simulink model "new_model"  (R2023a)
(part 3 of 4)

  Bus Selector:RadarSensor:1_OBJ_S_Range_BS/39 -> RadarSensor:1.OBJ_S_Range_39/1  "<OBJ_S_Range_39>"
  Bus Selector:RadarSensor:1_OBJ_S_Range_BS/40 -> RadarSensor:1.OBJ_S_Range_40/1  "<OBJ_S_Range_40>"
  Bus Selector:RadarSensor:1_OBJ_S_Range_BS/41 -> RadarSensor:1.OBJ_S_Range_41/1  "<OBJ_S_Range_41>"
  Bus Selector:RadarSensor:1_OBJ_S_Range_BS/42 -> RadarSensor:1.OBJ_S_Range_42/1  "<OBJ_S_Range_42>"
  Bus Selector:RadarSensor:1_OBJ_S_Range_BS/43 -> RadarSensor:1.OBJ_S_Range_43/1  "<OBJ_S_Range_43>"
  Bus Selector:RadarSensor:1_OBJ_S_Range_BS/44 -> RadarSensor:1.OBJ_S_Range_44/1  "<OBJ_S_Range_44>"
  Bus Selector:RadarSensor:1_OBJ_S_Range_BS/45 -> RadarSensor:1.OBJ_S_Range_45/1  "<OBJ_S_Range_45>"
  Bus Selector:RadarSensor:1_OBJ_S_Range_BS/46 -> RadarSensor:1.OBJ_S_Range_46/1  "<OBJ_S_Range_46>"
  Bus Selector:RadarSensor:1_OBJ_S_Range_BS/47 -> RadarSensor:1.OBJ_S_Range_47/1  "<OBJ_S_Range_47>"
  Bus Selector:RadarSensor:1_OBJ_S_Range_BS/48 -> RadarSensor:1.OBJ_S_Range_48/1  "<OBJ_S_Range_48>"
  Bus Selector:RadarSensor:1_OBJ_S_Range_BS/49 -> RadarSensor:1.OBJ_S_Range_49/1  "<OBJ_S_Range_49>"
  Bus Selector:RadarSensor:1_OBJ_S_Range_BS/50 -> RadarSensor:1.OBJ_S_Range_50/1  "<OBJ_S_Range_50>"
  Bus Selector:RadarSensor:1_OBJ_S_Range_BS/51 -> RadarSensor:1.OBJ_S_Range_51/1  "<OBJ_S_Range_51>"
  Bus Selector:RadarSensor:1_OBJ_S_Range_BS/52 -> RadarSensor:1.OBJ_S_Range_52/1  "<OBJ_S_Range_52>"
  Bus Selector:RadarSensor:1_OBJ_S_Range_BS/53 -> RadarSensor:1.OBJ_S_Range_53/1  "<OBJ_S_Range_53>"
  Bus Selector:RadarSensor:1_OBJ_S_Range_BS/54 -> RadarSensor:1.OBJ_S_Range_54/1  "<OBJ_S_Range_54>"
  Bus Selector:RadarSensor:1_OBJ_S_Range_BS/55 -> RadarSensor:1.OBJ_S_Range_55/1  "<OBJ_S_Range_55>"
  Bus Selector:RadarSensor:1_OBJ_S_Range_BS/56 -> RadarSensor:1.OBJ_S_Range_56/1  "<OBJ_S_Range_56>"
  Bus Selector:RadarSensor:1_OBJ_S_Range_BS/57 -> RadarSensor:1.OBJ_S_Range_57/1  "<OBJ_S_Range_57>"
  Bus Selector:RadarSensor:1_OBJ_S_Range_BS/58 -> RadarSensor:1.OBJ_S_Range_58/1  "<OBJ_S_Range_58>"
  Bus Selector:RadarSensor:1_OBJ_S_Range_BS/59 -> RadarSensor:1.OBJ_S_Range_59/1  "<OBJ_S_Range_59>"
  Bus Selector:RadarSensor:1_OBJ_S_Range_BS/60 -> RadarSensor:1.OBJ_S_Range_60/1  "<OBJ_S_Range_60>"
  Bus Selector:RadarSensor:1_OBJ_S_Range_BS/61 -> RadarSensor:1.OBJ_S_Range_61/1  "<OBJ_S_Range_61>"
  Bus Selector:RadarSensor:1_OBJ_S_Range_BS/62 -> RadarSensor:1.OBJ_S_Range_62/1  "<OBJ_S_Range_62>"
  Bus Selector:RadarSensor:1_OBJ_S_Range_BS/63 -> RadarSensor:1.OBJ_S_Range_63/1  "<OBJ_S_Range_63>"
  Bus Selector:RadarSensor:1_OBJ_S_Range_BS/64 -> RadarSensor:1.OBJ_S_Range_64/1  "<OBJ_S_Range_64>"
  Bus Selector:RadarSensor:1_OBJ_RCS_BS/1 -> RadarSensor:1.OBJ_RCS_1/1  "<OBJ_RCS_1>"
  Bus Selector:RadarSensor:1_OBJ_RCS_BS/2 -> RadarSensor:1.OBJ_RCS_2/1  "<OBJ_RCS_2>"
  Bus Selector:RadarSensor:1_OBJ_RCS_BS/3 -> RadarSensor:1.OBJ_RCS_3/1  "<OBJ_RCS_3>"
  Bus Selector:RadarSensor:1_OBJ_RCS_BS/4 -> RadarSensor:1.OBJ_RCS_4/1  "<OBJ_RCS_4>"
  Bus Selector:RadarSensor:1_OBJ_RCS_BS/5 -> RadarSensor:1.OBJ_RCS_5/1  "<OBJ_RCS_5>"
  Bus Selector:RadarSensor:1_OBJ_RCS_BS/6 -> RadarSensor:1.OBJ_RCS_6/1  "<OBJ_RCS_6>"
  Bus Selector:RadarSensor:1_OBJ_RCS_BS/7 -> RadarSensor:1.OBJ_RCS_7/1  "<OBJ_RCS_7>"
  Bus Selector:RadarSensor:1_OBJ_RCS_BS/8 -> RadarSensor:1.OBJ_RCS_8/1  "<OBJ_RCS_8>"
  Bus Selector:RadarSensor:1_OBJ_RCS_BS/9 -> RadarSensor:1.OBJ_RCS_9/1  "<OBJ_RCS_9>"
  Bus Selector:RadarSensor:1_OBJ_RCS_BS/10 -> RadarSensor:1.OBJ_RCS_10/1  "<OBJ_RCS_10>"
  Bus Selector:RadarSensor:1_OBJ_RCS_BS/11 -> RadarSensor:1.OBJ_RCS_11/1  "<OBJ_RCS_11>"
  Bus Selector:RadarSensor:1_OBJ_RCS_BS/12 -> RadarSensor:1.OBJ_RCS_12/1  "<OBJ_RCS_12>"
  Bus Selector:RadarSensor:1_OBJ_RCS_BS/13 -> RadarSensor:1.OBJ_RCS_13/1  "<OBJ_RCS_13>"
  Bus Selector:RadarSensor:1_OBJ_RCS_BS/14 -> RadarSensor:1.OBJ_RCS_14/1  "<OBJ_RCS_14>"
  Bus Selector:RadarSensor:1_OBJ_RCS_BS/15 -> RadarSensor:1.OBJ_RCS_15/1  "<OBJ_RCS_15>"
  Bus Selector:RadarSensor:1_OBJ_RCS_BS/16 -> RadarSensor:1.OBJ_RCS_16/1  "<OBJ_RCS_16>"
  Bus Selector:RadarSensor:1_OBJ_RCS_BS/17 -> RadarSensor:1.OBJ_RCS_17/1  "<OBJ_RCS_17>"
  Bus Selector:RadarSensor:1_OBJ_RCS_BS/18 -> RadarSensor:1.OBJ_RCS_18/1  "<OBJ_RCS_18>"
  Bus Selector:RadarSensor:1_OBJ_RCS_BS/19 -> RadarSensor:1.OBJ_RCS_19/1  "<OBJ_RCS_19>"
  Bus Selector:RadarSensor:1_OBJ_RCS_BS/20 -> RadarSensor:1.OBJ_RCS_20/1  "<OBJ_RCS_20>"
  Bus Selector:RadarSensor:1_OBJ_RCS_BS/21 -> RadarSensor:1.OBJ_RCS_21/1  "<OBJ_RCS_21>"
  Bus Selector:RadarSensor:1_OBJ_RCS_BS/22 -> RadarSensor:1.OBJ_RCS_22/1  "<OBJ_RCS_22>"
  Bus Selector:RadarSensor:1_OBJ_RCS_BS/23 -> RadarSensor:1.OBJ_RCS_23/1  "<OBJ_RCS_23>"
  Bus Selector:RadarSensor:1_OBJ_RCS_BS/24 -> RadarSensor:1.OBJ_RCS_24/1  "<OBJ_RCS_24>"
  Bus Selector:RadarSensor:1_OBJ_RCS_BS/25 -> RadarSensor:1.OBJ_RCS_25/1  "<OBJ_RCS_25>"
  Bus Selector:RadarSensor:1_OBJ_RCS_BS/26 -> RadarSensor:1.OBJ_RCS_26/1  "<OBJ_RCS_26>"
  Bus Selector:RadarSensor:1_OBJ_RCS_BS/27 -> RadarSensor:1.OBJ_RCS_27/1  "<OBJ_RCS_27>"
  Bus Selector:RadarSensor:1_OBJ_RCS_BS/28 -> RadarSensor:1.OBJ_RCS_28/1  "<OBJ_RCS_28>"
  Bus Selector:RadarSensor:1_OBJ_RCS_BS/29 -> RadarSensor:1.OBJ_RCS_29/1  "<OBJ_RCS_29>"
  Bus Selector:RadarSensor:1_OBJ_RCS_BS/30 -> RadarSensor:1.OBJ_RCS_30/1  "<OBJ_RCS_30>"
  Bus Selector:RadarSensor:1_OBJ_RCS_BS/31 -> RadarSensor:1.OBJ_RCS_31/1  "<OBJ_RCS_31>"
  Bus Selector:RadarSensor:1_OBJ_RCS_BS/32 -> RadarSensor:1.OBJ_RCS_32/1  "<OBJ_RCS_32>"
  Bus Selector:RadarSensor:1_OBJ_RCS_BS/33 -> RadarSensor:1.OBJ_RCS_33/1  "<OBJ_RCS_33>"
  Bus Selector:RadarSensor:1_OBJ_RCS_BS/34 -> RadarSensor:1.OBJ_RCS_34/1  "<OBJ_RCS_34>"
  Bus Selector:RadarSensor:1_OBJ_RCS_BS/35 -> RadarSensor:1.OBJ_RCS_35/1  "<OBJ_RCS_35>"
  Bus Selector:RadarSensor:1_OBJ_RCS_BS/36 -> RadarSensor:1.OBJ_RCS_36/1  "<OBJ_RCS_36>"
  Bus Selector:RadarSensor:1_OBJ_RCS_BS/37 -> RadarSensor:1.OBJ_RCS_37/1  "<OBJ_RCS_37>"
  Bus Selector:RadarSensor:1_OBJ_RCS_BS/38 -> RadarSensor:1.OBJ_RCS_38/1  "<OBJ_RCS_38>"
  Bus Selector:RadarSensor:1_OBJ_RCS_BS/39 -> RadarSensor:1.OBJ_RCS_39/1  "<OBJ_RCS_39>"
  Bus Selector:RadarSensor:1_OBJ_RCS_BS/40 -> RadarSensor:1.OBJ_RCS_40/1  "<OBJ_RCS_40>"
  Bus Selector:RadarSensor:1_OBJ_RCS_BS/41 -> RadarSensor:1.OBJ_RCS_41/1  "<OBJ_RCS_41>"
  Bus Selector:RadarSensor:1_OBJ_RCS_BS/42 -> RadarSensor:1.OBJ_RCS_42/1  "<OBJ_RCS_42>"
  Bus Selector:RadarSensor:1_OBJ_RCS_BS/43 -> RadarSensor:1.OBJ_RCS_43/1  "<OBJ_RCS_43>"
  Bus Selector:RadarSensor:1_OBJ_RCS_BS/44 -> RadarSensor:1.OBJ_RCS_44/1  "<OBJ_RCS_44>"
  Bus Selector:RadarSensor:1_OBJ_RCS_BS/45 -> RadarSensor:1.OBJ_RCS_45/1  "<OBJ_RCS_45>"
  Bus Selector:RadarSensor:1_OBJ_RCS_BS/46 -> RadarSensor:1.OBJ_RCS_46/1  "<OBJ_RCS_46>"
  Bus Selector:RadarSensor:1_OBJ_RCS_BS/47 -> RadarSensor:1.OBJ_RCS_47/1  "<OBJ_RCS_47>"
  Bus Selector:RadarSensor:1_OBJ_RCS_BS/48 -> RadarSensor:1.OBJ_RCS_48/1  "<OBJ_RCS_48>"
  Bus Selector:RadarSensor:1_OBJ_RCS_BS/49 -> RadarSensor:1.OBJ_RCS_49/1  "<OBJ_RCS_49>"
  Bus Selector:RadarSensor:1_OBJ_RCS_BS/50 -> RadarSensor:1.OBJ_RCS_50/1  "<OBJ_RCS_50>"
  Bus Selector:RadarSensor:1_OBJ_RCS_BS/51 -> RadarSensor:1.OBJ_RCS_51/1  "<OBJ_RCS_51>"
  Bus Selector:RadarSensor:1_OBJ_RCS_BS/52 -> RadarSensor:1.OBJ_RCS_52/1  "<OBJ_RCS_52>"
  Bus Selector:RadarSensor:1_OBJ_RCS_BS/53 -> RadarSensor:1.OBJ_RCS_53/1  "<OBJ_RCS_53>"
  Bus Selector:RadarSensor:1_OBJ_RCS_BS/54 -> RadarSensor:1.OBJ_RCS_54/1  "<OBJ_RCS_54>"
  Bus Selector:RadarSensor:1_OBJ_RCS_BS/55 -> RadarSensor:1.OBJ_RCS_55/1  "<OBJ_RCS_55>"
  Bus Selector:RadarSensor:1_OBJ_RCS_BS/56 -> RadarSensor:1.OBJ_RCS_56/1  "<OBJ_RCS_56>"
  Bus Selector:RadarSensor:1_OBJ_RCS_BS/57 -> RadarSensor:1.OBJ_RCS_57/1  "<OBJ_RCS_57>"
  Bus Selector:RadarSensor:1_OBJ_RCS_BS/58 -> RadarSensor:1.OBJ_RCS_58/1  "<OBJ_RCS_58>"
  Bus Selector:RadarSensor:1_OBJ_RCS_BS/59 -> RadarSensor:1.OBJ_RCS_59/1  "<OBJ_RCS_59>"
  Bus Selector:RadarSensor:1_OBJ_RCS_BS/60 -> RadarSensor:1.OBJ_RCS_60/1  "<OBJ_RCS_60>"
  Bus Selector:RadarSensor:1_OBJ_RCS_BS/61 -> RadarSensor:1.OBJ_RCS_61/1  "<OBJ_RCS_61>"
  Bus Selector:RadarSensor:1_OBJ_RCS_BS/62 -> RadarSensor:1.OBJ_RCS_62/1  "<OBJ_RCS_62>"
  Bus Selector:RadarSensor:1_OBJ_RCS_BS/63 -> RadarSensor:1.OBJ_RCS_63/1  "<OBJ_RCS_63>"
  Bus Selector:RadarSensor:1_OBJ_RCS_BS/64 -> RadarSensor:1.OBJ_RCS_64/1  "<OBJ_RCS_64>"
  Bus Selector:RadarSensor:1/1 -> RadarSensor:1.time/1  "<time>"
  Bus Selector:RadarSensor:1/2 -> RadarSensor:1.width/1  "<width>"
  Bus Selector:RadarSensor:1/3 -> RadarSensor:1.OBJ_ID/1, Bus Selector:RadarSensor:1_OBJ_ID_BS/1  "<OBJ_ID>"
  Bus Selector:RadarSensor:1/4 -> RadarSensor:1.OBJ_Class/1, Bus Selector:RadarSensor:1_OBJ_Class_BS/1  "<OBJ_Class>"
  Bus Selector:RadarSensor:1/5 -> RadarSensor:1.OBJ_S_Azimuth/1, Bus Selector:RadarSensor:1_OBJ_S_Azimuth_BS/1  "<OBJ_S_Azimuth>"
  Bus Selector:RadarSensor:1/6 -> RadarSensor:1.OBJ_S_Elevation/1, Bus Selector:RadarSensor:1_OBJ_S_Elevation_BS/1  "<OBJ_S_Elevation>"
  Bus Selector:RadarSensor:1/7 -> RadarSensor:1.OBJ_S_Velocity/1, Bus Selector:RadarSensor:1_OBJ_S_Velocity_BS/1  "<OBJ_S_Velocity>"
  Bus Selector:RadarSensor:1/8 -> RadarSensor:1.OBJ_S_Range/1, Bus Selector:RadarSensor:1_OBJ_S_Range_BS/1  "<OBJ_S_Range>"
  Bus Selector:RadarSensor:1/9 -> RadarSensor:1.OBJ_RCS/1, Bus Selector:RadarSensor:1_OBJ_RCS_BS/1  "<OBJ_RCS>"
  Bus Selector:RadarSensor:2_OBJ_ID_BS/1 -> RadarSensor:2.OBJ_ID_1/1  "<OBJ_ID_1>"
  Bus Selector:RadarSensor:2_OBJ_ID_BS/2 -> RadarSensor:2.OBJ_ID_2/1  "<OBJ_ID_2>"
  Bus Selector:RadarSensor:2_OBJ_ID_BS/3 -> RadarSensor:2.OBJ_ID_3/1  "<OBJ_ID_3>"
  Bus Selector:RadarSensor:2_OBJ_ID_BS/4 -> RadarSensor:2.OBJ_ID_4/1  "<OBJ_ID_4>"
  Bus Selector:RadarSensor:2_OBJ_ID_BS/5 -> RadarSensor:2.OBJ_ID_5/1  "<OBJ_ID_5>"
  Bus Selector:RadarSensor:2_OBJ_ID_BS/6 -> RadarSensor:2.OBJ_ID_6/1  "<OBJ_ID_6>"
  Bus Selector:RadarSensor:2_OBJ_ID_BS/7 -> RadarSensor:2.OBJ_ID_7/1  "<OBJ_ID_7>"
  Bus Selector:RadarSensor:2_OBJ_ID_BS/8 -> RadarSensor:2.OBJ_ID_8/1  "<OBJ_ID_8>"
  Bus Selector:RadarSensor:2_OBJ_ID_BS/9 -> RadarSensor:2.OBJ_ID_9/1  "<OBJ_ID_9>"
  Bus Selector:RadarSensor:2_OBJ_ID_BS/10 -> RadarSensor:2.OBJ_ID_10/1  "<OBJ_ID_10>"
  Bus Selector:RadarSensor:2_OBJ_ID_BS/11 -> RadarSensor:2.OBJ_ID_11/1  "<OBJ_ID_11>"
  Bus Selector:RadarSensor:2_OBJ_ID_BS/12 -> RadarSensor:2.OBJ_ID_12/1  "<OBJ_ID_12>"
  Bus Selector:RadarSensor:2_OBJ_ID_BS/13 -> RadarSensor:2.OBJ_ID_13/1  "<OBJ_ID_13>"
  Bus Selector:RadarSensor:2_OBJ_ID_BS/14 -> RadarSensor:2.OBJ_ID_14/1  "<OBJ_ID_14>"
  Bus Selector:RadarSensor:2_OBJ_ID_BS/15 -> RadarSensor:2.OBJ_ID_15/1  "<OBJ_ID_15>"
  Bus Selector:RadarSensor:2_OBJ_ID_BS/16 -> RadarSensor:2.OBJ_ID_16/1  "<OBJ_ID_16>"
  Bus Selector:RadarSensor:2_OBJ_ID_BS/17 -> RadarSensor:2.OBJ_ID_17/1  "<OBJ_ID_17>"
  Bus Selector:RadarSensor:2_OBJ_ID_BS/18 -> RadarSensor:2.OBJ_ID_18/1  "<OBJ_ID_18>"
  Bus Selector:RadarSensor:2_OBJ_ID_BS/19 -> RadarSensor:2.OBJ_ID_19/1  "<OBJ_ID_19>"
  Bus Selector:RadarSensor:2_OBJ_ID_BS/20 -> RadarSensor:2.OBJ_ID_20/1  "<OBJ_ID_20>"
  Bus Selector:RadarSensor:2_OBJ_ID_BS/21 -> RadarSensor:2.OBJ_ID_21/1  "<OBJ_ID_21>"
  Bus Selector:RadarSensor:2_OBJ_ID_BS/22 -> RadarSensor:2.OBJ_ID_22/1  "<OBJ_ID_22>"
  Bus Selector:RadarSensor:2_OBJ_ID_BS/23 -> RadarSensor:2.OBJ_ID_23/1  "<OBJ_ID_23>"
  Bus Selector:RadarSensor:2_OBJ_ID_BS/24 -> RadarSensor:2.OBJ_ID_24/1  "<OBJ_ID_24>"
  Bus Selector:RadarSensor:2_OBJ_ID_BS/25 -> RadarSensor:2.OBJ_ID_25/1  "<OBJ_ID_25>"
  Bus Selector:RadarSensor:2_OBJ_ID_BS/26 -> RadarSensor:2.OBJ_ID_26/1  "<OBJ_ID_26>"
  Bus Selector:RadarSensor:2_OBJ_ID_BS/27 -> RadarSensor:2.OBJ_ID_27/1  "<OBJ_ID_27>"
  Bus Selector:RadarSensor:2_OBJ_ID_BS/28 -> RadarSensor:2.OBJ_ID_28/1  "<OBJ_ID_28>"
  Bus Selector:RadarSensor:2_OBJ_ID_BS/29 -> RadarSensor:2.OBJ_ID_29/1  "<OBJ_ID_29>"
  Bus Selector:RadarSensor:2_OBJ_ID_BS/30 -> RadarSensor:2.OBJ_ID_30/1  "<OBJ_ID_30>"
  Bus Selector:RadarSensor:2_OBJ_ID_BS/31 -> RadarSensor:2.OBJ_ID_31/1  "<OBJ_ID_31>"
  Bus Selector:RadarSensor:2_OBJ_ID_BS/32 -> RadarSensor:2.OBJ_ID_32/1  "<OBJ_ID_32>"
  Bus Selector:RadarSensor:2_OBJ_ID_BS/33 -> RadarSensor:2.OBJ_ID_33/1  "<OBJ_ID_33>"
  Bus Selector:RadarSensor:2_OBJ_ID_BS/34 -> RadarSensor:2.OBJ_ID_34/1  "<OBJ_ID_34>"
  Bus Selector:RadarSensor:2_OBJ_ID_BS/35 -> RadarSensor:2.OBJ_ID_35/1  "<OBJ_ID_35>"
  Bus Selector:RadarSensor:2_OBJ_ID_BS/36 -> RadarSensor:2.OBJ_ID_36/1  "<OBJ_ID_36>"
  Bus Selector:RadarSensor:2_OBJ_ID_BS/37 -> RadarSensor:2.OBJ_ID_37/1  "<OBJ_ID_37>"
  Bus Selector:RadarSensor:2_OBJ_ID_BS/38 -> RadarSensor:2.OBJ_ID_38/1  "<OBJ_ID_38>"
  Bus Selector:RadarSensor:2_OBJ_ID_BS/39 -> RadarSensor:2.OBJ_ID_39/1  "<OBJ_ID_39>"
  Bus Selector:RadarSensor:2_OBJ_ID_BS/40 -> RadarSensor:2.OBJ_ID_40/1  "<OBJ_ID_40>"
  Bus Selector:RadarSensor:2_OBJ_ID_BS/41 -> RadarSensor:2.OBJ_ID_41/1  "<OBJ_ID_41>"
  Bus Selector:RadarSensor:2_OBJ_ID_BS/42 -> RadarSensor:2.OBJ_ID_42/1  "<OBJ_ID_42>"
  Bus Selector:RadarSensor:2_OBJ_ID_BS/43 -> RadarSensor:2.OBJ_ID_43/1  "<OBJ_ID_43>"
  Bus Selector:RadarSensor:2_OBJ_ID_BS/44 -> RadarSensor:2.OBJ_ID_44/1  "<OBJ_ID_44>"
  Bus Selector:RadarSensor:2_OBJ_ID_BS/45 -> RadarSensor:2.OBJ_ID_45/1  "<OBJ_ID_45>"
  Bus Selector:RadarSensor:2_OBJ_ID_BS/46 -> RadarSensor:2.OBJ_ID_46/1  "<OBJ_ID_46>"
  Bus Selector:RadarSensor:2_OBJ_ID_BS/47 -> RadarSensor:2.OBJ_ID_47/1  "<OBJ_ID_47>"
  Bus Selector:RadarSensor:2_OBJ_ID_BS/48 -> RadarSensor:2.OBJ_ID_48/1  "<OBJ_ID_48>"
  Bus Selector:RadarSensor:2_OBJ_ID_BS/49 -> RadarSensor:2.OBJ_ID_49/1  "<OBJ_ID_49>"
  Bus Selector:RadarSensor:2_OBJ_ID_BS/50 -> RadarSensor:2.OBJ_ID_50/1  "<OBJ_ID_50>"
  Bus Selector:RadarSensor:2_OBJ_ID_BS/51 -> RadarSensor:2.OBJ_ID_51/1  "<OBJ_ID_51>"
  Bus Selector:RadarSensor:2_OBJ_ID_BS/52 -> RadarSensor:2.OBJ_ID_52/1  "<OBJ_ID_52>"
  Bus Selector:RadarSensor:2_OBJ_ID_BS/53 -> RadarSensor:2.OBJ_ID_53/1  "<OBJ_ID_53>"
  Bus Selector:RadarSensor:2_OBJ_ID_BS/54 -> RadarSensor:2.OBJ_ID_54/1  "<OBJ_ID_54>"
  Bus Selector:RadarSensor:2_OBJ_ID_BS/55 -> RadarSensor:2.OBJ_ID_55/1  "<OBJ_ID_55>"
  Bus Selector:RadarSensor:2_OBJ_ID_BS/56 -> RadarSensor:2.OBJ_ID_56/1  "<OBJ_ID_56>"
  Bus Selector:RadarSensor:2_OBJ_ID_BS/57 -> RadarSensor:2.OBJ_ID_57/1  "<OBJ_ID_57>"
  Bus Selector:RadarSensor:2_OBJ_ID_BS/58 -> RadarSensor:2.OBJ_ID_58/1  "<OBJ_ID_58>"
  Bus Selector:RadarSensor:2_OBJ_ID_BS/59 -> RadarSensor:2.OBJ_ID_59/1  "<OBJ_ID_59>"
  Bus Selector:RadarSensor:2_OBJ_ID_BS/60 -> RadarSensor:2.OBJ_ID_60/1  "<OBJ_ID_60>"
  Bus Selector:RadarSensor:2_OBJ_ID_BS/61 -> RadarSensor:2.OBJ_ID_61/1  "<OBJ_ID_61>"
  Bus Selector:RadarSensor:2_OBJ_ID_BS/62 -> RadarSensor:2.OBJ_ID_62/1  "<OBJ_ID_62>"
  Bus Selector:RadarSensor:2_OBJ_ID_BS/63 -> RadarSensor:2.OBJ_ID_63/1  "<OBJ_ID_63>"
  Bus Selector:RadarSensor:2_OBJ_ID_BS/64 -> RadarSensor:2.OBJ_ID_64/1  "<OBJ_ID_64>"
  Bus Selector:RadarSensor:2_OBJ_Class_BS/1 -> RadarSensor:2.OBJ_Class_1/1  "<OBJ_Class_1>"
  Bus Selector:RadarSensor:2_OBJ_Class_BS/2 -> RadarSensor:2.OBJ_Class_2/1  "<OBJ_Class_2>"
  Bus Selector:RadarSensor:2_OBJ_Class_BS/3 -> RadarSensor:2.OBJ_Class_3/1  "<OBJ_Class_3>"
  Bus Selector:RadarSensor:2_OBJ_Class_BS/4 -> RadarSensor:2.OBJ_Class_4/1  "<OBJ_Class_4>"
  Bus Selector:RadarSensor:2_OBJ_Class_BS/5 -> RadarSensor:2.OBJ_Class_5/1  "<OBJ_Class_5>"
  Bus Selector:RadarSensor:2_OBJ_Class_BS/6 -> RadarSensor:2.OBJ_Class_6/1  "<OBJ_Class_6>"
  Bus Selector:RadarSensor:2_OBJ_Class_BS/7 -> RadarSensor:2.OBJ_Class_7/1  "<OBJ_Class_7>"
  Bus Selector:RadarSensor:2_OBJ_Class_BS/8 -> RadarSensor:2.OBJ_Class_8/1  "<OBJ_Class_8>"
  Bus Selector:RadarSensor:2_OBJ_Class_BS/9 -> RadarSensor:2.OBJ_Class_9/1  "<OBJ_Class_9>"
  Bus Selector:RadarSensor:2_OBJ_Class_BS/10 -> RadarSensor:2.OBJ_Class_10/1  "<OBJ_Class_10>"
  Bus Selector:RadarSensor:2_OBJ_Class_BS/11 -> RadarSensor:2.OBJ_Class_11/1  "<OBJ_Class_11>"
  Bus Selector:RadarSensor:2_OBJ_Class_BS/12 -> RadarSensor:2.OBJ_Class_12/1  "<OBJ_Class_12>"
  Bus Selector:RadarSensor:2_OBJ_Class_BS/13 -> RadarSensor:2.OBJ_Class_13/1  "<OBJ_Class_13>"
  Bus Selector:RadarSensor:2_OBJ_Class_BS/14 -> RadarSensor:2.OBJ_Class_14/1  "<OBJ_Class_14>"
  Bus Selector:RadarSensor:2_OBJ_Class_BS/15 -> RadarSensor:2.OBJ_Class_15/1  "<OBJ_Class_15>"
  Bus Selector:RadarSensor:2_OBJ_Class_BS/16 -> RadarSensor:2.OBJ_Class_16/1  "<OBJ_Class_16>"
  Bus Selector:RadarSensor:2_OBJ_Class_BS/17 -> RadarSensor:2.OBJ_Class_17/1  "<OBJ_Class_17>"
  Bus Selector:RadarSensor:2_OBJ_Class_BS/18 -> RadarSensor:2.OBJ_Class_18/1  "<OBJ_Class_18>"
  Bus Selector:RadarSensor:2_OBJ_Class_BS/19 -> RadarSensor:2.OBJ_Class_19/1  "<OBJ_Class_19>"
  Bus Selector:RadarSensor:2_OBJ_Class_BS/20 -> RadarSensor:2.OBJ_Class_20/1  "<OBJ_Class_20>"
  Bus Selector:RadarSensor:2_OBJ_Class_BS/21 -> RadarSensor:2.OBJ_Class_21/1  "<OBJ_Class_21>"
  Bus Selector:RadarSensor:2_OBJ_Class_BS/22 -> RadarSensor:2.OBJ_Class_22/1  "<OBJ_Class_22>"
  Bus Selector:RadarSensor:2_OBJ_Class_BS/23 -> RadarSensor:2.OBJ_Class_23/1  "<OBJ_Class_23>"
  Bus Selector:RadarSensor:2_OBJ_Class_BS/24 -> RadarSensor:2.OBJ_Class_24/1  "<OBJ_Class_24>"
  Bus Selector:RadarSensor:2_OBJ_Class_BS/25 -> RadarSensor:2.OBJ_Class_25/1  "<OBJ_Class_25>"
  Bus Selector:RadarSensor:2_OBJ_Class_BS/26 -> RadarSensor:2.OBJ_Class_26/1  "<OBJ_Class_26>"
  Bus Selector:RadarSensor:2_OBJ_Class_BS/27 -> RadarSensor:2.OBJ_Class_27/1  "<OBJ_Class_27>"
  Bus Selector:RadarSensor:2_OBJ_Class_BS/28 -> RadarSensor:2.OBJ_Class_28/1  "<OBJ_Class_28>"
  Bus Selector:RadarSensor:2_OBJ_Class_BS/29 -> RadarSensor:2.OBJ_Class_29/1  "<OBJ_Class_29>"
  Bus Selector:RadarSensor:2_OBJ_Class_BS/30 -> RadarSensor:2.OBJ_Class_30/1  "<OBJ_Class_30>"
  Bus Selector:RadarSensor:2_OBJ_Class_BS/31 -> RadarSensor:2.OBJ_Class_31/1  "<OBJ_Class_31>"
  Bus Selector:RadarSensor:2_OBJ_Class_BS/32 -> RadarSensor:2.OBJ_Class_32/1  "<OBJ_Class_32>"
  Bus Selector:RadarSensor:2_OBJ_Class_BS/33 -> RadarSensor:2.OBJ_Class_33/1  "<OBJ_Class_33>"
  Bus Selector:RadarSensor:2_OBJ_Class_BS/34 -> RadarSensor:2.OBJ_Class_34/1  "<OBJ_Class_34>"
  Bus Selector:RadarSensor:2_OBJ_Class_BS/35 -> RadarSensor:2.OBJ_Class_35/1  "<OBJ_Class_35>"
  Bus Selector:RadarSensor:2_OBJ_Class_BS/36 -> RadarSensor:2.OBJ_Class_36/1  "<OBJ_Class_36>"
  Bus Selector:RadarSensor:2_OBJ_Class_BS/37 -> RadarSensor:2.OBJ_Class_37/1  "<OBJ_Class_37>"
  Bus Selector:RadarSensor:2_OBJ_Class_BS/38 -> RadarSensor:2.OBJ_Class_38/1  "<OBJ_Class_38>"
  Bus Selector:RadarSensor:2_OBJ_Class_BS/39 -> RadarSensor:2.OBJ_Class_39/1  "<OBJ_Class_39>"
  Bus Selector:RadarSensor:2_OBJ_Class_BS/40 -> RadarSensor:2.OBJ_Class_40/1  "<OBJ_Class_40>"
  Bus Selector:RadarSensor:2_OBJ_Class_BS/41 -> RadarSensor:2.OBJ_Class_41/1  "<OBJ_Class_41>"
  Bus Selector:RadarSensor:2_OBJ_Class_BS/42 -> RadarSensor:2.OBJ_Class_42/1  "<OBJ_Class_42>"
  Bus Selector:RadarSensor:2_OBJ_Class_BS/43 -> RadarSensor:2.OBJ_Class_43/1  "<OBJ_Class_43>"
  Bus Selector:RadarSensor:2_OBJ_Class_BS/44 -> RadarSensor:2.OBJ_Class_44/1  "<OBJ_Class_44>"
  Bus Selector:RadarSensor:2_OBJ_Class_BS/45 -> RadarSensor:2.OBJ_Class_45/1  "<OBJ_Class_45>"
  Bus Selector:RadarSensor:2_OBJ_Class_BS/46 -> RadarSensor:2.OBJ_Class_46/1  "<OBJ_Class_46>"
  Bus Selector:RadarSensor:2_OBJ_Class_BS/47 -> RadarSensor:2.OBJ_Class_47/1  "<OBJ_Class_47>"
  Bus Selector:RadarSensor:2_OBJ_Class_BS/48 -> RadarSensor:2.OBJ_Class_48/1  "<OBJ_Class_48>"
  Bus Selector:RadarSensor:2_OBJ_Class_BS/49 -> RadarSensor:2.OBJ_Class_49/1  "<OBJ_Class_49>"
  Bus Selector:RadarSensor:2_OBJ_Class_BS/50 -> RadarSensor:2.OBJ_Class_50/1  "<OBJ_Class_50>"
  Bus Selector:RadarSensor:2_OBJ_Class_BS/51 -> RadarSensor:2.OBJ_Class_51/1  "<OBJ_Class_51>"
  Bus Selector:RadarSensor:2_OBJ_Class_BS/52 -> RadarSensor:2.OBJ_Class_52/1  "<OBJ_Class_52>"
  Bus Selector:RadarSensor:2_OBJ_Class_BS/53 -> RadarSensor:2.OBJ_Class_53/1  "<OBJ_Class_53>"
  Bus Selector:RadarSensor:2_OBJ_Class_BS/54 -> RadarSensor:2.OBJ_Class_54/1  "<OBJ_Class_54>"
  Bus Selector:RadarSensor:2_OBJ_Class_BS/55 -> RadarSensor:2.OBJ_Class_55/1  "<OBJ_Class_55>"
  Bus Selector:RadarSensor:2_OBJ_Class_BS/56 -> RadarSensor:2.OBJ_Class_56/1  "<OBJ_Class_56>"
  Bus Selector:RadarSensor:2_OBJ_Class_BS/57 -> RadarSensor:2.OBJ_Class_57/1  "<OBJ_Class_57>"
  Bus Selector:RadarSensor:2_OBJ_Class_BS/58 -> RadarSensor:2.OBJ_Class_58/1  "<OBJ_Class_58>"
  Bus Selector:RadarSensor:2_OBJ_Class_BS/59 -> RadarSensor:2.OBJ_Class_59/1  "<OBJ_Class_59>"
  Bus Selector:RadarSensor:2_OBJ_Class_BS/60 -> RadarSensor:2.OBJ_Class_60/1  "<OBJ_Class_60>"
  Bus Selector:RadarSensor:2_OBJ_Class_BS/61 -> RadarSensor:2.OBJ_Class_61/1  "<OBJ_Class_61>"
  Bus Selector:RadarSensor:2_OBJ_Class_BS/62 -> RadarSensor:2.OBJ_Class_62/1  "<OBJ_Class_62>"
  Bus Selector:RadarSensor:2_OBJ_Class_BS/63 -> RadarSensor:2.OBJ_Class_63/1  "<OBJ_Class_63>"
  Bus Selector:RadarSensor:2_OBJ_Class_BS/64 -> RadarSensor:2.OBJ_Class_64/1  "<OBJ_Class_64>"
  Bus Selector:RadarSensor:2_OBJ_S_Azimuth_BS/1 -> RadarSensor:2.OBJ_S_Azimuth_1/1  "<OBJ_S_Azimuth_1>"
  Bus Selector:RadarSensor:2_OBJ_S_Azimuth_BS/2 -> RadarSensor:2.OBJ_S_Azimuth_2/1  "<OBJ_S_Azimuth_2>"
  Bus Selector:RadarSensor:2_OBJ_S_Azimuth_BS/3 -> RadarSensor:2.OBJ_S_Azimuth_3/1  "<OBJ_S_Azimuth_3>"
  Bus Selector:RadarSensor:2_OBJ_S_Azimuth_BS/4 -> RadarSensor:2.OBJ_S_Azimuth_4/1  "<OBJ_S_Azimuth_4>"
  Bus Selector:RadarSensor:2_OBJ_S_Azimuth_BS/5 -> RadarSensor:2.OBJ_S_Azimuth_5/1  "<OBJ_S_Azimuth_5>"
  Bus Selector:RadarSensor:2_OBJ_S_Azimuth_BS/6 -> RadarSensor:2.OBJ_S_Azimuth_6/1  "<OBJ_S_Azimuth_6>"
  Bus Selector:RadarSensor:2_OBJ_S_Azimuth_BS/7 -> RadarSensor:2.OBJ_S_Azimuth_7/1  "<OBJ_S_Azimuth_7>"
  Bus Selector:RadarSensor:2_OBJ_S_Azimuth_BS/8 -> RadarSensor:2.OBJ_S_Azimuth_8/1  "<OBJ_S_Azimuth_8>"
  Bus Selector:RadarSensor:2_OBJ_S_Azimuth_BS/9 -> RadarSensor:2.OBJ_S_Azimuth_9/1  "<OBJ_S_Azimuth_9>"
  Bus Selector:RadarSensor:2_OBJ_S_Azimuth_BS/10 -> RadarSensor:2.OBJ_S_Azimuth_10/1  "<OBJ_S_Azimuth_10>"
  Bus Selector:RadarSensor:2_OBJ_S_Azimuth_BS/11 -> RadarSensor:2.OBJ_S_Azimuth_11/1  "<OBJ_S_Azimuth_11>"
  Bus Selector:RadarSensor:2_OBJ_S_Azimuth_BS/12 -> RadarSensor:2.OBJ_S_Azimuth_12/1  "<OBJ_S_Azimuth_12>"
  Bus Selector:RadarSensor:2_OBJ_S_Azimuth_BS/13 -> RadarSensor:2.OBJ_S_Azimuth_13/1  "<OBJ_S_Azimuth_13>"
  Bus Selector:RadarSensor:2_OBJ_S_Azimuth_BS/14 -> RadarSensor:2.OBJ_S_Azimuth_14/1  "<OBJ_S_Azimuth_14>"
  Bus Selector:RadarSensor:2_OBJ_S_Azimuth_BS/15 -> RadarSensor:2.OBJ_S_Azimuth_15/1  "<OBJ_S_Azimuth_15>"
  Bus Selector:RadarSensor:2_OBJ_S_Azimuth_BS/16 -> RadarSensor:2.OBJ_S_Azimuth_16/1  "<OBJ_S_Azimuth_16>"
  Bus Selector:RadarSensor:2_OBJ_S_Azimuth_BS/17 -> RadarSensor:2.OBJ_S_Azimuth_17/1  "<OBJ_S_Azimuth_17>"
  Bus Selector:RadarSensor:2_OBJ_S_Azimuth_BS/18 -> RadarSensor:2.OBJ_S_Azimuth_18/1  "<OBJ_S_Azimuth_18>"
  Bus Selector:RadarSensor:2_OBJ_S_Azimuth_BS/19 -> RadarSensor:2.OBJ_S_Azimuth_19/1  "<OBJ_S_Azimuth_19>"
  Bus Selector:RadarSensor:2_OBJ_S_Azimuth_BS/20 -> RadarSensor:2.OBJ_S_Azimuth_20/1  "<OBJ_S_Azimuth_20>"
  Bus Selector:RadarSensor:2_OBJ_S_Azimuth_BS/21 -> RadarSensor:2.OBJ_S_Azimuth_21/1  "<OBJ_S_Azimuth_21>"
  Bus Selector:RadarSensor:2_OBJ_S_Azimuth_BS/22 -> RadarSensor:2.OBJ_S_Azimuth_22/1  "<OBJ_S_Azimuth_22>"
  Bus Selector:RadarSensor:2_OBJ_S_Azimuth_BS/23 -> RadarSensor:2.OBJ_S_Azimuth_23/1  "<OBJ_S_Azimuth_23>"
  Bus Selector:RadarSensor:2_OBJ_S_Azimuth_BS/24 -> RadarSensor:2.OBJ_S_Azimuth_24/1  "<OBJ_S_Azimuth_24>"
  Bus Selector:RadarSensor:2_OBJ_S_Azimuth_BS/25 -> RadarSensor:2.OBJ_S_Azimuth_25/1  "<OBJ_S_Azimuth_25>"
  Bus Selector:RadarSensor:2_OBJ_S_Azimuth_BS/26 -> RadarSensor:2.OBJ_S_Azimuth_26/1  "<OBJ_S_Azimuth_26>"
  Bus Selector:RadarSensor:2_OBJ_S_Azimuth_BS/27 -> RadarSensor:2.OBJ_S_Azimuth_27/1  "<OBJ_S_Azimuth_27>"
  Bus Selector:RadarSensor:2_OBJ_S_Azimuth_BS/28 -> RadarSensor:2.OBJ_S_Azimuth_28/1  "<OBJ_S_Azimuth_28>"
  Bus Selector:RadarSensor:2_OBJ_S_Azimuth_BS/29 -> RadarSensor:2.OBJ_S_Azimuth_29/1  "<OBJ_S_Azimuth_29>"
  Bus Selector:RadarSensor:2_OBJ_S_Azimuth_BS/30 -> RadarSensor:2.OBJ_S_Azimuth_30/1  "<OBJ_S_Azimuth_30>"
  Bus Selector:RadarSensor:2_OBJ_S_Azimuth_BS/31 -> RadarSensor:2.OBJ_S_Azimuth_31/1  "<OBJ_S_Azimuth_31>"
  Bus Selector:RadarSensor:2_OBJ_S_Azimuth_BS/32 -> RadarSensor:2.OBJ_S_Azimuth_32/1  "<OBJ_S_Azimuth_32>"
  Bus Selector:RadarSensor:2_OBJ_S_Azimuth_BS/33 -> RadarSensor:2.OBJ_S_Azimuth_33/1  "<OBJ_S_Azimuth_33>"
  Bus Selector:RadarSensor:2_OBJ_S_Azimuth_BS/34 -> RadarSensor:2.OBJ_S_Azimuth_34/1  "<OBJ_S_Azimuth_34>"
  Bus Selector:RadarSensor:2_OBJ_S_Azimuth_BS/35 -> RadarSensor:2.OBJ_S_Azimuth_35/1  "<OBJ_S_Azimuth_35>"
  Bus Selector:RadarSensor:2_OBJ_S_Azimuth_BS/36 -> RadarSensor:2.OBJ_S_Azimuth_36/1  "<OBJ_S_Azimuth_36>"
  Bus Selector:RadarSensor:2_OBJ_S_Azimuth_BS/37 -> RadarSensor:2.OBJ_S_Azimuth_37/1  "<OBJ_S_Azimuth_37>"
  Bus Selector:RadarSensor:2_OBJ_S_Azimuth_BS/38 -> RadarSensor:2.OBJ_S_Azimuth_38/1  "<OBJ_S_Azimuth_38>"
  Bus Selector:RadarSensor:2_OBJ_S_Azimuth_BS/39 -> RadarSensor:2.OBJ_S_Azimuth_39/1  "<OBJ_S_Azimuth_39>"
  Bus Selector:RadarSensor:2_OBJ_S_Azimuth_BS/40 -> RadarSensor:2.OBJ_S_Azimuth_40/1  "<OBJ_S_Azimuth_40>"
  Bus Selector:RadarSensor:2_OBJ_S_Azimuth_BS/41 -> RadarSensor:2.OBJ_S_Azimuth_41/1  "<OBJ_S_Azimuth_41>"
  Bus Selector:RadarSensor:2_OBJ_S_Azimuth_BS/42 -> RadarSensor:2.OBJ_S_Azimuth_42/1  "<OBJ_S_Azimuth_42>"
  Bus Selector:RadarSensor:2_OBJ_S_Azimuth_BS/43 -> RadarSensor:2.OBJ_S_Azimuth_43/1  "<OBJ_S_Azimuth_43>"
  Bus Selector:RadarSensor:2_OBJ_S_Azimuth_BS/44 -> RadarSensor:2.OBJ_S_Azimuth_44/1  "<OBJ_S_Azimuth_44>"
  Bus Selector:RadarSensor:2_OBJ_S_Azimuth_BS/45 -> RadarSensor:2.OBJ_S_Azimuth_45/1  "<OBJ_S_Azimuth_45>"
  Bus Selector:RadarSensor:2_OBJ_S_Azimuth_BS/46 -> RadarSensor:2.OBJ_S_Azimuth_46/1  "<OBJ_S_Azimuth_46>"
  Bus Selector:RadarSensor:2_OBJ_S_Azimuth_BS/47 -> RadarSensor:2.OBJ_S_Azimuth_47/1  "<OBJ_S_Azimuth_47>"
  Bus Selector:RadarSensor:2_OBJ_S_Azimuth_BS/48 -> RadarSensor:2.OBJ_S_Azimuth_48/1  "<OBJ_S_Azimuth_48>"
  Bus Selector:RadarSensor:2_OBJ_S_Azimuth_BS/49 -> RadarSensor:2.OBJ_S_Azimuth_49/1  "<OBJ_S_Azimuth_49>"
  Bus Selector:RadarSensor:2_OBJ_S_Azimuth_BS/50 -> RadarSensor:2.OBJ_S_Azimuth_50/1  "<OBJ_S_Azimuth_50>"
  Bus Selector:RadarSensor:2_OBJ_S_Azimuth_BS/51 -> RadarSensor:2.OBJ_S_Azimuth_51/1  "<OBJ_S_Azimuth_51>"
  Bus Selector:RadarSensor:2_OBJ_S_Azimuth_BS/52 -> RadarSensor:2.OBJ_S_Azimuth_52/1  "<OBJ_S_Azimuth_52>"
  Bus Selector:RadarSensor:2_OBJ_S_Azimuth_BS/53 -> RadarSensor:2.OBJ_S_Azimuth_53/1  "<OBJ_S_Azimuth_53>"
  Bus Selector:RadarSensor:2_OBJ_S_Azimuth_BS/54 -> RadarSensor:2.OBJ_S_Azimuth_54/1  "<OBJ_S_Azimuth_54>"
  Bus Selector:RadarSensor:2_OBJ_S_Azimuth_BS/55 -> RadarSensor:2.OBJ_S_Azimuth_55/1  "<OBJ_S_Azimuth_55>"
  Bus Selector:RadarSensor:2_OBJ_S_Azimuth_BS/56 -> RadarSensor:2.OBJ_S_Azimuth_56/1  "<OBJ_S_Azimuth_56>"
  Bus Selector:RadarSensor:2_OBJ_S_Azimuth_BS/57 -> RadarSensor:2.OBJ_S_Azimuth_57/1  "<OBJ_S_Azimuth_57>"
  Bus Selector:RadarSensor:2_OBJ_S_Azimuth_BS/58 -> RadarSensor:2.OBJ_S_Azimuth_58/1  "<OBJ_S_Azimuth_58>"
  Bus Selector:RadarSensor:2_OBJ_S_Azimuth_BS/59 -> RadarSensor:2.OBJ_S_Azimuth_59/1  "<OBJ_S_Azimuth_59>"
  Bus Selector:RadarSensor:2_OBJ_S_Azimuth_BS/60 -> RadarSensor:2.OBJ_S_Azimuth_60/1  "<OBJ_S_Azimuth_60>"
  Bus Selector:RadarSensor:2_OBJ_S_Azimuth_BS/61 -> RadarSensor:2.OBJ_S_Azimuth_61/1  "<OBJ_S_Azimuth_61>"
  Bus Selector:RadarSensor:2_OBJ_S_Azimuth_BS/62 -> RadarSensor:2.OBJ_S_Azimuth_62/1  "<OBJ_S_Azimuth_62>"
  Bus Selector:RadarSensor:2_OBJ_S_Azimuth_BS/63 -> RadarSensor:2.OBJ_S_Azimuth_63/1  "<OBJ_S_Azimuth_63>"
  Bus Selector:RadarSensor:2_OBJ_S_Azimuth_BS/64 -> RadarSensor:2.OBJ_S_Azimuth_64/1  "<OBJ_S_Azimuth_64>"
  Bus Selector:RadarSensor:2_OBJ_S_Elevation_BS/1 -> RadarSensor:2.OBJ_S_Elevation_1/1  "<OBJ_S_Elevation_1>"
  Bus Selector:RadarSensor:2_OBJ_S_Elevation_BS/2 -> RadarSensor:2.OBJ_S_Elevation_2/1  "<OBJ_S_Elevation_2>"
  Bus Selector:RadarSensor:2_OBJ_S_Elevation_BS/3 -> RadarSensor:2.OBJ_S_Elevation_3/1  "<OBJ_S_Elevation_3>"
  Bus Selector:RadarSensor:2_OBJ_S_Elevation_BS/4 -> RadarSensor:2.OBJ_S_Elevation_4/1  "<OBJ_S_Elevation_4>"
  Bus Selector:RadarSensor:2_OBJ_S_Elevation_BS/5 -> RadarSensor:2.OBJ_S_Elevation_5/1  "<OBJ_S_Elevation_5>"
  Bus Selector:RadarSensor:2_OBJ_S_Elevation_BS/6 -> RadarSensor:2.OBJ_S_Elevation_6/1  "<OBJ_S_Elevation_6>"
  Bus Selector:RadarSensor:2_OBJ_S_Elevation_BS/7 -> RadarSensor:2.OBJ_S_Elevation_7/1  "<OBJ_S_Elevation_7>"
  Bus Selector:RadarSensor:2_OBJ_S_Elevation_BS/8 -> RadarSensor:2.OBJ_S_Elevation_8/1  "<OBJ_S_Elevation_8>"
  Bus Selector:RadarSensor:2_OBJ_S_Elevation_BS/9 -> RadarSensor:2.OBJ_S_Elevation_9/1  "<OBJ_S_Elevation_9>"
  Bus Selector:RadarSensor:2_OBJ_S_Elevation_BS/10 -> RadarSensor:2.OBJ_S_Elevation_10/1  "<OBJ_S_Elevation_10>"
  Bus Selector:RadarSensor:2_OBJ_S_Elevation_BS/11 -> RadarSensor:2.OBJ_S_Elevation_11/1  "<OBJ_S_Elevation_11>"
  Bus Selector:RadarSensor:2_OBJ_S_Elevation_BS/12 -> RadarSensor:2.OBJ_S_Elevation_12/1  "<OBJ_S_Elevation_12>"
  Bus Selector:RadarSensor:2_OBJ_S_Elevation_BS/13 -> RadarSensor:2.OBJ_S_Elevation_13/1  "<OBJ_S_Elevation_13>"
  Bus Selector:RadarSensor:2_OBJ_S_Elevation_BS/14 -> RadarSensor:2.OBJ_S_Elevation_14/1  "<OBJ_S_Elevation_14>"
  Bus Selector:RadarSensor:2_OBJ_S_Elevation_BS/15 -> RadarSensor:2.OBJ_S_Elevation_15/1  "<OBJ_S_Elevation_15>"
  Bus Selector:RadarSensor:2_OBJ_S_Elevation_BS/16 -> RadarSensor:2.OBJ_S_Elevation_16/1  "<OBJ_S_Elevation_16>"
  Bus Selector:RadarSensor:2_OBJ_S_Elevation_BS/17 -> RadarSensor:2.OBJ_S_Elevation_17/1  "<OBJ_S_Elevation_17>"
  Bus Selector:RadarSensor:2_OBJ_S_Elevation_BS/18 -> RadarSensor:2.OBJ_S_Elevation_18/1  "<OBJ_S_Elevation_18>"
  Bus Selector:RadarSensor:2_OBJ_S_Elevation_BS/19 -> RadarSensor:2.OBJ_S_Elevation_19/1  "<OBJ_S_Elevation_19>"
  Bus Selector:RadarSensor:2_OBJ_S_Elevation_BS/20 -> RadarSensor:2.OBJ_S_Elevation_20/1  "<OBJ_S_Elevation_20>"
  Bus Selector:RadarSensor:2_OBJ_S_Elevation_BS/21 -> RadarSensor:2.OBJ_S_Elevation_21/1  "<OBJ_S_Elevation_21>"
  Bus Selector:RadarSensor:2_OBJ_S_Elevation_BS/22 -> RadarSensor:2.OBJ_S_Elevation_22/1  "<OBJ_S_Elevation_22>"
  Bus Selector:RadarSensor:2_OBJ_S_Elevation_BS/23 -> RadarSensor:2.OBJ_S_Elevation_23/1  "<OBJ_S_Elevation_23>"
  Bus Selector:RadarSensor:2_OBJ_S_Elevation_BS/24 -> RadarSensor:2.OBJ_S_Elevation_24/1  "<OBJ_S_Elevation_24>"
  Bus Selector:RadarSensor:2_OBJ_S_Elevation_BS/25 -> RadarSensor:2.OBJ_S_Elevation_25/1  "<OBJ_S_Elevation_25>"
  Bus Selector:RadarSensor:2_OBJ_S_Elevation_BS/26 -> RadarSensor:2.OBJ_S_Elevation_26/1  "<OBJ_S_Elevation_26>"
  Bus Selector:RadarSensor:2_OBJ_S_Elevation_BS/27 -> RadarSensor:2.OBJ_S_Elevation_27/1  "<OBJ_S_Elevation_27>"
  Bus Selector:RadarSensor:2_OBJ_S_Elevation_BS/28 -> RadarSensor:2.OBJ_S_Elevation_28/1  "<OBJ_S_Elevation_28>"
  Bus Selector:RadarSensor:2_OBJ_S_Elevation_BS/29 -> RadarSensor:2.OBJ_S_Elevation_29/1  "<OBJ_S_Elevation_29>"
  Bus Selector:RadarSensor:2_OBJ_S_Elevation_BS/30 -> RadarSensor:2.OBJ_S_Elevation_30/1  "<OBJ_S_Elevation_30>"
  Bus Selector:RadarSensor:2_OBJ_S_Elevation_BS/31 -> RadarSensor:2.OBJ_S_Elevation_31/1  "<OBJ_S_Elevation_31>"
  Bus Selector:RadarSensor:2_OBJ_S_Elevation_BS/32 -> RadarSensor:2.OBJ_S_Elevation_32/1  "<OBJ_S_Elevation_32>"
  Bus Selector:RadarSensor:2_OBJ_S_Elevation_BS/33 -> RadarSensor:2.OBJ_S_Elevation_33/1  "<OBJ_S_Elevation_33>"
  Bus Selector:RadarSensor:2_OBJ_S_Elevation_BS/34 -> RadarSensor:2.OBJ_S_Elevation_34/1  "<OBJ_S_Elevation_34>"
  Bus Selector:RadarSensor:2_OBJ_S_Elevation_BS/35 -> RadarSensor:2.OBJ_S_Elevation_35/1  "<OBJ_S_Elevation_35>"
  Bus Selector:RadarSensor:2_OBJ_S_Elevation_BS/36 -> RadarSensor:2.OBJ_S_Elevation_36/1  "<OBJ_S_Elevation_36>"
  Bus Selector:RadarSensor:2_OBJ_S_Elevation_BS/37 -> RadarSensor:2.OBJ_S_Elevation_37/1  "<OBJ_S_Elevation_37>"
  Bus Selector:RadarSensor:2_OBJ_S_Elevation_BS/38 -> RadarSensor:2.OBJ_S_Elevation_38/1  "<OBJ_S_Elevation_38>"
  Bus Selector:RadarSensor:2_OBJ_S_Elevation_BS/39 -> RadarSensor:2.OBJ_S_Elevation_39/1  "<OBJ_S_Elevation_39>"
  Bus Selector:RadarSensor:2_OBJ_S_Elevation_BS/40 -> RadarSensor:2.OBJ_S_Elevation_40/1  "<OBJ_S_Elevation_40>"
  Bus Selector:RadarSensor:2_OBJ_S_Elevation_BS/41 -> RadarSensor:2.OBJ_S_Elevation_41/1  "<OBJ_S_Elevation_41>"
  Bus Selector:RadarSensor:2_OBJ_S_Elevation_BS/42 -> RadarSensor:2.OBJ_S_Elevation_42/1  "<OBJ_S_Elevation_42>"
  Bus Selector:RadarSensor:2_OBJ_S_Elevation_BS/43 -> RadarSensor:2.OBJ_S_Elevation_43/1  "<OBJ_S_Elevation_43>"
  Bus Selector:RadarSensor:2_OBJ_S_Elevation_BS/44 -> RadarSensor:2.OBJ_S_Elevation_44/1  "<OBJ_S_Elevation_44>"
  Bus Selector:RadarSensor:2_OBJ_S_Elevation_BS/45 -> RadarSensor:2.OBJ_S_Elevation_45/1  "<OBJ_S_Elevation_45>"
  Bus Selector:RadarSensor:2_OBJ_S_Elevation_BS/46 -> RadarSensor:2.OBJ_S_Elevation_46/1  "<OBJ_S_Elevation_46>"
  Bus Selector:RadarSensor:2_OBJ_S_Elevation_BS/47 -> RadarSensor:2.OBJ_S_Elevation_47/1  "<OBJ_S_Elevation_47>"
  Bus Selector:RadarSensor:2_OBJ_S_Elevation_BS/48 -> RadarSensor:2.OBJ_S_Elevation_48/1  "<OBJ_S_Elevation_48>"
  Bus Selector:RadarSensor:2_OBJ_S_Elevation_BS/49 -> RadarSensor:2.OBJ_S_Elevation_49/1  "<OBJ_S_Elevation_49>"
  Bus Selector:RadarSensor:2_OBJ_S_Elevation_BS/50 -> RadarSensor:2.OBJ_S_Elevation_50/1  "<OBJ_S_Elevation_50>"
  Bus Selector:RadarSensor:2_OBJ_S_Elevation_BS/51 -> RadarSensor:2.OBJ_S_Elevation_51/1  "<OBJ_S_Elevation_51>"
  Bus Selector:RadarSensor:2_OBJ_S_Elevation_BS/52 -> RadarSensor:2.OBJ_S_Elevation_52/1  "<OBJ_S_Elevation_52>"
  Bus Selector:RadarSensor:2_OBJ_S_Elevation_BS/53 -> RadarSensor:2.OBJ_S_Elevation_53/1  "<OBJ_S_Elevation_53>"
  Bus Selector:RadarSensor:2_OBJ_S_Elevation_BS/54 -> RadarSensor:2.OBJ_S_Elevation_54/1  "<OBJ_S_Elevation_54>"
  Bus Selector:RadarSensor:2_OBJ_S_Elevation_BS/55 -> RadarSensor:2.OBJ_S_Elevation_55/1  "<OBJ_S_Elevation_55>"
  Bus Selector:RadarSensor:2_OBJ_S_Elevation_BS/56 -> RadarSensor:2.OBJ_S_Elevation_56/1  "<OBJ_S_Elevation_56>"
  Bus Selector:RadarSensor:2_OBJ_S_Elevation_BS/57 -> RadarSensor:2.OBJ_S_Elevation_57/1  "<OBJ_S_Elevation_57>"
  Bus Selector:RadarSensor:2_OBJ_S_Elevation_BS/58 -> RadarSensor:2.OBJ_S_Elevation_58/1  "<OBJ_S_Elevation_58>"
  Bus Selector:RadarSensor:2_OBJ_S_Elevation_BS/59 -> RadarSensor:2.OBJ_S_Elevation_59/1  "<OBJ_S_Elevation_59>"
  Bus Selector:RadarSensor:2_OBJ_S_Elevation_BS/60 -> RadarSensor:2.OBJ_S_Elevation_60/1  "<OBJ_S_Elevation_60>"
  Bus Selector:RadarSensor:2_OBJ_S_Elevation_BS/61 -> RadarSensor:2.OBJ_S_Elevation_61/1  "<OBJ_S_Elevation_61>"
  Bus Selector:RadarSensor:2_OBJ_S_Elevation_BS/62 -> RadarSensor:2.OBJ_S_Elevation_62/1  "<OBJ_S_Elevation_62>"
  Bus Selector:RadarSensor:2_OBJ_S_Elevation_BS/63 -> RadarSensor:2.OBJ_S_Elevation_63/1  "<OBJ_S_Elevation_63>"
  Bus Selector:RadarSensor:2_OBJ_S_Elevation_BS/64 -> RadarSensor:2.OBJ_S_Elevation_64/1  "<OBJ_S_Elevation_64>"
  Bus Selector:RadarSensor:2_OBJ_S_Velocity_BS/1 -> RadarSensor:2.OBJ_S_Velocity_1/1  "<OBJ_S_Velocity_1>"
  Bus Selector:RadarSensor:2_OBJ_S_Velocity_BS/2 -> RadarSensor:2.OBJ_S_Velocity_2/1  "<OBJ_S_Velocity_2>"
  Bus Selector:RadarSensor:2_OBJ_S_Velocity_BS/3 -> RadarSensor:2.OBJ_S_Velocity_3/1  "<OBJ_S_Velocity_3>"
  Bus Selector:RadarSensor:2_OBJ_S_Velocity_BS/4 -> RadarSensor:2.OBJ_S_Velocity_4/1  "<OBJ_S_Velocity_4>"
  Bus Selector:RadarSensor:2_OBJ_S_Velocity_BS/5 -> RadarSensor:2.OBJ_S_Velocity_5/1  "<OBJ_S_Velocity_5>"
  Bus Selector:RadarSensor:2_OBJ_S_Velocity_BS/6 -> RadarSensor:2.OBJ_S_Velocity_6/1  "<OBJ_S_Velocity_6>"
  Bus Selector:RadarSensor:2_OBJ_S_Velocity_BS/7 -> RadarSensor:2.OBJ_S_Velocity_7/1  "<OBJ_S_Velocity_7>"
  Bus Selector:RadarSensor:2_OBJ_S_Velocity_BS/8 -> RadarSensor:2.OBJ_S_Velocity_8/1  "<OBJ_S_Velocity_8>"
  Bus Selector:RadarSensor:2_OBJ_S_Velocity_BS/9 -> RadarSensor:2.OBJ_S_Velocity_9/1  "<OBJ_S_Velocity_9>"
  Bus Selector:RadarSensor:2_OBJ_S_Velocity_BS/10 -> RadarSensor:2.OBJ_S_Velocity_10/1  "<OBJ_S_Velocity_10>"
  Bus Selector:RadarSensor:2_OBJ_S_Velocity_BS/11 -> RadarSensor:2.OBJ_S_Velocity_11/1  "<OBJ_S_Velocity_11>"
  Bus Selector:RadarSensor:2_OBJ_S_Velocity_BS/12 -> RadarSensor:2.OBJ_S_Velocity_12/1  "<OBJ_S_Velocity_12>"
  Bus Selector:RadarSensor:2_OBJ_S_Velocity_BS/13 -> RadarSensor:2.OBJ_S_Velocity_13/1  "<OBJ_S_Velocity_13>"
  Bus Selector:RadarSensor:2_OBJ_S_Velocity_BS/14 -> RadarSensor:2.OBJ_S_Velocity_14/1  "<OBJ_S_Velocity_14>"
  Bus Selector:RadarSensor:2_OBJ_S_Velocity_BS/15 -> RadarSensor:2.OBJ_S_Velocity_15/1  "<OBJ_S_Velocity_15>"
  Bus Selector:RadarSensor:2_OBJ_S_Velocity_BS/16 -> RadarSensor:2.OBJ_S_Velocity_16/1  "<OBJ_S_Velocity_16>"
  Bus Selector:RadarSensor:2_OBJ_S_Velocity_BS/17 -> RadarSensor:2.OBJ_S_Velocity_17/1  "<OBJ_S_Velocity_17>"
  Bus Selector:RadarSensor:2_OBJ_S_Velocity_BS/18 -> RadarSensor:2.OBJ_S_Velocity_18/1  "<OBJ_S_Velocity_18>"
  Bus Selector:RadarSensor:2_OBJ_S_Velocity_BS/19 -> RadarSensor:2.OBJ_S_Velocity_19/1  "<OBJ_S_Velocity_19>"
  Bus Selector:RadarSensor:2_OBJ_S_Velocity_BS/20 -> RadarSensor:2.OBJ_S_Velocity_20/1  "<OBJ_S_Velocity_20>"
  Bus Selector:RadarSensor:2_OBJ_S_Velocity_BS/21 -> RadarSensor:2.OBJ_S_Velocity_21/1  "<OBJ_S_Velocity_21>"
  Bus Selector:RadarSensor:2_OBJ_S_Velocity_BS/22 -> RadarSensor:2.OBJ_S_Velocity_22/1  "<OBJ_S_Velocity_22>"
  Bus Selector:RadarSensor:2_OBJ_S_Velocity_BS/23 -> RadarSensor:2.OBJ_S_Velocity_23/1  "<OBJ_S_Velocity_23>"
  Bus Selector:RadarSensor:2_OBJ_S_Velocity_BS/24 -> RadarSensor:2.OBJ_S_Velocity_24/1  "<OBJ_S_Velocity_24>"
  Bus Selector:RadarSensor:2_OBJ_S_Velocity_BS/25 -> RadarSensor:2.OBJ_S_Velocity_25/1  "<OBJ_S_Velocity_25>"
  Bus Selector:RadarSensor:2_OBJ_S_Velocity_BS/26 -> RadarSensor:2.OBJ_S_Velocity_26/1  "<OBJ_S_Velocity_26>"
  Bus Selector:RadarSensor:2_OBJ_S_Velocity_BS/27 -> RadarSensor:2.OBJ_S_Velocity_27/1  "<OBJ_S_Velocity_27>"
  Bus Selector:RadarSensor:2_OBJ_S_Velocity_BS/28 -> RadarSensor:2.OBJ_S_Velocity_28/1  "<OBJ_S_Velocity_28>"
  Bus Selector:RadarSensor:2_OBJ_S_Velocity_BS/29 -> RadarSensor:2.OBJ_S_Velocity_29/1  "<OBJ_S_Velocity_29>"
  Bus Selector:RadarSensor:2_OBJ_S_Velocity_BS/30 -> RadarSensor:2.OBJ_S_Velocity_30/1  "<OBJ_S_Velocity_30>"
  Bus Selector:RadarSensor:2_OBJ_S_Velocity_BS/31 -> RadarSensor:2.OBJ_S_Velocity_31/1  "<OBJ_S_Velocity_31>"
  Bus Selector:RadarSensor:2_OBJ_S_Velocity_BS/32 -> RadarSensor:2.OBJ_S_Velocity_32/1  "<OBJ_S_Velocity_32>"
  Bus Selector:RadarSensor:2_OBJ_S_Velocity_BS/33 -> RadarSensor:2.OBJ_S_Velocity_33/1  "<OBJ_S_Velocity_33>"
  Bus Selector:RadarSensor:2_OBJ_S_Velocity_BS/34 -> RadarSensor:2.OBJ_S_Velocity_34/1  "<OBJ_S_Velocity_34>"
  Bus Selector:RadarSensor:2_OBJ_S_Velocity_BS/35 -> RadarSensor:2.OBJ_S_Velocity_35/1  "<OBJ_S_Velocity_35>"
  Bus Selector:RadarSensor:2_OBJ_S_Velocity_BS/36 -> RadarSensor:2.OBJ_S_Velocity_36/1  "<OBJ_S_Velocity_36>"
  Bus Selector:RadarSensor:2_OBJ_S_Velocity_BS/37 -> RadarSensor:2.OBJ_S_Velocity_37/1  "<OBJ_S_Velocity_37>"
  Bus Selector:RadarSensor:2_OBJ_S_Velocity_BS/38 -> RadarSensor:2.OBJ_S_Velocity_38/1  "<OBJ_S_Velocity_38>"
  Bus Selector:RadarSensor:2_OBJ_S_Velocity_BS/39 -> RadarSensor:2.OBJ_S_Velocity_39/1  "<OBJ_S_Velocity_39>"
  Bus Selector:RadarSensor:2_OBJ_S_Velocity_BS/40 -> RadarSensor:2.OBJ_S_Velocity_40/1  "<OBJ_S_Velocity_40>"
  Bus Selector:RadarSensor:2_OBJ_S_Velocity_BS/41 -> RadarSensor:2.OBJ_S_Velocity_41/1  "<OBJ_S_Velocity_41>"
  Bus Selector:RadarSensor:2_OBJ_S_Velocity_BS/42 -> RadarSensor:2.OBJ_S_Velocity_42/1  "<OBJ_S_Velocity_42>"
  Bus Selector:RadarSensor:2_OBJ_S_Velocity_BS/43 -> RadarSensor:2.OBJ_S_Velocity_43/1  "<OBJ_S_Velocity_43>"
  Bus Selector:RadarSensor:2_OBJ_S_Velocity_BS/44 -> RadarSensor:2.OBJ_S_Velocity_44/1  "<OBJ_S_Velocity_44>"
  Bus Selector:RadarSensor:2_OBJ_S_Velocity_BS/45 -> RadarSensor:2.OBJ_S_Velocity_45/1  "<OBJ_S_Velocity_45>"
  Bus Selector:RadarSensor:2_OBJ_S_Velocity_BS/46 -> RadarSensor:2.OBJ_S_Velocity_46/1  "<OBJ_S_Velocity_46>"
  Bus Selector:RadarSensor:2_OBJ_S_Velocity_BS/47 -> RadarSensor:2.OBJ_S_Velocity_47/1  "<OBJ_S_Velocity_47>"
  Bus Selector:RadarSensor:2_OBJ_S_Velocity_BS/48 -> RadarSensor:2.OBJ_S_Velocity_48/1  "<OBJ_S_Velocity_48>"
  Bus Selector:RadarSensor:2_OBJ_S_Velocity_BS/49 -> RadarSensor:2.OBJ_S_Velocity_49/1  "<OBJ_S_Velocity_49>"
  Bus Selector:RadarSensor:2_OBJ_S_Velocity_BS/50 -> RadarSensor:2.OBJ_S_Velocity_50/1  "<OBJ_S_Velocity_50>"
  Bus Selector:RadarSensor:2_OBJ_S_Velocity_BS/51 -> RadarSensor:2.OBJ_S_Velocity_51/1  "<OBJ_S_Velocity_51>"
  Bus Selector:RadarSensor:2_OBJ_S_Velocity_BS/52 -> RadarSensor:2.OBJ_S_Velocity_52/1  "<OBJ_S_Velocity_52>"
  Bus Selector:RadarSensor:2_OBJ_S_Velocity_BS/53 -> RadarSensor:2.OBJ_S_Velocity_53/1  "<OBJ_S_Velocity_53>"
  Bus Selector:RadarSensor:2_OBJ_S_Velocity_BS/54 -> RadarSensor:2.OBJ_S_Velocity_54/1  "<OBJ_S_Velocity_54>"
  Bus Selector:RadarSensor:2_OBJ_S_Velocity_BS/55 -> RadarSensor:2.OBJ_S_Velocity_55/1  "<OBJ_S_Velocity_55>"
  Bus Selector:RadarSensor:2_OBJ_S_Velocity_BS/56 -> RadarSensor:2.OBJ_S_Velocity_56/1  "<OBJ_S_Velocity_56>"
  Bus Selector:RadarSensor:2_OBJ_S_Velocity_BS/57 -> RadarSensor:2.OBJ_S_Velocity_57/1  "<OBJ_S_Velocity_57>"
  Bus Selector:RadarSensor:2_OBJ_S_Velocity_BS/58 -> RadarSensor:2.OBJ_S_Velocity_58/1  "<OBJ_S_Velocity_58>"
  Bus Selector:RadarSensor:2_OBJ_S_Velocity_BS/59 -> RadarSensor:2.OBJ_S_Velocity_59/1  "<OBJ_S_Velocity_59>"
  Bus Selector:RadarSensor:2_OBJ_S_Velocity_BS/60 -> RadarSensor:2.OBJ_S_Velocity_60/1  "<OBJ_S_Velocity_60>"
  Bus Selector:RadarSensor:2_OBJ_S_Velocity_BS/61 -> RadarSensor:2.OBJ_S_Velocity_61/1  "<OBJ_S_Velocity_61>"
  Bus Selector:RadarSensor:2_OBJ_S_Velocity_BS/62 -> RadarSensor:2.OBJ_S_Velocity_62/1  "<OBJ_S_Velocity_62>"
  Bus Selector:RadarSensor:2_OBJ_S_Velocity_BS/63 -> RadarSensor:2.OBJ_S_Velocity_63/1  "<OBJ_S_Velocity_63>"
  Bus Selector:RadarSensor:2_OBJ_S_Velocity_BS/64 -> RadarSensor:2.OBJ_S_Velocity_64/1  "<OBJ_S_Velocity_64>"
  Bus Selector:RadarSensor:2_OBJ_S_Range_BS/1 -> RadarSensor:2.OBJ_S_Range_1/1  "<OBJ_S_Range_1>"
  Bus Selector:RadarSensor:2_OBJ_S_Range_BS/2 -> RadarSensor:2.OBJ_S_Range_2/1  "<OBJ_S_Range_2>"
  Bus Selector:RadarSensor:2_OBJ_S_Range_BS/3 -> RadarSensor:2.OBJ_S_Range_3/1  "<OBJ_S_Range_3>"
  Bus Selector:RadarSensor:2_OBJ_S_Range_BS/4 -> RadarSensor:2.OBJ_S_Range_4/1  "<OBJ_S_Range_4>"
  Bus Selector:RadarSensor:2_OBJ_S_Range_BS/5 -> RadarSensor:2.OBJ_S_Range_5/1  "<OBJ_S_Range_5>"
  Bus Selector:RadarSensor:2_OBJ_S_Range_BS/6 -> RadarSensor:2.OBJ_S_Range_6/1  "<OBJ_S_Range_6>"
  Bus Selector:RadarSensor:2_OBJ_S_Range_BS/7 -> RadarSensor:2.OBJ_S_Range_7/1  "<OBJ_S_Range_7>"
  Bus Selector:RadarSensor:2_OBJ_S_Range_BS/8 -> RadarSensor:2.OBJ_S_Range_8/1  "<OBJ_S_Range_8>"
  Bus Selector:RadarSensor:2_OBJ_S_Range_BS/9 -> RadarSensor:2.OBJ_S_Range_9/1  "<OBJ_S_Range_9>"
  Bus Selector:RadarSensor:2_OBJ_S_Range_BS/10 -> RadarSensor:2.OBJ_S_Range_10/1  "<OBJ_S_Range_10>"
  Bus Selector:RadarSensor:2_OBJ_S_Range_BS/11 -> RadarSensor:2.OBJ_S_Range_11/1  "<OBJ_S_Range_11>"
  Bus Selector:RadarSensor:2_OBJ_S_Range_BS/12 -> RadarSensor:2.OBJ_S_Range_12/1  "<OBJ_S_Range_12>"
  Bus Selector:RadarSensor:2_OBJ_S_Range_BS/13 -> RadarSensor:2.OBJ_S_Range_13/1  "<OBJ_S_Range_13>"
  Bus Selector:RadarSensor:2_OBJ_S_Range_BS/14 -> RadarSensor:2.OBJ_S_Range_14/1  "<OBJ_S_Range_14>"
  Bus Selector:RadarSensor:2_OBJ_S_Range_BS/15 -> RadarSensor:2.OBJ_S_Range_15/1  "<OBJ_S_Range_15>"
  Bus Selector:RadarSensor:2_OBJ_S_Range_BS/16 -> RadarSensor:2.OBJ_S_Range_16/1  "<OBJ_S_Range_16>"
  Bus Selector:RadarSensor:2_OBJ_S_Range_BS/17 -> RadarSensor:2.OBJ_S_Range_17/1  "<OBJ_S_Range_17>"
  Bus Selector:RadarSensor:2_OBJ_S_Range_BS/18 -> RadarSensor:2.OBJ_S_Range_18/1  "<OBJ_S_Range_18>"
  Bus Selector:RadarSensor:2_OBJ_S_Range_BS/19 -> RadarSensor:2.OBJ_S_Range_19/1  "<OBJ_S_Range_19>"
  Bus Selector:RadarSensor:2_OBJ_S_Range_BS/20 -> RadarSensor:2.OBJ_S_Range_20/1  "<OBJ_S_Range_20>"
  Bus Selector:RadarSensor:2_OBJ_S_Range_BS/21 -> RadarSensor:2.OBJ_S_Range_21/1  "<OBJ_S_Range_21>"
  Bus Selector:RadarSensor:2_OBJ_S_Range_BS/22 -> RadarSensor:2.OBJ_S_Range_22/1  "<OBJ_S_Range_22>"
  Bus Selector:RadarSensor:2_OBJ_S_Range_BS/23 -> RadarSensor:2.OBJ_S_Range_23/1  "<OBJ_S_Range_23>"
  Bus Selector:RadarSensor:2_OBJ_S_Range_BS/24 -> RadarSensor:2.OBJ_S_Range_24/1  "<OBJ_S_Range_24>"
  Bus Selector:RadarSensor:2_OBJ_S_Range_BS/25 -> RadarSensor:2.OBJ_S_Range_25/1  "<OBJ_S_Range_25>"
  Bus Selector:RadarSensor:2_OBJ_S_Range_BS/26 -> RadarSensor:2.OBJ_S_Range_26/1  "<OBJ_S_Range_26>"
  Bus Selector:RadarSensor:2_OBJ_S_Range_BS/27 -> RadarSensor:2.OBJ_S_Range_27/1  "<OBJ_S_Range_27>"
  Bus Selector:RadarSensor:2_OBJ_S_Range_BS/28 -> RadarSensor:2.OBJ_S_Range_28/1  "<OBJ_S_Range_28>"
  Bus Selector:RadarSensor:2_OBJ_S_Range_BS/29 -> RadarSensor:2.OBJ_S_Range_29/1  "<OBJ_S_Range_29>"
  Bus Selector:RadarSensor:2_OBJ_S_Range_BS/30 -> RadarSensor:2.OBJ_S_Range_30/1  "<OBJ_S_Range_30>"
  Bus Selector:RadarSensor:2_OBJ_S_Range_BS/31 -> RadarSensor:2.OBJ_S_Range_31/1  "<OBJ_S_Range_31>"
  Bus Selector:RadarSensor:2_OBJ_S_Range_BS/32 -> RadarSensor:2.OBJ_S_Range_32/1  "<OBJ_S_Range_32>"
  Bus Selector:RadarSensor:2_OBJ_S_Range_BS/33 -> RadarSensor:2.OBJ_S_Range_33/1  "<OBJ_S_Range_33>"
  Bus Selector:RadarSensor:2_OBJ_S_Range_BS/34 -> RadarSensor:2.OBJ_S_Range_34/1  "<OBJ_S_Range_34>"
  Bus Selector:RadarSensor:2_OBJ_S_Range_BS/35 -> RadarSensor:2.OBJ_S_Range_35/1  "<OBJ_S_Range_35>"
  Bus Selector:RadarSensor:2_OBJ_S_Range_BS/36 -> RadarSensor:2.OBJ_S_Range_36/1  "<OBJ_S_Range_36>"
  Bus Selector:RadarSensor:2_OBJ_S_Range_BS/37 -> RadarSensor:2.OBJ_S_Range_37/1  "<OBJ_S_Range_37>"
  Bus Selector:RadarSensor:2_OBJ_S_Range_BS/38 -> RadarSensor:2.OBJ_S_Range_38/1  "<OBJ_S_Range_38>"
  Bus Selector:RadarSensor:2_OBJ_S_Range_BS/39 -> RadarSensor:2.OBJ_S_Range_39/1  "<OBJ_S_Range_39>"
  Bus Selector:RadarSensor:2_OBJ_S_Range_BS/40 -> RadarSensor:2.OBJ_S_Range_40/1  "<OBJ_S_Range_40>"
  Bus Selector:RadarSensor:2_OBJ_S_Range_BS/41 -> RadarSensor:2.OBJ_S_Range_41/1  "<OBJ_S_Range_41>"
  Bus Selector:RadarSensor:2_OBJ_S_Range_BS/42 -> RadarSensor:2.OBJ_S_Range_42/1  "<OBJ_S_Range_42>"
  Bus Selector:RadarSensor:2_OBJ_S_Range_BS/43 -> RadarSensor:2.OBJ_S_Range_43/1  "<OBJ_S_Range_43>"
  Bus Selector:RadarSensor:2_OBJ_S_Range_BS/44 -> RadarSensor:2.OBJ_S_Range_44/1  "<OBJ_S_Range_44>"
  Bus Selector:RadarSensor:2_OBJ_S_Range_BS/45 -> RadarSensor:2.OBJ_S_Range_45/1  "<OBJ_S_Range_45>"
  Bus Selector:RadarSensor:2_OBJ_S_Range_BS/46 -> RadarSensor:2.OBJ_S_Range_46/1  "<OBJ_S_Range_46>"
  Bus Selector:RadarSensor:2_OBJ_S_Range_BS/47 -> RadarSensor:2.OBJ_S_Range_47/1  "<OBJ_S_Range_47>"
  Bus Selector:RadarSensor:2_OBJ_S_Range_BS/48 -> RadarSensor:2.OBJ_S_Range_48/1  "<OBJ_S_Range_48>"
  Bus Selector:RadarSensor:2_OBJ_S_Range_BS/49 -> RadarSensor:2.OBJ_S_Range_49/1  "<OBJ_S_Range_49>"
  Bus Selector:RadarSensor:2_OBJ_S_Range_BS/50 -> RadarSensor:2.OBJ_S_Range_50/1  "<OBJ_S_Range_50>"
  Bus Selector:RadarSensor:2_OBJ_S_Range_BS/51 -> RadarSensor:2.OBJ_S_Range_51/1  "<OBJ_S_Range_51>"
  Bus Selector:RadarSensor:2_OBJ_S_Range_BS/52 -> RadarSensor:2.OBJ_S_Range_52/1  "<OBJ_S_Range_52>"
  Bus Selector:RadarSensor:2_OBJ_S_Range_BS/53 -> RadarSensor:2.OBJ_S_Range_53/1  "<OBJ_S_Range_53>"
  Bus Selector:RadarSensor:2_OBJ_S_Range_BS/54 -> RadarSensor:2.OBJ_S_Range_54/1  "<OBJ_S_Range_54>"
  Bus Selector:RadarSensor:2_OBJ_S_Range_BS/55 -> RadarSensor:2.OBJ_S_Range_55/1  "<OBJ_S_Range_55>"
  Bus Selector:RadarSensor:2_OBJ_S_Range_BS/56 -> RadarSensor:2.OBJ_S_Range_56/1  "<OBJ_S_Range_56>"
  Bus Selector:RadarSensor:2_OBJ_S_Range_BS/57 -> RadarSensor:2.OBJ_S_Range_57/1  "<OBJ_S_Range_57>"
  Bus Selector:RadarSensor:2_OBJ_S_Range_BS/58 -> RadarSensor:2.OBJ_S_Range_58/1  "<OBJ_S_Range_58>"
  Bus Selector:RadarSensor:2_OBJ_S_Range_BS/59 -> RadarSensor:2.OBJ_S_Range_59/1  "<OBJ_S_Range_59>"
  Bus Selector:RadarSensor:2_OBJ_S_Range_BS/60 -> RadarSensor:2.OBJ_S_Range_60/1  "<OBJ_S_Range_60>"
  Bus Selector:RadarSensor:2_OBJ_S_Range_BS/61 -> RadarSensor:2.OBJ_S_Range_61/1  "<OBJ_S_Range_61>"
  Bus Selector:RadarSensor:2_OBJ_S_Range_BS/62 -> RadarSensor:2.OBJ_S_Range_62/1  "<OBJ_S_Range_62>"
  Bus Selector:RadarSensor:2_OBJ_S_Range_BS/63 -> RadarSensor:2.OBJ_S_Range_63/1  "<OBJ_S_Range_63>"
  Bus Selector:RadarSensor:2_OBJ_S_Range_BS/64 -> RadarSensor:2.OBJ_S_Range_64/1  "<OBJ_S_Range_64>"
  Bus Selector:RadarSensor:2_OBJ_RCS_BS/1 -> RadarSensor:2.OBJ_RCS_1/1  "<OBJ_RCS_1>"
  Bus Selector:RadarSensor:2_OBJ_RCS_BS/2 -> RadarSensor:2.OBJ_RCS_2/1  "<OBJ_RCS_2>"
  Bus Selector:RadarSensor:2_OBJ_RCS_BS/3 -> RadarSensor:2.OBJ_RCS_3/1  "<OBJ_RCS_3>"
  Bus Selector:RadarSensor:2_OBJ_RCS_BS/4 -> RadarSensor:2.OBJ_RCS_4/1  "<OBJ_RCS_4>"
  Bus Selector:RadarSensor:2_OBJ_RCS_BS/5 -> RadarSensor:2.OBJ_RCS_5/1  "<OBJ_RCS_5>"
  Bus Selector:RadarSensor:2_OBJ_RCS_BS/6 -> RadarSensor:2.OBJ_RCS_6/1  "<OBJ_RCS_6>"
  Bus Selector:RadarSensor:2_OBJ_RCS_BS/7 -> RadarSensor:2.OBJ_RCS_7/1  "<OBJ_RCS_7>"
  Bus Selector:RadarSensor:2_OBJ_RCS_BS/8 -> RadarSensor:2.OBJ_RCS_8/1  "<OBJ_RCS_8>"
  Bus Selector:RadarSensor:2_OBJ_RCS_BS/9 -> RadarSensor:2.OBJ_RCS_9/1  "<OBJ_RCS_9>"
  Bus Selector:RadarSensor:2_OBJ_RCS_BS/10 -> RadarSensor:2.OBJ_RCS_10/1  "<OBJ_RCS_10>"
  Bus Selector:RadarSensor:2_OBJ_RCS_BS/11 -> RadarSensor:2.OBJ_RCS_11/1  "<OBJ_RCS_11>"
  Bus Selector:RadarSensor:2_OBJ_RCS_BS/12 -> RadarSensor:2.OBJ_RCS_12/1  "<OBJ_RCS_12>"
  Bus Selector:RadarSensor:2_OBJ_RCS_BS/13 -> RadarSensor:2.OBJ_RCS_13/1  "<OBJ_RCS_13>"
  Bus Selector:RadarSensor:2_OBJ_RCS_BS/14 -> RadarSensor:2.OBJ_RCS_14/1  "<OBJ_RCS_14>"
  Bus Selector:RadarSensor:2_OBJ_RCS_BS/15 -> RadarSensor:2.OBJ_RCS_15/1  "<OBJ_RCS_15>"
  Bus Selector:RadarSensor:2_OBJ_RCS_BS/16 -> RadarSensor:2.OBJ_RCS_16/1  "<OBJ_RCS_16>"
  Bus Selector:RadarSensor:2_OBJ_RCS_BS/17 -> RadarSensor:2.OBJ_RCS_17/1  "<OBJ_RCS_17>"
  Bus Selector:RadarSensor:2_OBJ_RCS_BS/18 -> RadarSensor:2.OBJ_RCS_18/1  "<OBJ_RCS_18>"
  Bus Selector:RadarSensor:2_OBJ_RCS_BS/19 -> RadarSensor:2.OBJ_RCS_19/1  "<OBJ_RCS_19>"
  Bus Selector:RadarSensor:2_OBJ_RCS_BS/20 -> RadarSensor:2.OBJ_RCS_20/1  "<OBJ_RCS_20>"
  Bus Selector:RadarSensor:2_OBJ_RCS_BS/21 -> RadarSensor:2.OBJ_RCS_21/1  "<OBJ_RCS_21>"
  Bus Selector:RadarSensor:2_OBJ_RCS_BS/22 -> RadarSensor:2.OBJ_RCS_22/1  "<OBJ_RCS_22>"
  Bus Selector:RadarSensor:2_OBJ_RCS_BS/23 -> RadarSensor:2.OBJ_RCS_23/1  "<OBJ_RCS_23>"
  Bus Selector:RadarSensor:2_OBJ_RCS_BS/24 -> RadarSensor:2.OBJ_RCS_24/1  "<OBJ_RCS_24>"
  Bus Selector:RadarSensor:2_OBJ_RCS_BS/25 -> RadarSensor:2.OBJ_RCS_25/1  "<OBJ_RCS_25>"
  Bus Selector:RadarSensor:2_OBJ_RCS_BS/26 -> RadarSensor:2.OBJ_RCS_26/1  "<OBJ_RCS_26>"
  Bus Selector:RadarSensor:2_OBJ_RCS_BS/27 -> RadarSensor:2.OBJ_RCS_27/1  "<OBJ_RCS_27>"
  Bus Selector:RadarSensor:2_OBJ_RCS_BS/28 -> RadarSensor:2.OBJ_RCS_28/1  "<OBJ_RCS_28>"
  Bus Selector:RadarSensor:2_OBJ_RCS_BS/29 -> RadarSensor:2.OBJ_RCS_29/1  "<OBJ_RCS_29>"
  Bus Selector:RadarSensor:2_OBJ_RCS_BS/30 -> RadarSensor:2.OBJ_RCS_30/1  "<OBJ_RCS_30>"
  Bus Selector:RadarSensor:2_OBJ_RCS_BS/31 -> RadarSensor:2.OBJ_RCS_31/1  "<OBJ_RCS_31>"
  Bus Selector:RadarSensor:2_OBJ_RCS_BS/32 -> RadarSensor:2.OBJ_RCS_32/1  "<OBJ_RCS_32>"
  Bus Selector:RadarSensor:2_OBJ_RCS_BS/33 -> RadarSensor:2.OBJ_RCS_33/1  "<OBJ_RCS_33>"
  Bus Selector:RadarSensor:2_OBJ_RCS_BS/34 -> RadarSensor:2.OBJ_RCS_34/1  "<OBJ_RCS_34>"
  Bus Selector:RadarSensor:2_OBJ_RCS_BS/35 -> RadarSensor:2.OBJ_RCS_35/1  "<OBJ_RCS_35>"
  Bus Selector:RadarSensor:2_OBJ_RCS_BS/36 -> RadarSensor:2.OBJ_RCS_36/1  "<OBJ_RCS_36>"
  Bus Selector:RadarSensor:2_OBJ_RCS_BS/37 -> RadarSensor:2.OBJ_RCS_37/1  "<OBJ_RCS_37>"
  Bus Selector:RadarSensor:2_OBJ_RCS_BS/38 -> RadarSensor:2.OBJ_RCS_38/1  "<OBJ_RCS_38>"
  Bus Selector:RadarSensor:2_OBJ_RCS_BS/39 -> RadarSensor:2.OBJ_RCS_39/1  "<OBJ_RCS_39>"
  Bus Selector:RadarSensor:2_OBJ_RCS_BS/40 -> RadarSensor:2.OBJ_RCS_40/1  "<OBJ_RCS_40>"
  Bus Selector:RadarSensor:2_OBJ_RCS_BS/41 -> RadarSensor:2.OBJ_RCS_41/1  "<OBJ_RCS_41>"
  Bus Selector:RadarSensor:2_OBJ_RCS_BS/42 -> RadarSensor:2.OBJ_RCS_42/1  "<OBJ_RCS_42>"
  Bus Selector:RadarSensor:2_OBJ_RCS_BS/43 -> RadarSensor:2.OBJ_RCS_43/1  "<OBJ_RCS_43>"
  Bus Selector:RadarSensor:2_OBJ_RCS_BS/44 -> RadarSensor:2.OBJ_RCS_44/1  "<OBJ_RCS_44>"
  Bus Selector:RadarSensor:2_OBJ_RCS_BS/45 -> RadarSensor:2.OBJ_RCS_45/1  "<OBJ_RCS_45>"
  Bus Selector:RadarSensor:2_OBJ_RCS_BS/46 -> RadarSensor:2.OBJ_RCS_46/1  "<OBJ_RCS_46>"
  Bus Selector:RadarSensor:2_OBJ_RCS_BS/47 -> RadarSensor:2.OBJ_RCS_47/1  "<OBJ_RCS_47>"
  Bus Selector:RadarSensor:2_OBJ_RCS_BS/48 -> RadarSensor:2.OBJ_RCS_48/1  "<OBJ_RCS_48>"
  Bus Selector:RadarSensor:2_OBJ_RCS_BS/49 -> RadarSensor:2.OBJ_RCS_49/1  "<OBJ_RCS_49>"
  Bus Selector:RadarSensor:2_OBJ_RCS_BS/50 -> RadarSensor:2.OBJ_RCS_50/1  "<OBJ_RCS_50>"
  Bus Selector:RadarSensor:2_OBJ_RCS_BS/51 -> RadarSensor:2.OBJ_RCS_51/1  "<OBJ_RCS_51>"
  Bus Selector:RadarSensor:2_OBJ_RCS_BS/52 -> RadarSensor:2.OBJ_RCS_52/1  "<OBJ_RCS_52>"
  Bus Selector:RadarSensor:2_OBJ_RCS_BS/53 -> RadarSensor:2.OBJ_RCS_53/1  "<OBJ_RCS_53>"
  Bus Selector:RadarSensor:2_OBJ_RCS_BS/54 -> RadarSensor:2.OBJ_RCS_54/1  "<OBJ_RCS_54>"
  Bus Selector:RadarSensor:2_OBJ_RCS_BS/55 -> RadarSensor:2.OBJ_RCS_55/1  "<OBJ_RCS_55>"
  Bus Selector:RadarSensor:2_OBJ_RCS_BS/56 -> RadarSensor:2.OBJ_RCS_56/1  "<OBJ_RCS_56>"
  Bus Selector:RadarSensor:2_OBJ_RCS_BS/57 -> RadarSensor:2.OBJ_RCS_57/1  "<OBJ_RCS_57>"
  Bus Selector:RadarSensor:2_OBJ_RCS_BS/58 -> RadarSensor:2.OBJ_RCS_58/1  "<OBJ_RCS_58>"
  Bus Selector:RadarSensor:2_OBJ_RCS_BS/59 -> RadarSensor:2.OBJ_RCS_59/1  "<OBJ_RCS_59>"
  Bus Selector:RadarSensor:2_OBJ_RCS_BS/60 -> RadarSensor:2.OBJ_RCS_60/1  "<OBJ_RCS_60>"
  Bus Selector:RadarSensor:2_OBJ_RCS_BS/61 -> RadarSensor:2.OBJ_RCS_61/1  "<OBJ_RCS_61>"
  Bus Selector:RadarSensor:2_OBJ_RCS_BS/62 -> RadarSensor:2.OBJ_RCS_62/1  "<OBJ_RCS_62>"
  Bus Selector:RadarSensor:2_OBJ_RCS_BS/63 -> RadarSensor:2.OBJ_RCS_63/1  "<OBJ_RCS_63>"
  Bus Selector:RadarSensor:2_OBJ_RCS_BS/64 -> RadarSensor:2.OBJ_RCS_64/1  "<OBJ_RCS_64>"
  Bus Selector:RadarSensor:2/1 -> RadarSensor:2.time/1  "<time>"
  Bus Selector:RadarSensor:2/2 -> RadarSensor:2.width/1  "<width>"
  Bus Selector:RadarSensor:2/3 -> RadarSensor:2.OBJ_ID/1, Bus Selector:RadarSensor:2_OBJ_ID_BS/1  "<OBJ_ID>"
  Bus Selector:RadarSensor:2/4 -> RadarSensor:2.OBJ_Class/1, Bus Selector:RadarSensor:2_OBJ_Class_BS/1  "<OBJ_Class>"
  Bus Selector:RadarSensor:2/5 -> RadarSensor:2.OBJ_S_Azimuth/1, Bus Selector:RadarSensor:2_OBJ_S_Azimuth_BS/1  "<OBJ_S_Azimuth>"
  Bus Selector:RadarSensor:2/6 -> RadarSensor:2.OBJ_S_Elevation/1, Bus Selector:RadarSensor:2_OBJ_S_Elevation_BS/1  "<OBJ_S_Elevation>"
  Bus Selector:RadarSensor:2/7 -> RadarSensor:2.OBJ_S_Velocity/1, Bus Selector:RadarSensor:2_OBJ_S_Velocity_BS/1  "<OBJ_S_Velocity>"
  Bus Selector:RadarSensor:2/8 -> RadarSensor:2.OBJ_S_Range/1, Bus Selector:RadarSensor:2_OBJ_S_Range_BS/1  "<OBJ_S_Range>"
  Bus Selector:RadarSensor:2/9 -> RadarSensor:2.OBJ_RCS/1, Bus Selector:RadarSensor:2_OBJ_RCS_BS/1  "<OBJ_RCS>"
  Bus Selector:RadarSensor:3_OBJ_ID_BS/1 -> RadarSensor:3.OBJ_ID_1/1  "<OBJ_ID_1>"
  Bus Selector:RadarSensor:3_OBJ_ID_BS/2 -> RadarSensor:3.OBJ_ID_2/1  "<OBJ_ID_2>"
  Bus Selector:RadarSensor:3_OBJ_ID_BS/3 -> RadarSensor:3.OBJ_ID_3/1  "<OBJ_ID_3>"
  Bus Selector:RadarSensor:3_OBJ_ID_BS/4 -> RadarSensor:3.OBJ_ID_4/1  "<OBJ_ID_4>"
  Bus Selector:RadarSensor:3_OBJ_ID_BS/5 -> RadarSensor:3.OBJ_ID_5/1  "<OBJ_ID_5>"
  Bus Selector:RadarSensor:3_OBJ_ID_BS/6 -> RadarSensor:3.OBJ_ID_6/1  "<OBJ_ID_6>"
  Bus Selector:RadarSensor:3_OBJ_ID_BS/7 -> RadarSensor:3.OBJ_ID_7/1  "<OBJ_ID_7>"
  Bus Selector:RadarSensor:3_OBJ_ID_BS/8 -> RadarSensor:3.OBJ_ID_8/1  "<OBJ_ID_8>"
  Bus Selector:RadarSensor:3_OBJ_ID_BS/9 -> RadarSensor:3.OBJ_ID_9/1  "<OBJ_ID_9>"
  Bus Selector:RadarSensor:3_OBJ_ID_BS/10 -> RadarSensor:3.OBJ_ID_10/1  "<OBJ_ID_10>"
  Bus Selector:RadarSensor:3_OBJ_ID_BS/11 -> RadarSensor:3.OBJ_ID_11/1  "<OBJ_ID_11>"
  Bus Selector:RadarSensor:3_OBJ_ID_BS/12 -> RadarSensor:3.OBJ_ID_12/1  "<OBJ_ID_12>"
  Bus Selector:RadarSensor:3_OBJ_ID_BS/13 -> RadarSensor:3.OBJ_ID_13/1  "<OBJ_ID_13>"
  Bus Selector:RadarSensor:3_OBJ_ID_BS/14 -> RadarSensor:3.OBJ_ID_14/1  "<OBJ_ID_14>"
  Bus Selector:RadarSensor:3_OBJ_ID_BS/15 -> RadarSensor:3.OBJ_ID_15/1  "<OBJ_ID_15>"
  Bus Selector:RadarSensor:3_OBJ_ID_BS/16 -> RadarSensor:3.OBJ_ID_16/1  "<OBJ_ID_16>"
  Bus Selector:RadarSensor:3_OBJ_ID_BS/17 -> RadarSensor:3.OBJ_ID_17/1  "<OBJ_ID_17>"
  Bus Selector:RadarSensor:3_OBJ_ID_BS/18 -> RadarSensor:3.OBJ_ID_18/1  "<OBJ_ID_18>"
  Bus Selector:RadarSensor:3_OBJ_ID_BS/19 -> RadarSensor:3.OBJ_ID_19/1  "<OBJ_ID_19>"
  Bus Selector:RadarSensor:3_OBJ_ID_BS/20 -> RadarSensor:3.OBJ_ID_20/1  "<OBJ_ID_20>"
  Bus Selector:RadarSensor:3_OBJ_ID_BS/21 -> RadarSensor:3.OBJ_ID_21/1  "<OBJ_ID_21>"
  Bus Selector:RadarSensor:3_OBJ_ID_BS/22 -> RadarSensor:3.OBJ_ID_22/1  "<OBJ_ID_22>"
  Bus Selector:RadarSensor:3_OBJ_ID_BS/23 -> RadarSensor:3.OBJ_ID_23/1  "<OBJ_ID_23>"
  Bus Selector:RadarSensor:3_OBJ_ID_BS/24 -> RadarSensor:3.OBJ_ID_24/1  "<OBJ_ID_24>"
  Bus Selector:RadarSensor:3_OBJ_ID_BS/25 -> RadarSensor:3.OBJ_ID_25/1  "<OBJ_ID_25>"
  Bus Selector:RadarSensor:3_OBJ_ID_BS/26 -> RadarSensor:3.OBJ_ID_26/1  "<OBJ_ID_26>"
  Bus Selector:RadarSensor:3_OBJ_ID_BS/27 -> RadarSensor:3.OBJ_ID_27/1  "<OBJ_ID_27>"
  Bus Selector:RadarSensor:3_OBJ_ID_BS/28 -> RadarSensor:3.OBJ_ID_28/1  "<OBJ_ID_28>"
  Bus Selector:RadarSensor:3_OBJ_ID_BS/29 -> RadarSensor:3.OBJ_ID_29/1  "<OBJ_ID_29>"
  Bus Selector:RadarSensor:3_OBJ_ID_BS/30 -> RadarSensor:3.OBJ_ID_30/1  "<OBJ_ID_30>"
  Bus Selector:RadarSensor:3_OBJ_ID_BS/31 -> RadarSensor:3.OBJ_ID_31/1  "<OBJ_ID_31>"
  Bus Selector:RadarSensor:3_OBJ_ID_BS/32 -> RadarSensor:3.OBJ_ID_32/1  "<OBJ_ID_32>"
  Bus Selector:RadarSensor:3_OBJ_ID_BS/33 -> RadarSensor:3.OBJ_ID_33/1  "<OBJ_ID_33>"
  Bus Selector:RadarSensor:3_OBJ_ID_BS/34 -> RadarSensor:3.OBJ_ID_34/1  "<OBJ_ID_34>"
  Bus Selector:RadarSensor:3_OBJ_ID_BS/35 -> RadarSensor:3.OBJ_ID_35/1  "<OBJ_ID_35>"
  Bus Selector:RadarSensor:3_OBJ_ID_BS/36 -> RadarSensor:3.OBJ_ID_36/1  "<OBJ_ID_36>"
  Bus Selector:RadarSensor:3_OBJ_ID_BS/37 -> RadarSensor:3.OBJ_ID_37/1  "<OBJ_ID_37>"
  Bus Selector:RadarSensor:3_OBJ_ID_BS/38 -> RadarSensor:3.OBJ_ID_38/1  "<OBJ_ID_38>"
  Bus Selector:RadarSensor:3_OBJ_ID_BS/39 -> RadarSensor:3.OBJ_ID_39/1  "<OBJ_ID_39>"
  Bus Selector:RadarSensor:3_OBJ_ID_BS/40 -> RadarSensor:3.OBJ_ID_40/1  "<OBJ_ID_40>"
  Bus Selector:RadarSensor:3_OBJ_ID_BS/41 -> RadarSensor:3.OBJ_ID_41/1  "<OBJ_ID_41>"
  Bus Selector:RadarSensor:3_OBJ_ID_BS/42 -> RadarSensor:3.OBJ_ID_42/1  "<OBJ_ID_42>"
  Bus Selector:RadarSensor:3_OBJ_ID_BS/43 -> RadarSensor:3.OBJ_ID_43/1  "<OBJ_ID_43>"
  Bus Selector:RadarSensor:3_OBJ_ID_BS/44 -> RadarSensor:3.OBJ_ID_44/1  "<OBJ_ID_44>"
  Bus Selector:RadarSensor:3_OBJ_ID_BS/45 -> RadarSensor:3.OBJ_ID_45/1  "<OBJ_ID_45>"
  Bus Selector:RadarSensor:3_OBJ_ID_BS/46 -> RadarSensor:3.OBJ_ID_46/1  "<OBJ_ID_46>"
  Bus Selector:RadarSensor:3_OBJ_ID_BS/47 -> RadarSensor:3.OBJ_ID_47/1  "<OBJ_ID_47>"
  Bus Selector:RadarSensor:3_OBJ_ID_BS/48 -> RadarSensor:3.OBJ_ID_48/1  "<OBJ_ID_48>"
  Bus Selector:RadarSensor:3_OBJ_ID_BS/49 -> RadarSensor:3.OBJ_ID_49/1  "<OBJ_ID_49>"
  Bus Selector:RadarSensor:3_OBJ_ID_BS/50 -> RadarSensor:3.OBJ_ID_50/1  "<OBJ_ID_50>"
  Bus Selector:RadarSensor:3_OBJ_ID_BS/51 -> RadarSensor:3.OBJ_ID_51/1  "<OBJ_ID_51>"
  Bus Selector:RadarSensor:3_OBJ_ID_BS/52 -> RadarSensor:3.OBJ_ID_52/1  "<OBJ_ID_52>"
  Bus Selector:RadarSensor:3_OBJ_ID_BS/53 -> RadarSensor:3.OBJ_ID_53/1  "<OBJ_ID_53>"
  Bus Selector:RadarSensor:3_OBJ_ID_BS/54 -> RadarSensor:3.OBJ_ID_54/1  "<OBJ_ID_54>"
  Bus Selector:RadarSensor:3_OBJ_ID_BS/55 -> RadarSensor:3.OBJ_ID_55/1  "<OBJ_ID_55>"
  Bus Selector:RadarSensor:3_OBJ_ID_BS/56 -> RadarSensor:3.OBJ_ID_56/1  "<OBJ_ID_56>"
  Bus Selector:RadarSensor:3_OBJ_ID_BS/57 -> RadarSensor:3.OBJ_ID_57/1  "<OBJ_ID_57>"
  Bus Selector:RadarSensor:3_OBJ_ID_BS/58 -> RadarSensor:3.OBJ_ID_58/1  "<OBJ_ID_58>"
  Bus Selector:RadarSensor:3_OBJ_ID_BS/59 -> RadarSensor:3.OBJ_ID_59/1  "<OBJ_ID_59>"
  Bus Selector:RadarSensor:3_OBJ_ID_BS/60 -> RadarSensor:3.OBJ_ID_60/1  "<OBJ_ID_60>"
  Bus Selector:RadarSensor:3_OBJ_ID_BS/61 -> RadarSensor:3.OBJ_ID_61/1  "<OBJ_ID_61>"
  Bus Selector:RadarSensor:3_OBJ_ID_BS/62 -> RadarSensor:3.OBJ_ID_62/1  "<OBJ_ID_62>"
  Bus Selector:RadarSensor:3_OBJ_ID_BS/63 -> RadarSensor:3.OBJ_ID_63/1  "<OBJ_ID_63>"
  Bus Selector:RadarSensor:3_OBJ_ID_BS/64 -> RadarSensor:3.OBJ_ID_64/1  "<OBJ_ID_64>"
  Bus Selector:RadarSensor:3_OBJ_Class_BS/1 -> RadarSensor:3.OBJ_Class_1/1  "<OBJ_Class_1>"
  Bus Selector:RadarSensor:3_OBJ_Class_BS/2 -> RadarSensor:3.OBJ_Class_2/1  "<OBJ_Class_2>"
  Bus Selector:RadarSensor:3_OBJ_Class_BS/3 -> RadarSensor:3.OBJ_Class_3/1  "<OBJ_Class_3>"
  Bus Selector:RadarSensor:3_OBJ_Class_BS/4 -> RadarSensor:3.OBJ_Class_4/1  "<OBJ_Class_4>"
  Bus Selector:RadarSensor:3_OBJ_Class_BS/5 -> RadarSensor:3.OBJ_Class_5/1  "<OBJ_Class_5>"
  Bus Selector:RadarSensor:3_OBJ_Class_BS/6 -> RadarSensor:3.OBJ_Class_6/1  "<OBJ_Class_6>"
  Bus Selector:RadarSensor:3_OBJ_Class_BS/7 -> RadarSensor:3.OBJ_Class_7/1  "<OBJ_Class_7>"
  Bus Selector:RadarSensor:3_OBJ_Class_BS/8 -> RadarSensor:3.OBJ_Class_8/1  "<OBJ_Class_8>"
  Bus Selector:RadarSensor:3_OBJ_Class_BS/9 -> RadarSensor:3.OBJ_Class_9/1  "<OBJ_Class_9>"
  Bus Selector:RadarSensor:3_OBJ_Class_BS/10 -> RadarSensor:3.OBJ_Class_10/1  "<OBJ_Class_10>"
  Bus Selector:RadarSensor:3_OBJ_Class_BS/11 -> RadarSensor:3.OBJ_Class_11/1  "<OBJ_Class_11>"
  Bus Selector:RadarSensor:3_OBJ_Class_BS/12 -> RadarSensor:3.OBJ_Class_12/1  "<OBJ_Class_12>"
  Bus Selector:RadarSensor:3_OBJ_Class_BS/13 -> RadarSensor:3.OBJ_Class_13/1  "<OBJ_Class_13>"
  Bus Selector:RadarSensor:3_OBJ_Class_BS/14 -> RadarSensor:3.OBJ_Class_14/1  "<OBJ_Class_14>"
  Bus Selector:RadarSensor:3_OBJ_Class_BS/15 -> RadarSensor:3.OBJ_Class_15/1  "<OBJ_Class_15>"
  Bus Selector:RadarSensor:3_OBJ_Class_BS/16 -> RadarSensor:3.OBJ_Class_16/1  "<OBJ_Class_16>"
  Bus Selector:RadarSensor:3_OBJ_Class_BS/17 -> RadarSensor:3.OBJ_Class_17/1  "<OBJ_Class_17>"
  Bus Selector:RadarSensor:3_OBJ_Class_BS/18 -> RadarSensor:3.OBJ_Class_18/1  "<OBJ_Class_18>"
  Bus Selector:RadarSensor:3_OBJ_Class_BS/19 -> RadarSensor:3.OBJ_Class_19/1  "<OBJ_Class_19>"
  Bus Selector:RadarSensor:3_OBJ_Class_BS/20 -> RadarSensor:3.OBJ_Class_20/1  "<OBJ_Class_20>"
  Bus Selector:RadarSensor:3_OBJ_Class_BS/21 -> RadarSensor:3.OBJ_Class_21/1  "<OBJ_Class_21>"
  Bus Selector:RadarSensor:3_OBJ_Class_BS/22 -> RadarSensor:3.OBJ_Class_22/1  "<OBJ_Class_22>"
  Bus Selector:RadarSensor:3_OBJ_Class_BS/23 -> RadarSensor:3.OBJ_Class_23/1  "<OBJ_Class_23>"
  Bus Selector:RadarSensor:3_OBJ_Class_BS/24 -> RadarSensor:3.OBJ_Class_24/1  "<OBJ_Class_24>"
  Bus Selector:RadarSensor:3_OBJ_Class_BS/25 -> RadarSensor:3.OBJ_Class_25/1  "<OBJ_Class_25>"
  Bus Selector:RadarSensor:3_OBJ_Class_BS/26 -> RadarSensor:3.OBJ_Class_26/1  "<OBJ_Class_26>"
  Bus Selector:RadarSensor:3_OBJ_Class_BS/27 -> RadarSensor:3.OBJ_Class_27/1  "<OBJ_Class_27>"
  Bus Selector:RadarSensor:3_OBJ_Class_BS/28 -> RadarSensor:3.OBJ_Class_28/1  "<OBJ_Class_28>"
  Bus Selector:RadarSensor:3_OBJ_Class_BS/29 -> RadarSensor:3.OBJ_Class_29/1  "<OBJ_Class_29>"
  Bus Selector:RadarSensor:3_OBJ_Class_BS/30 -> RadarSensor:3.OBJ_Class_30/1  "<OBJ_Class_30>"
  Bus Selector:RadarSensor:3_OBJ_Class_BS/31 -> RadarSensor:3.OBJ_Class_31/1  "<OBJ_Class_31>"
  Bus Selector:RadarSensor:3_OBJ_Class_BS/32 -> RadarSensor:3.OBJ_Class_32/1  "<OBJ_Class_32>"
  Bus Selector:RadarSensor:3_OBJ_Class_BS/33 -> RadarSensor:3.OBJ_Class_33/1  "<OBJ_Class_33>"
  Bus Selector:RadarSensor:3_OBJ_Class_BS/34 -> RadarSensor:3.OBJ_Class_34/1  "<OBJ_Class_34>"
  Bus Selector:RadarSensor:3_OBJ_Class_BS/35 -> RadarSensor:3.OBJ_Class_35/1  "<OBJ_Class_35>"
  Bus Selector:RadarSensor:3_OBJ_Class_BS/36 -> RadarSensor:3.OBJ_Class_36/1  "<OBJ_Class_36>"
  Bus Selector:RadarSensor:3_OBJ_Class_BS/37 -> RadarSensor:3.OBJ_Class_37/1  "<OBJ_Class_37>"
  Bus Selector:RadarSensor:3_OBJ_Class_BS/38 -> RadarSensor:3.OBJ_Class_38/1  "<OBJ_Class_38>"
  Bus Selector:RadarSensor:3_OBJ_Class_BS/39 -> RadarSensor:3.OBJ_Class_39/1  "<OBJ_Class_39>"
  Bus Selector:RadarSensor:3_OBJ_Class_BS/40 -> RadarSensor:3.OBJ_Class_40/1  "<OBJ_Class_40>"
  Bus Selector:RadarSensor:3_OBJ_Class_BS/41 -> RadarSensor:3.OBJ_Class_41/1  "<OBJ_Class_41>"
  Bus Selector:RadarSensor:3_OBJ_Class_BS/42 -> RadarSensor:3.OBJ_Class_42/1  "<OBJ_Class_42>"
  Bus Selector:RadarSensor:3_OBJ_Class_BS/43 -> RadarSensor:3.OBJ_Class_43/1  "<OBJ_Class_43>"
  Bus Selector:RadarSensor:3_OBJ_Class_BS/44 -> RadarSensor:3.OBJ_Class_44/1  "<OBJ_Class_44>"
  Bus Selector:RadarSensor:3_OBJ_Class_BS/45 -> RadarSensor:3.OBJ_Class_45/1  "<OBJ_Class_45>"
  Bus Selector:RadarSensor:3_OBJ_Class_BS/46 -> RadarSensor:3.OBJ_Class_46/1  "<OBJ_Class_46>"
  Bus Selector:RadarSensor:3_OBJ_Class_BS/47 -> RadarSensor:3.OBJ_Class_47/1  "<OBJ_Class_47>"
  Bus Selector:RadarSensor:3_OBJ_Class_BS/48 -> RadarSensor:3.OBJ_Class_48/1  "<OBJ_Class_48>"
  Bus Selector:RadarSensor:3_OBJ_Class_BS/49 -> RadarSensor:3.OBJ_Class_49/1  "<OBJ_Class_49>"
  Bus Selector:RadarSensor:3_OBJ_Class_BS/50 -> RadarSensor:3.OBJ_Class_50/1  "<OBJ_Class_50>"
  Bus Selector:RadarSensor:3_OBJ_Class_BS/51 -> RadarSensor:3.OBJ_Class_51/1  "<OBJ_Class_51>"
  Bus Selector:RadarSensor:3_OBJ_Class_BS/52 -> RadarSensor:3.OBJ_Class_52/1  "<OBJ_Class_52>"
  Bus Selector:RadarSensor:3_OBJ_Class_BS/53 -> RadarSensor:3.OBJ_Class_53/1  "<OBJ_Class_53>"
  Bus Selector:RadarSensor:3_OBJ_Class_BS/54 -> RadarSensor:3.OBJ_Class_54/1  "<OBJ_Class_54>"
  Bus Selector:RadarSensor:3_OBJ_Class_BS/55 -> RadarSensor:3.OBJ_Class_55/1  "<OBJ_Class_55>"
  Bus Selector:RadarSensor:3_OBJ_Class_BS/56 -> RadarSensor:3.OBJ_Class_56/1  "<OBJ_Class_56>"
  Bus Selector:RadarSensor:3_OBJ_Class_BS/57 -> RadarSensor:3.OBJ_Class_57/1  "<OBJ_Class_57>"
  Bus Selector:RadarSensor:3_OBJ_Class_BS/58 -> RadarSensor:3.OBJ_Class_58/1  "<OBJ_Class_58>"
  Bus Selector:RadarSensor:3_OBJ_Class_BS/59 -> RadarSensor:3.OBJ_Class_59/1  "<OBJ_Class_59>"
  Bus Selector:RadarSensor:3_OBJ_Class_BS/60 -> RadarSensor:3.OBJ_Class_60/1  "<OBJ_Class_60>"
  Bus Selector:RadarSensor:3_OBJ_Class_BS/61 -> RadarSensor:3.OBJ_Class_61/1  "<OBJ_Class_61>"
  Bus Selector:RadarSensor:3_OBJ_Class_BS/62 -> RadarSensor:3.OBJ_Class_62/1  "<OBJ_Class_62>"
  Bus Selector:RadarSensor:3_OBJ_Class_BS/63 -> RadarSensor:3.OBJ_Class_63/1  "<OBJ_Class_63>"
  Bus Selector:RadarSensor:3_OBJ_Class_BS/64 -> RadarSensor:3.OBJ_Class_64/1  "<OBJ_Class_64>"
  Bus Selector:RadarSensor:3_OBJ_S_Azimuth_BS/1 -> RadarSensor:3.OBJ_S_Azimuth_1/1  "<OBJ_S_Azimuth_1>"
  Bus Selector:RadarSensor:3_OBJ_S_Azimuth_BS/2 -> RadarSensor:3.OBJ_S_Azimuth_2/1  "<OBJ_S_Azimuth_2>"
  Bus Selector:RadarSensor:3_OBJ_S_Azimuth_BS/3 -> RadarSensor:3.OBJ_S_Azimuth_3/1  "<OBJ_S_Azimuth_3>"
  Bus Selector:RadarSensor:3_OBJ_S_Azimuth_BS/4 -> RadarSensor:3.OBJ_S_Azimuth_4/1  "<OBJ_S_Azimuth_4>"
  Bus Selector:RadarSensor:3_OBJ_S_Azimuth_BS/5 -> RadarSensor:3.OBJ_S_Azimuth_5/1  "<OBJ_S_Azimuth_5>"
  Bus Selector:RadarSensor:3_OBJ_S_Azimuth_BS/6 -> RadarSensor:3.OBJ_S_Azimuth_6/1  "<OBJ_S_Azimuth_6>"
  Bus Selector:RadarSensor:3_OBJ_S_Azimuth_BS/7 -> RadarSensor:3.OBJ_S_Azimuth_7/1  "<OBJ_S_Azimuth_7>"
  Bus Selector:RadarSensor:3_OBJ_S_Azimuth_BS/8 -> RadarSensor:3.OBJ_S_Azimuth_8/1  "<OBJ_S_Azimuth_8>"
  Bus Selector:RadarSensor:3_OBJ_S_Azimuth_BS/9 -> RadarSensor:3.OBJ_S_Azimuth_9/1  "<OBJ_S_Azimuth_9>"
  Bus Selector:RadarSensor:3_OBJ_S_Azimuth_BS/10 -> RadarSensor:3.OBJ_S_Azimuth_10/1  "<OBJ_S_Azimuth_10>"
  Bus Selector:RadarSensor:3_OBJ_S_Azimuth_BS/11 -> RadarSensor:3.OBJ_S_Azimuth_11/1  "<OBJ_S_Azimuth_11>"
  Bus Selector:RadarSensor:3_OBJ_S_Azimuth_BS/12 -> RadarSensor:3.OBJ_S_Azimuth_12/1  "<OBJ_S_Azimuth_12>"
  Bus Selector:RadarSensor:3_OBJ_S_Azimuth_BS/13 -> RadarSensor:3.OBJ_S_Azimuth_13/1  "<OBJ_S_Azimuth_13>"
  Bus Selector:RadarSensor:3_OBJ_S_Azimuth_BS/14 -> RadarSensor:3.OBJ_S_Azimuth_14/1  "<OBJ_S_Azimuth_14>"
  Bus Selector:RadarSensor:3_OBJ_S_Azimuth_BS/15 -> RadarSensor:3.OBJ_S_Azimuth_15/1  "<OBJ_S_Azimuth_15>"
  Bus Selector:RadarSensor:3_OBJ_S_Azimuth_BS/16 -> RadarSensor:3.OBJ_S_Azimuth_16/1  "<OBJ_S_Azimuth_16>"
  Bus Selector:RadarSensor:3_OBJ_S_Azimuth_BS/17 -> RadarSensor:3.OBJ_S_Azimuth_17/1  "<OBJ_S_Azimuth_17>"
  Bus Selector:RadarSensor:3_OBJ_S_Azimuth_BS/18 -> RadarSensor:3.OBJ_S_Azimuth_18/1  "<OBJ_S_Azimuth_18>"
  Bus Selector:RadarSensor:3_OBJ_S_Azimuth_BS/19 -> RadarSensor:3.OBJ_S_Azimuth_19/1  "<OBJ_S_Azimuth_19>"
  Bus Selector:RadarSensor:3_OBJ_S_Azimuth_BS/20 -> RadarSensor:3.OBJ_S_Azimuth_20/1  "<OBJ_S_Azimuth_20>"
  Bus Selector:RadarSensor:3_OBJ_S_Azimuth_BS/21 -> RadarSensor:3.OBJ_S_Azimuth_21/1  "<OBJ_S_Azimuth_21>"
  Bus Selector:RadarSensor:3_OBJ_S_Azimuth_BS/22 -> RadarSensor:3.OBJ_S_Azimuth_22/1  "<OBJ_S_Azimuth_22>"
  Bus Selector:RadarSensor:3_OBJ_S_Azimuth_BS/23 -> RadarSensor:3.OBJ_S_Azimuth_23/1  "<OBJ_S_Azimuth_23>"
  Bus Selector:RadarSensor:3_OBJ_S_Azimuth_BS/24 -> RadarSensor:3.OBJ_S_Azimuth_24/1  "<OBJ_S_Azimuth_24>"
  Bus Selector:RadarSensor:3_OBJ_S_Azimuth_BS/25 -> RadarSensor:3.OBJ_S_Azimuth_25/1  "<OBJ_S_Azimuth_25>"
  Bus Selector:RadarSensor:3_OBJ_S_Azimuth_BS/26 -> RadarSensor:3.OBJ_S_Azimuth_26/1  "<OBJ_S_Azimuth_26>"
  Bus Selector:RadarSensor:3_OBJ_S_Azimuth_BS/27 -> RadarSensor:3.OBJ_S_Azimuth_27/1  "<OBJ_S_Azimuth_27>"
  Bus Selector:RadarSensor:3_OBJ_S_Azimuth_BS/28 -> RadarSensor:3.OBJ_S_Azimuth_28/1  "<OBJ_S_Azimuth_28>"
  Bus Selector:RadarSensor:3_OBJ_S_Azimuth_BS/29 -> RadarSensor:3.OBJ_S_Azimuth_29/1  "<OBJ_S_Azimuth_29>"
  Bus Selector:RadarSensor:3_OBJ_S_Azimuth_BS/30 -> RadarSensor:3.OBJ_S_Azimuth_30/1  "<OBJ_S_Azimuth_30>"
  Bus Selector:RadarSensor:3_OBJ_S_Azimuth_BS/31 -> RadarSensor:3.OBJ_S_Azimuth_31/1  "<OBJ_S_Azimuth_31>"
  Bus Selector:RadarSensor:3_OBJ_S_Azimuth_BS/32 -> RadarSensor:3.OBJ_S_Azimuth_32/1  "<OBJ_S_Azimuth_32>"
  Bus Selector:RadarSensor:3_OBJ_S_Azimuth_BS/33 -> RadarSensor:3.OBJ_S_Azimuth_33/1  "<OBJ_S_Azimuth_33>"
  Bus Selector:RadarSensor:3_OBJ_S_Azimuth_BS/34 -> RadarSensor:3.OBJ_S_Azimuth_34/1  "<OBJ_S_Azimuth_34>"
  Bus Selector:RadarSensor:3_OBJ_S_Azimuth_BS/35 -> RadarSensor:3.OBJ_S_Azimuth_35/1  "<OBJ_S_Azimuth_35>"
  Bus Selector:RadarSensor:3_OBJ_S_Azimuth_BS/36 -> RadarSensor:3.OBJ_S_Azimuth_36/1  "<OBJ_S_Azimuth_36>"
  Bus Selector:RadarSensor:3_OBJ_S_Azimuth_BS/37 -> RadarSensor:3.OBJ_S_Azimuth_37/1  "<OBJ_S_Azimuth_37>"
  Bus Selector:RadarSensor:3_OBJ_S_Azimuth_BS/38 -> RadarSensor:3.OBJ_S_Azimuth_38/1  "<OBJ_S_Azimuth_38>"
  Bus Selector:RadarSensor:3_OBJ_S_Azimuth_BS/39 -> RadarSensor:3.OBJ_S_Azimuth_39/1  "<OBJ_S_Azimuth_39>"
  Bus Selector:RadarSensor:3_OBJ_S_Azimuth_BS/40 -> RadarSensor:3.OBJ_S_Azimuth_40/1  "<OBJ_S_Azimuth_40>"
  Bus Selector:RadarSensor:3_OBJ_S_Azimuth_BS/41 -> RadarSensor:3.OBJ_S_Azimuth_41/1  "<OBJ_S_Azimuth_41>"
  Bus Selector:RadarSensor:3_OBJ_S_Azimuth_BS/42 -> RadarSensor:3.OBJ_S_Azimuth_42/1  "<OBJ_S_Azimuth_42>"
  Bus Selector:RadarSensor:3_OBJ_S_Azimuth_BS/43 -> RadarSensor:3.OBJ_S_Azimuth_43/1  "<OBJ_S_Azimuth_43>"
  Bus Selector:RadarSensor:3_OBJ_S_Azimuth_BS/44 -> RadarSensor:3.OBJ_S_Azimuth_44/1  "<OBJ_S_Azimuth_44>"
  Bus Selector:RadarSensor:3_OBJ_S_Azimuth_BS/45 -> RadarSensor:3.OBJ_S_Azimuth_45/1  "<OBJ_S_Azimuth_45>"
  Bus Selector:RadarSensor:3_OBJ_S_Azimuth_BS/46 -> RadarSensor:3.OBJ_S_Azimuth_46/1  "<OBJ_S_Azimuth_46>"
  Bus Selector:RadarSensor:3_OBJ_S_Azimuth_BS/47 -> RadarSensor:3.OBJ_S_Azimuth_47/1  "<OBJ_S_Azimuth_47>"
  Bus Selector:RadarSensor:3_OBJ_S_Azimuth_BS/48 -> RadarSensor:3.OBJ_S_Azimuth_48/1  "<OBJ_S_Azimuth_48>"
  Bus Selector:RadarSensor:3_OBJ_S_Azimuth_BS/49 -> RadarSensor:3.OBJ_S_Azimuth_49/1  "<OBJ_S_Azimuth_49>"
  Bus Selector:RadarSensor:3_OBJ_S_Azimuth_BS/50 -> RadarSensor:3.OBJ_S_Azimuth_50/1  "<OBJ_S_Azimuth_50>"
  Bus Selector:RadarSensor:3_OBJ_S_Azimuth_BS/51 -> RadarSensor:3.OBJ_S_Azimuth_51/1  "<OBJ_S_Azimuth_51>"
  Bus Selector:RadarSensor:3_OBJ_S_Azimuth_BS/52 -> RadarSensor:3.OBJ_S_Azimuth_52/1  "<OBJ_S_Azimuth_52>"
  Bus Selector:RadarSensor:3_OBJ_S_Azimuth_BS/53 -> RadarSensor:3.OBJ_S_Azimuth_53/1  "<OBJ_S_Azimuth_53>"
  Bus Selector:RadarSensor:3_OBJ_S_Azimuth_BS/54 -> RadarSensor:3.OBJ_S_Azimuth_54/1  "<OBJ_S_Azimuth_54>"
  Bus Selector:RadarSensor:3_OBJ_S_Azimuth_BS/55 -> RadarSensor:3.OBJ_S_Azimuth_55/1  "<OBJ_S_Azimuth_55>"
  Bus Selector:RadarSensor:3_OBJ_S_Azimuth_BS/56 -> RadarSensor:3.OBJ_S_Azimuth_56/1  "<OBJ_S_Azimuth_56>"
  Bus Selector:RadarSensor:3_OBJ_S_Azimuth_BS/57 -> RadarSensor:3.OBJ_S_Azimuth_57/1  "<OBJ_S_Azimuth_57>"
  Bus Selector:RadarSensor:3_OBJ_S_Azimuth_BS/58 -> RadarSensor:3.OBJ_S_Azimuth_58/1  "<OBJ_S_Azimuth_58>"
  Bus Selector:RadarSensor:3_OBJ_S_Azimuth_BS/59 -> RadarSensor:3.OBJ_S_Azimuth_59/1  "<OBJ_S_Azimuth_59>"
  Bus Selector:RadarSensor:3_OBJ_S_Azimuth_BS/60 -> RadarSensor:3.OBJ_S_Azimuth_60/1  "<OBJ_S_Azimuth_60>"
  Bus Selector:RadarSensor:3_OBJ_S_Azimuth_BS/61 -> RadarSensor:3.OBJ_S_Azimuth_61/1  "<OBJ_S_Azimuth_61>"
  Bus Selector:RadarSensor:3_OBJ_S_Azimuth_BS/62 -> RadarSensor:3.OBJ_S_Azimuth_62/1  "<OBJ_S_Azimuth_62>"
  Bus Selector:RadarSensor:3_OBJ_S_Azimuth_BS/63 -> RadarSensor:3.OBJ_S_Azimuth_63/1  "<OBJ_S_Azimuth_63>"
  Bus Selector:RadarSensor:3_OBJ_S_Azimuth_BS/64 -> RadarSensor:3.OBJ_S_Azimuth_64/1  "<OBJ_S_Azimuth_64>"
  Bus Selector:RadarSensor:3_OBJ_S_Elevation_BS/1 -> RadarSensor:3.OBJ_S_Elevation_1/1  "<OBJ_S_Elevation_1>"
  Bus Selector:RadarSensor:3_OBJ_S_Elevation_BS/2 -> RadarSensor:3.OBJ_S_Elevation_2/1  "<OBJ_S_Elevation_2>"
  Bus Selector:RadarSensor:3_OBJ_S_Elevation_BS/3 -> RadarSensor:3.OBJ_S_Elevation_3/1  "<OBJ_S_Elevation_3>"
  Bus Selector:RadarSensor:3_OBJ_S_Elevation_BS/4 -> RadarSensor:3.OBJ_S_Elevation_4/1  "<OBJ_S_Elevation_4>"
  Bus Selector:RadarSensor:3_OBJ_S_Elevation_BS/5 -> RadarSensor:3.OBJ_S_Elevation_5/1  "<OBJ_S_Elevation_5>"
  Bus Selector:RadarSensor:3_OBJ_S_Elevation_BS/6 -> RadarSensor:3.OBJ_S_Elevation_6/1  "<OBJ_S_Elevation_6>"
  Bus Selector:RadarSensor:3_OBJ_S_Elevation_BS/7 -> RadarSensor:3.OBJ_S_Elevation_7/1  "<OBJ_S_Elevation_7>"
  Bus Selector:RadarSensor:3_OBJ_S_Elevation_BS/8 -> RadarSensor:3.OBJ_S_Elevation_8/1  "<OBJ_S_Elevation_8>"
  Bus Selector:RadarSensor:3_OBJ_S_Elevation_BS/9 -> RadarSensor:3.OBJ_S_Elevation_9/1  "<OBJ_S_Elevation_9>"
  Bus Selector:RadarSensor:3_OBJ_S_Elevation_BS/10 -> RadarSensor:3.OBJ_S_Elevation_10/1  "<OBJ_S_Elevation_10>"
  Bus Selector:RadarSensor:3_OBJ_S_Elevation_BS/11 -> RadarSensor:3.OBJ_S_Elevation_11/1  "<OBJ_S_Elevation_11>"
  Bus Selector:RadarSensor:3_OBJ_S_Elevation_BS/12 -> RadarSensor:3.OBJ_S_Elevation_12/1  "<OBJ_S_Elevation_12>"
  Bus Selector:RadarSensor:3_OBJ_S_Elevation_BS/13 -> RadarSensor:3.OBJ_S_Elevation_13/1  "<OBJ_S_Elevation_13>"
  Bus Selector:RadarSensor:3_OBJ_S_Elevation_BS/14 -> RadarSensor:3.OBJ_S_Elevation_14/1  "<OBJ_S_Elevation_14>"
  Bus Selector:RadarSensor:3_OBJ_S_Elevation_BS/15 -> RadarSensor:3.OBJ_S_Elevation_15/1  "<OBJ_S_Elevation_15>"
  Bus Selector:RadarSensor:3_OBJ_S_Elevation_BS/16 -> RadarSensor:3.OBJ_S_Elevation_16/1  "<OBJ_S_Elevation_16>"
  Bus Selector:RadarSensor:3_OBJ_S_Elevation_BS/17 -> RadarSensor:3.OBJ_S_Elevation_17/1  "<OBJ_S_Elevation_17>"
  Bus Selector:RadarSensor:3_OBJ_S_Elevation_BS/18 -> RadarSensor:3.OBJ_S_Elevation_18/1  "<OBJ_S_Elevation_18>"
  Bus Selector:RadarSensor:3_OBJ_S_Elevation_BS/19 -> RadarSensor:3.OBJ_S_Elevation_19/1  "<OBJ_S_Elevation_19>"
  Bus Selector:RadarSensor:3_OBJ_S_Elevation_BS/20 -> RadarSensor:3.OBJ_S_Elevation_20/1  "<OBJ_S_Elevation_20>"
  Bus Selector:RadarSensor:3_OBJ_S_Elevation_BS/21 -> RadarSensor:3.OBJ_S_Elevation_21/1  "<OBJ_S_Elevation_21>"
  Bus Selector:RadarSensor:3_OBJ_S_Elevation_BS/22 -> RadarSensor:3.OBJ_S_Elevation_22/1  "<OBJ_S_Elevation_22>"
  Bus Selector:RadarSensor:3_OBJ_S_Elevation_BS/23 -> RadarSensor:3.OBJ_S_Elevation_23/1  "<OBJ_S_Elevation_23>"
  Bus Selector:RadarSensor:3_OBJ_S_Elevation_BS/24 -> RadarSensor:3.OBJ_S_Elevation_24/1  "<OBJ_S_Elevation_24>"
  Bus Selector:RadarSensor:3_OBJ_S_Elevation_BS/25 -> RadarSensor:3.OBJ_S_Elevation_25/1  "<OBJ_S_Elevation_25>"
  Bus Selector:RadarSensor:3_OBJ_S_Elevation_BS/26 -> RadarSensor:3.OBJ_S_Elevation_26/1  "<OBJ_S_Elevation_26>"
  Bus Selector:RadarSensor:3_OBJ_S_Elevation_BS/27 -> RadarSensor:3.OBJ_S_Elevation_27/1  "<OBJ_S_Elevation_27>"
  Bus Selector:RadarSensor:3_OBJ_S_Elevation_BS/28 -> RadarSensor:3.OBJ_S_Elevation_28/1  "<OBJ_S_Elevation_28>"
  Bus Selector:RadarSensor:3_OBJ_S_Elevation_BS/29 -> RadarSensor:3.OBJ_S_Elevation_29/1  "<OBJ_S_Elevation_29>"
  Bus Selector:RadarSensor:3_OBJ_S_Elevation_BS/30 -> RadarSensor:3.OBJ_S_Elevation_30/1  "<OBJ_S_Elevation_30>"
  Bus Selector:RadarSensor:3_OBJ_S_Elevation_BS/31 -> RadarSensor:3.OBJ_S_Elevation_31/1  "<OBJ_S_Elevation_31>"
  Bus Selector:RadarSensor:3_OBJ_S_Elevation_BS/32 -> RadarSensor:3.OBJ_S_Elevation_32/1  "<OBJ_S_Elevation_32>"
  Bus Selector:RadarSensor:3_OBJ_S_Elevation_BS/33 -> RadarSensor:3.OBJ_S_Elevation_33/1  "<OBJ_S_Elevation_33>"
  Bus Selector:RadarSensor:3_OBJ_S_Elevation_BS/34 -> RadarSensor:3.OBJ_S_Elevation_34/1  "<OBJ_S_Elevation_34>"
  Bus Selector:RadarSensor:3_OBJ_S_Elevation_BS/35 -> RadarSensor:3.OBJ_S_Elevation_35/1  "<OBJ_S_Elevation_35>"
  Bus Selector:RadarSensor:3_OBJ_S_Elevation_BS/36 -> RadarSensor:3.OBJ_S_Elevation_36/1  "<OBJ_S_Elevation_36>"
  Bus Selector:RadarSensor:3_OBJ_S_Elevation_BS/37 -> RadarSensor:3.OBJ_S_Elevation_37/1  "<OBJ_S_Elevation_37>"
  Bus Selector:RadarSensor:3_OBJ_S_Elevation_BS/38 -> RadarSensor:3.OBJ_S_Elevation_38/1  "<OBJ_S_Elevation_38>"
  Bus Selector:RadarSensor:3_OBJ_S_Elevation_BS/39 -> RadarSensor:3.OBJ_S_Elevation_39/1  "<OBJ_S_Elevation_39>"
  Bus Selector:RadarSensor:3_OBJ_S_Elevation_BS/40 -> RadarSensor:3.OBJ_S_Elevation_40/1  "<OBJ_S_Elevation_40>"
  Bus Selector:RadarSensor:3_OBJ_S_Elevation_BS/41 -> RadarSensor:3.OBJ_S_Elevation_41/1  "<OBJ_S_Elevation_41>"
  Bus Selector:RadarSensor:3_OBJ_S_Elevation_BS/42 -> RadarSensor:3.OBJ_S_Elevation_42/1  "<OBJ_S_Elevation_42>"
  Bus Selector:RadarSensor:3_OBJ_S_Elevation_BS/43 -> RadarSensor:3.OBJ_S_Elevation_43/1  "<OBJ_S_Elevation_43>"
  Bus Selector:RadarSensor:3_OBJ_S_Elevation_BS/44 -> RadarSensor:3.OBJ_S_Elevation_44/1  "<OBJ_S_Elevation_44>"
  Bus Selector:RadarSensor:3_OBJ_S_Elevation_BS/45 -> RadarSensor:3.OBJ_S_Elevation_45/1  "<OBJ_S_Elevation_45>"
  Bus Selector:RadarSensor:3_OBJ_S_Elevation_BS/46 -> RadarSensor:3.OBJ_S_Elevation_46/1  "<OBJ_S_Elevation_46>"
  Bus Selector:RadarSensor:3_OBJ_S_Elevation_BS/47 -> RadarSensor:3.OBJ_S_Elevation_47/1  "<OBJ_S_Elevation_47>"
  Bus Selector:RadarSensor:3_OBJ_S_Elevation_BS/48 -> RadarSensor:3.OBJ_S_Elevation_48/1  "<OBJ_S_Elevation_48>"
  Bus Selector:RadarSensor:3_OBJ_S_Elevation_BS/49 -> RadarSensor:3.OBJ_S_Elevation_49/1  "<OBJ_S_Elevation_49>"
  Bus Selector:RadarSensor:3_OBJ_S_Elevation_BS/50 -> RadarSensor:3.OBJ_S_Elevation_50/1  "<OBJ_S_Elevation_50>"
  Bus Selector:RadarSensor:3_OBJ_S_Elevation_BS/51 -> RadarSensor:3.OBJ_S_Elevation_51/1  "<OBJ_S_Elevation_51>"
  Bus Selector:RadarSensor:3_OBJ_S_Elevation_BS/52 -> RadarSensor:3.OBJ_S_Elevation_52/1  "<OBJ_S_Elevation_52>"
  Bus Selector:RadarSensor:3_OBJ_S_Elevation_BS/53 -> RadarSensor:3.OBJ_S_Elevation_53/1  "<OBJ_S_Elevation_53>"
  Bus Selector:RadarSensor:3_OBJ_S_Elevation_BS/54 -> RadarSensor:3.OBJ_S_Elevation_54/1  "<OBJ_S_Elevation_54>"
  Bus Selector:RadarSensor:3_OBJ_S_Elevation_BS/55 -> RadarSensor:3.OBJ_S_Elevation_55/1  "<OBJ_S_Elevation_55>"
  Bus Selector:RadarSensor:3_OBJ_S_Elevation_BS/56 -> RadarSensor:3.OBJ_S_Elevation_56/1  "<OBJ_S_Elevation_56>"
  Bus Selector:RadarSensor:3_OBJ_S_Elevation_BS/57 -> RadarSensor:3.OBJ_S_Elevation_57/1  "<OBJ_S_Elevation_57>"
  Bus Selector:RadarSensor:3_OBJ_S_Elevation_BS/58 -> RadarSensor:3.OBJ_S_Elevation_58/1  "<OBJ_S_Elevation_58>"
  Bus Selector:RadarSensor:3_OBJ_S_Elevation_BS/59 -> RadarSensor:3.OBJ_S_Elevation_59/1  "<OBJ_S_Elevation_59>"
  Bus Selector:RadarSensor:3_OBJ_S_Elevation_BS/60 -> RadarSensor:3.OBJ_S_Elevation_60/1  "<OBJ_S_Elevation_60>"
  Bus Selector:RadarSensor:3_OBJ_S_Elevation_BS/61 -> RadarSensor:3.OBJ_S_Elevation_61/1  "<OBJ_S_Elevation_61>"
  Bus Selector:RadarSensor:3_OBJ_S_Elevation_BS/62 -> RadarSensor:3.OBJ_S_Elevation_62/1  "<OBJ_S_Elevation_62>"
  Bus Selector:RadarSensor:3_OBJ_S_Elevation_BS/63 -> RadarSensor:3.OBJ_S_Elevation_63/1  "<OBJ_S_Elevation_63>"
  Bus Selector:RadarSensor:3_OBJ_S_Elevation_BS/64 -> RadarSensor:3.OBJ_S_Elevation_64/1  "<OBJ_S_Elevation_64>"
  Bus Selector:RadarSensor:3_OBJ_S_Velocity_BS/1 -> RadarSensor:3.OBJ_S_Velocity_1/1  "<OBJ_S_Velocity_1>"
  Bus Selector:RadarSensor:3_OBJ_S_Velocity_BS/2 -> RadarSensor:3.OBJ_S_Velocity_2/1  "<OBJ_S_Velocity_2>"
  Bus Selector:RadarSensor:3_OBJ_S_Velocity_BS/3 -> RadarSensor:3.OBJ_S_Velocity_3/1  "<OBJ_S_Velocity_3>"
  Bus Selector:RadarSensor:3_OBJ_S_Velocity_BS/4 -> RadarSensor:3.OBJ_S_Velocity_4/1  "<OBJ_S_Velocity_4>"
  Bus Selector:RadarSensor:3_OBJ_S_Velocity_BS/5 -> RadarSensor:3.OBJ_S_Velocity_5/1  "<OBJ_S_Velocity_5>"
  Bus Selector:RadarSensor:3_OBJ_S_Velocity_BS/6 -> RadarSensor:3.OBJ_S_Velocity_6/1  "<OBJ_S_Velocity_6>"
  Bus Selector:RadarSensor:3_OBJ_S_Velocity_BS/7 -> RadarSensor:3.OBJ_S_Velocity_7/1  "<OBJ_S_Velocity_7>"
  Bus Selector:RadarSensor:3_OBJ_S_Velocity_BS/8 -> RadarSensor:3.OBJ_S_Velocity_8/1  "<OBJ_S_Velocity_8>"
  Bus Selector:RadarSensor:3_OBJ_S_Velocity_BS/9 -> RadarSensor:3.OBJ_S_Velocity_9/1  "<OBJ_S_Velocity_9>"
  Bus Selector:RadarSensor:3_OBJ_S_Velocity_BS/10 -> RadarSensor:3.OBJ_S_Velocity_10/1  "<OBJ_S_Velocity_10>"
  Bus Selector:RadarSensor:3_OBJ_S_Velocity_BS/11 -> RadarSensor:3.OBJ_S_Velocity_11/1  "<OBJ_S_Velocity_11>"
  Bus Selector:RadarSensor:3_OBJ_S_Velocity_BS/12 -> RadarSensor:3.OBJ_S_Velocity_12/1  "<OBJ_S_Velocity_12>"
  Bus Selector:RadarSensor:3_OBJ_S_Velocity_BS/13 -> RadarSensor:3.OBJ_S_Velocity_13/1  "<OBJ_S_Velocity_13>"
  Bus Selector:RadarSensor:3_OBJ_S_Velocity_BS/14 -> RadarSensor:3.OBJ_S_Velocity_14/1  "<OBJ_S_Velocity_14>"
  Bus Selector:RadarSensor:3_OBJ_S_Velocity_BS/15 -> RadarSensor:3.OBJ_S_Velocity_15/1  "<OBJ_S_Velocity_15>"
  Bus Selector:RadarSensor:3_OBJ_S_Velocity_BS/16 -> RadarSensor:3.OBJ_S_Velocity_16/1  "<OBJ_S_Velocity_16>"
  Bus Selector:RadarSensor:3_OBJ_S_Velocity_BS/17 -> RadarSensor:3.OBJ_S_Velocity_17/1  "<OBJ_S_Velocity_17>"
  Bus Selector:RadarSensor:3_OBJ_S_Velocity_BS/18 -> RadarSensor:3.OBJ_S_Velocity_18/1  "<OBJ_S_Velocity_18>"
  Bus Selector:RadarSensor:3_OBJ_S_Velocity_BS/19 -> RadarSensor:3.OBJ_S_Velocity_19/1  "<OBJ_S_Velocity_19>"
  Bus Selector:RadarSensor:3_OBJ_S_Velocity_BS/20 -> RadarSensor:3.OBJ_S_Velocity_20/1  "<OBJ_S_Velocity_20>"
  Bus Selector:RadarSensor:3_OBJ_S_Velocity_BS/21 -> RadarSensor:3.OBJ_S_Velocity_21/1  "<OBJ_S_Velocity_21>"
  Bus Selector:RadarSensor:3_OBJ_S_Velocity_BS/22 -> RadarSensor:3.OBJ_S_Velocity_22/1  "<OBJ_S_Velocity_22>"
  Bus Selector:RadarSensor:3_OBJ_S_Velocity_BS/23 -> RadarSensor:3.OBJ_S_Velocity_23/1  "<OBJ_S_Velocity_23>"
  Bus Selector:RadarSensor:3_OBJ_S_Velocity_BS/24 -> RadarSensor:3.OBJ_S_Velocity_24/1  "<OBJ_S_Velocity_24>"
  Bus Selector:RadarSensor:3_OBJ_S_Velocity_BS/25 -> RadarSensor:3.OBJ_S_Velocity_25/1  "<OBJ_S_Velocity_25>"
  Bus Selector:RadarSensor:3_OBJ_S_Velocity_BS/26 -> RadarSensor:3.OBJ_S_Velocity_26/1  "<OBJ_S_Velocity_26>"
  Bus Selector:RadarSensor:3_OBJ_S_Velocity_BS/27 -> RadarSensor:3.OBJ_S_Velocity_27/1  "<OBJ_S_Velocity_27>"
  Bus Selector:RadarSensor:3_OBJ_S_Velocity_BS/28 -> RadarSensor:3.OBJ_S_Velocity_28/1  "<OBJ_S_Velocity_28>"
  Bus Selector:RadarSensor:3_OBJ_S_Velocity_BS/29 -> RadarSensor:3.OBJ_S_Velocity_29/1  "<OBJ_S_Velocity_29>"
  Bus Selector:RadarSensor:3_OBJ_S_Velocity_BS/30 -> RadarSensor:3.OBJ_S_Velocity_30/1  "<OBJ_S_Velocity_30>"
  Bus Selector:RadarSensor:3_OBJ_S_Velocity_BS/31 -> RadarSensor:3.OBJ_S_Velocity_31/1  "<OBJ_S_Velocity_31>"
  Bus Selector:RadarSensor:3_OBJ_S_Velocity_BS/32 -> RadarSensor:3.OBJ_S_Velocity_32/1  "<OBJ_S_Velocity_32>"
  Bus Selector:RadarSensor:3_OBJ_S_Velocity_BS/33 -> RadarSensor:3.OBJ_S_Velocity_33/1  "<OBJ_S_Velocity_33>"
  Bus Selector:RadarSensor:3_OBJ_S_Velocity_BS/34 -> RadarSensor:3.OBJ_S_Velocity_34/1  "<OBJ_S_Velocity_34>"
  Bus Selector:RadarSensor:3_OBJ_S_Velocity_BS/35 -> RadarSensor:3.OBJ_S_Velocity_35/1  "<OBJ_S_Velocity_35>"
  Bus Selector:RadarSensor:3_OBJ_S_Velocity_BS/36 -> RadarSensor:3.OBJ_S_Velocity_36/1  "<OBJ_S_Velocity_36>"
  Bus Selector:RadarSensor:3_OBJ_S_Velocity_BS/37 -> RadarSensor:3.OBJ_S_Velocity_37/1  "<OBJ_S_Velocity_37>"
  Bus Selector:RadarSensor:3_OBJ_S_Velocity_BS/38 -> RadarSensor:3.OBJ_S_Velocity_38/1  "<OBJ_S_Velocity_38>"
  Bus Selector:RadarSensor:3_OBJ_S_Velocity_BS/39 -> RadarSensor:3.OBJ_S_Velocity_39/1  "<OBJ_S_Velocity_39>"
  Bus Selector:RadarSensor:3_OBJ_S_Velocity_BS/40 -> RadarSensor:3.OBJ_S_Velocity_40/1  "<OBJ_S_Velocity_40>"
  Bus Selector:RadarSensor:3_OBJ_S_Velocity_BS/41 -> RadarSensor:3.OBJ_S_Velocity_41/1  "<OBJ_S_Velocity_41>"
  Bus Selector:RadarSensor:3_OBJ_S_Velocity_BS/42 -> RadarSensor:3.OBJ_S_Velocity_42/1  "<OBJ_S_Velocity_42>"
  Bus Selector:RadarSensor:3_OBJ_S_Velocity_BS/43 -> RadarSensor:3.OBJ_S_Velocity_43/1  "<OBJ_S_Velocity_43>"
  Bus Selector:RadarSensor:3_OBJ_S_Velocity_BS/44 -> RadarSensor:3.OBJ_S_Velocity_44/1  "<OBJ_S_Velocity_44>"
  Bus Selector:RadarSensor:3_OBJ_S_Velocity_BS/45 -> RadarSensor:3.OBJ_S_Velocity_45/1  "<OBJ_S_Velocity_45>"
  Bus Selector:RadarSensor:3_OBJ_S_Velocity_BS/46 -> RadarSensor:3.OBJ_S_Velocity_46/1  "<OBJ_S_Velocity_46>"
  Bus Selector:RadarSensor:3_OBJ_S_Velocity_BS/47 -> RadarSensor:3.OBJ_S_Velocity_47/1  "<OBJ_S_Velocity_47>"
  Bus Selector:RadarSensor:3_OBJ_S_Velocity_BS/48 -> RadarSensor:3.OBJ_S_Velocity_48/1  "<OBJ_S_Velocity_48>"
  Bus Selector:RadarSensor:3_OBJ_S_Velocity_BS/49 -> RadarSensor:3.OBJ_S_Velocity_49/1  "<OBJ_S_Velocity_49>"
  Bus Selector:RadarSensor:3_OBJ_S_Velocity_BS/50 -> RadarSensor:3.OBJ_S_Velocity_50/1  "<OBJ_S_Velocity_50>"
  Bus Selector:RadarSensor:3_OBJ_S_Velocity_BS/51 -> RadarSensor:3.OBJ_S_Velocity_51/1  "<OBJ_S_Velocity_51>"
  Bus Selector:RadarSensor:3_OBJ_S_Velocity_BS/52 -> RadarSensor:3.OBJ_S_Velocity_52/1  "<OBJ_S_Velocity_52>"
  Bus Selector:RadarSensor:3_OBJ_S_Velocity_BS/53 -> RadarSensor:3.OBJ_S_Velocity_53/1  "<OBJ_S_Velocity_53>"
  Bus Selector:RadarSensor:3_OBJ_S_Velocity_BS/54 -> RadarSensor:3.OBJ_S_Velocity_54/1  "<OBJ_S_Velocity_54>"
  Bus Selector:RadarSensor:3_OBJ_S_Velocity_BS/55 -> RadarSensor:3.OBJ_S_Velocity_55/1  "<OBJ_S_Velocity_55>"
  Bus Selector:RadarSensor:3_OBJ_S_Velocity_BS/56 -> RadarSensor:3.OBJ_S_Velocity_56/1  "<OBJ_S_Velocity_56>"
  Bus Selector:RadarSensor:3_OBJ_S_Velocity_BS/57 -> RadarSensor:3.OBJ_S_Velocity_57/1  "<OBJ_S_Velocity_57>"
  Bus Selector:RadarSensor:3_OBJ_S_Velocity_BS/58 -> RadarSensor:3.OBJ_S_Velocity_58/1  "<OBJ_S_Velocity_58>"
  Bus Selector:RadarSensor:3_OBJ_S_Velocity_BS/59 -> RadarSensor:3.OBJ_S_Velocity_59/1  "<OBJ_S_Velocity_59>"
  Bus Selector:RadarSensor:3_OBJ_S_Velocity_BS/60 -> RadarSensor:3.OBJ_S_Velocity_60/1  "<OBJ_S_Velocity_60>"
  Bus Selector:RadarSensor:3_OBJ_S_Velocity_BS/61 -> RadarSensor:3.OBJ_S_Velocity_61/1  "<OBJ_S_Velocity_61>"
  Bus Selector:RadarSensor:3_OBJ_S_Velocity_BS/62 -> RadarSensor:3.OBJ_S_Velocity_62/1  "<OBJ_S_Velocity_62>"
  Bus Selector:RadarSensor:3_OBJ_S_Velocity_BS/63 -> RadarSensor:3.OBJ_S_Velocity_63/1  "<OBJ_S_Velocity_63>"
  Bus Selector:RadarSensor:3_OBJ_S_Velocity_BS/64 -> RadarSensor:3.OBJ_S_Velocity_64/1  "<OBJ_S_Velocity_64>"
  Bus Selector:RadarSensor:3_OBJ_S_Range_BS/1 -> RadarSensor:3.OBJ_S_Range_1/1  "<OBJ_S_Range_1>"
  Bus Selector:RadarSensor:3_OBJ_S_Range_BS/2 -> RadarSensor:3.OBJ_S_Range_2/1  "<OBJ_S_Range_2>"
  Bus Selector:RadarSensor:3_OBJ_S_Range_BS/3 -> RadarSensor:3.OBJ_S_Range_3/1  "<OBJ_S_Range_3>"
  Bus Selector:RadarSensor:3_OBJ_S_Range_BS/4 -> RadarSensor:3.OBJ_S_Range_4/1  "<OBJ_S_Range_4>"
  Bus Selector:RadarSensor:3_OBJ_S_Range_BS/5 -> RadarSensor:3.OBJ_S_Range_5/1  "<OBJ_S_Range_5>"
  Bus Selector:RadarSensor:3_OBJ_S_Range_BS/6 -> RadarSensor:3.OBJ_S_Range_6/1  "<OBJ_S_Range_6>"
  Bus Selector:RadarSensor:3_OBJ_S_Range_BS/7 -> RadarSensor:3.OBJ_S_Range_7/1  "<OBJ_S_Range_7>"
  Bus Selector:RadarSensor:3_OBJ_S_Range_BS/8 -> RadarSensor:3.OBJ_S_Range_8/1  "<OBJ_S_Range_8>"
  Bus Selector:RadarSensor:3_OBJ_S_Range_BS/9 -> RadarSensor:3.OBJ_S_Range_9/1  "<OBJ_S_Range_9>"
  Bus Selector:RadarSensor:3_OBJ_S_Range_BS/10 -> RadarSensor:3.OBJ_S_Range_10/1  "<OBJ_S_Range_10>"
  Bus Selector:RadarSensor:3_OBJ_S_Range_BS/11 -> RadarSensor:3.OBJ_S_Range_11/1  "<OBJ_S_Range_11>"
  Bus Selector:RadarSensor:3_OBJ_S_Range_BS/12 -> RadarSensor:3.OBJ_S_Range_12/1  "<OBJ_S_Range_12>"
  Bus Selector:RadarSensor:3_OBJ_S_Range_BS/13 -> RadarSensor:3.OBJ_S_Range_13/1  "<OBJ_S_Range_13>"
  Bus Selector:RadarSensor:3_OBJ_S_Range_BS/14 -> RadarSensor:3.OBJ_S_Range_14/1  "<OBJ_S_Range_14>"
  Bus Selector:RadarSensor:3_OBJ_S_Range_BS/15 -> RadarSensor:3.OBJ_S_Range_15/1  "<OBJ_S_Range_15>"
  Bus Selector:RadarSensor:3_OBJ_S_Range_BS/16 -> RadarSensor:3.OBJ_S_Range_16/1  "<OBJ_S_Range_16>"
  Bus Selector:RadarSensor:3_OBJ_S_Range_BS/17 -> RadarSensor:3.OBJ_S_Range_17/1  "<OBJ_S_Range_17>"
  Bus Selector:RadarSensor:3_OBJ_S_Range_BS/18 -> RadarSensor:3.OBJ_S_Range_18/1  "<OBJ_S_Range_18>"
  Bus Selector:RadarSensor:3_OBJ_S_Range_BS/19 -> RadarSensor:3.OBJ_S_Range_19/1  "<OBJ_S_Range_19>"
  Bus Selector:RadarSensor:3_OBJ_S_Range_BS/20 -> RadarSensor:3.OBJ_S_Range_20/1  "<OBJ_S_Range_20>"
  Bus Selector:RadarSensor:3_OBJ_S_Range_BS/21 -> RadarSensor:3.OBJ_S_Range_21/1  "<OBJ_S_Range_21>"
  Bus Selector:RadarSensor:3_OBJ_S_Range_BS/22 -> RadarSensor:3.OBJ_S_Range_22/1  "<OBJ_S_Range_22>"
  Bus Selector:RadarSensor:3_OBJ_S_Range_BS/23 -> RadarSensor:3.OBJ_S_Range_23/1  "<OBJ_S_Range_23>"
  Bus Selector:RadarSensor:3_OBJ_S_Range_BS/24 -> RadarSensor:3.OBJ_S_Range_24/1  "<OBJ_S_Range_24>"
  Bus Selector:RadarSensor:3_OBJ_S_Range_BS/25 -> RadarSensor:3.OBJ_S_Range_25/1  "<OBJ_S_Range_25>"
  Bus Selector:RadarSensor:3_OBJ_S_Range_BS/26 -> RadarSensor:3.OBJ_S_Range_26/1  "<OBJ_S_Range_26>"
  Bus Selector:RadarSensor:3_OBJ_S_Range_BS/27 -> RadarSensor:3.OBJ_S_Range_27/1  "<OBJ_S_Range_27>"
  Bus Selector:RadarSensor:3_OBJ_S_Range_BS/28 -> RadarSensor:3.OBJ_S_Range_28/1  "<OBJ_S_Range_28>"
  Bus Selector:RadarSensor:3_OBJ_S_Range_BS/29 -> RadarSensor:3.OBJ_S_Range_29/1  "<OBJ_S_Range_29>"
  Bus Selector:RadarSensor:3_OBJ_S_Range_BS/30 -> RadarSensor:3.OBJ_S_Range_30/1  "<OBJ_S_Range_30>"
  Bus Selector:RadarSensor:3_OBJ_S_Range_BS/31 -> RadarSensor:3.OBJ_S_Range_31/1  "<OBJ_S_Range_31>"
  Bus Selector:RadarSensor:3_OBJ_S_Range_BS/32 -> RadarSensor:3.OBJ_S_Range_32/1  "<OBJ_S_Range_32>"
  Bus Selector:RadarSensor:3_OBJ_S_Range_BS/33 -> RadarSensor:3.OBJ_S_Range_33/1  "<OBJ_S_Range_33>"
  Bus Selector:RadarSensor:3_OBJ_S_Range_BS/34 -> RadarSensor:3.OBJ_S_Range_34/1  "<OBJ_S_Range_34>"
  Bus Selector:RadarSensor:3_OBJ_S_Range_BS/35 -> RadarSensor:3.OBJ_S_Range_35/1  "<OBJ_S_Range_35>"
  Bus Selector:RadarSensor:3_OBJ_S_Range_BS/36 -> RadarSensor:3.OBJ_S_Range_36/1  "<OBJ_S_Range_36>"
  Bus Selector:RadarSensor:3_OBJ_S_Range_BS/37 -> RadarSensor:3.OBJ_S_Range_37/1  "<OBJ_S_Range_37>"
  Bus Selector:RadarSensor:3_OBJ_S_Range_BS/38 -> RadarSensor:3.OBJ_S_Range_38/1  "<OBJ_S_Range_38>"
  Bus Selector:RadarSensor:3_OBJ_S_Range_BS/39 -> RadarSensor:3.OBJ_S_Range_39/1  "<OBJ_S_Range_39>"
  Bus Selector:RadarSensor:3_OBJ_S_Range_BS/40 -> RadarSensor:3.OBJ_S_Range_40/1  "<OBJ_S_Range_40>"
  Bus Selector:RadarSensor:3_OBJ_S_Range_BS/41 -> RadarSensor:3.OBJ_S_Range_41/1  "<OBJ_S_Range_41>"
  Bus Selector:RadarSensor:3_OBJ_S_Range_BS/42 -> RadarSensor:3.OBJ_S_Range_42/1  "<OBJ_S_Range_42>"
  Bus Selector:RadarSensor:3_OBJ_S_Range_BS/43 -> RadarSensor:3.OBJ_S_Range_43/1  "<OBJ_S_Range_43>"
  Bus Selector:RadarSensor:3_OBJ_S_Range_BS/44 -> RadarSensor:3.OBJ_S_Range_44/1  "<OBJ_S_Range_44>"
  Bus Selector:RadarSensor:3_OBJ_S_Range_BS/45 -> RadarSensor:3.OBJ_S_Range_45/1  "<OBJ_S_Range_45>"
  Bus Selector:RadarSensor:3_OBJ_S_Range_BS/46 -> RadarSensor:3.OBJ_S_Range_46/1  "<OBJ_S_Range_46>"
  Bus Selector:RadarSensor:3_OBJ_S_Range_BS/47 -> RadarSensor:3.OBJ_S_Range_47/1  "<OBJ_S_Range_47>"
  Bus Selector:RadarSensor:3_OBJ_S_Range_BS/48 -> RadarSensor:3.OBJ_S_Range_48/1  "<OBJ_S_Range_48>"
  Bus Selector:RadarSensor:3_OBJ_S_Range_BS/49 -> RadarSensor:3.OBJ_S_Range_49/1  "<OBJ_S_Range_49>"
  Bus Selector:RadarSensor:3_OBJ_S_Range_BS/50 -> RadarSensor:3.OBJ_S_Range_50/1  "<OBJ_S_Range_50>"
  Bus Selector:RadarSensor:3_OBJ_S_Range_BS/51 -> RadarSensor:3.OBJ_S_Range_51/1  "<OBJ_S_Range_51>"
  Bus Selector:RadarSensor:3_OBJ_S_Range_BS/52 -> RadarSensor:3.OBJ_S_Range_52/1  "<OBJ_S_Range_52>"
  Bus Selector:RadarSensor:3_OBJ_S_Range_BS/53 -> RadarSensor:3.OBJ_S_Range_53/1  "<OBJ_S_Range_53>"
  Bus Selector:RadarSensor:3_OBJ_S_Range_BS/54 -> RadarSensor:3.OBJ_S_Range_54/1  "<OBJ_S_Range_54>"
  Bus Selector:RadarSensor:3_OBJ_S_Range_BS/55 -> RadarSensor:3.OBJ_S_Range_55/1  "<OBJ_S_Range_55>"
  Bus Selector:RadarSensor:3_OBJ_S_Range_BS/56 -> RadarSensor:3.OBJ_S_Range_56/1  "<OBJ_S_Range_56>"
  Bus Selector:RadarSensor:3_OBJ_S_Range_BS/57 -> RadarSensor:3.OBJ_S_Range_57/1  "<OBJ_S_Range_57>"
  Bus Selector:RadarSensor:3_OBJ_S_Range_BS/58 -> RadarSensor:3.OBJ_S_Range_58/1  "<OBJ_S_Range_58>"
  Bus Selector:RadarSensor:3_OBJ_S_Range_BS/59 -> RadarSensor:3.OBJ_S_Range_59/1  "<OBJ_S_Range_59>"
  Bus Selector:RadarSensor:3_OBJ_S_Range_BS/60 -> RadarSensor:3.OBJ_S_Range_60/1  "<OBJ_S_Range_60>"
  Bus Selector:RadarSensor:3_OBJ_S_Range_BS/61 -> RadarSensor:3.OBJ_S_Range_61/1  "<OBJ_S_Range_61>"
  Bus Selector:RadarSensor:3_OBJ_S_Range_BS/62 -> RadarSensor:3.OBJ_S_Range_62/1  "<OBJ_S_Range_62>"
  Bus Selector:RadarSensor:3_OBJ_S_Range_BS/63 -> RadarSensor:3.OBJ_S_Range_63/1  "<OBJ_S_Range_63>"
  Bus Selector:RadarSensor:3_OBJ_S_Range_BS/64 -> RadarSensor:3.OBJ_S_Range_64/1  "<OBJ_S_Range_64>"
  Bus Selector:RadarSensor:3_OBJ_RCS_BS/1 -> RadarSensor:3.OBJ_RCS_1/1  "<OBJ_RCS_1>"
  Bus Selector:RadarSensor:3_OBJ_RCS_BS/2 -> RadarSensor:3.OBJ_RCS_2/1  "<OBJ_RCS_2>"
  Bus Selector:RadarSensor:3_OBJ_RCS_BS/3 -> RadarSensor:3.OBJ_RCS_3/1  "<OBJ_RCS_3>"
  Bus Selector:RadarSensor:3_OBJ_RCS_BS/4 -> RadarSensor:3.OBJ_RCS_4/1  "<OBJ_RCS_4>"
  Bus Selector:RadarSensor:3_OBJ_RCS_BS/5 -> RadarSensor:3.OBJ_RCS_5/1  "<OBJ_RCS_5>"
  Bus Selector:RadarSensor:3_OBJ_RCS_BS/6 -> RadarSensor:3.OBJ_RCS_6/1  "<OBJ_RCS_6>"
  Bus Selector:RadarSensor:3_OBJ_RCS_BS/7 -> RadarSensor:3.OBJ_RCS_7/1  "<OBJ_RCS_7>"
  Bus Selector:RadarSensor:3_OBJ_RCS_BS/8 -> RadarSensor:3.OBJ_RCS_8/1  "<OBJ_RCS_8>"
  Bus Selector:RadarSensor:3_OBJ_RCS_BS/9 -> RadarSensor:3.OBJ_RCS_9/1  "<OBJ_RCS_9>"
  Bus Selector:RadarSensor:3_OBJ_RCS_BS/10 -> RadarSensor:3.OBJ_RCS_10/1  "<OBJ_RCS_10>"
  Bus Selector:RadarSensor:3_OBJ_RCS_BS/11 -> RadarSensor:3.OBJ_RCS_11/1  "<OBJ_RCS_11>"
  Bus Selector:RadarSensor:3_OBJ_RCS_BS/12 -> RadarSensor:3.OBJ_RCS_12/1  "<OBJ_RCS_12>"
  Bus Selector:RadarSensor:3_OBJ_RCS_BS/13 -> RadarSensor:3.OBJ_RCS_13/1  "<OBJ_RCS_13>"
  Bus Selector:RadarSensor:3_OBJ_RCS_BS/14 -> RadarSensor:3.OBJ_RCS_14/1  "<OBJ_RCS_14>"
  Bus Selector:RadarSensor:3_OBJ_RCS_BS/15 -> RadarSensor:3.OBJ_RCS_15/1  "<OBJ_RCS_15>"
  Bus Selector:RadarSensor:3_OBJ_RCS_BS/16 -> RadarSensor:3.OBJ_RCS_16/1  "<OBJ_RCS_16>"
  Bus Selector:RadarSensor:3_OBJ_RCS_BS/17 -> RadarSensor:3.OBJ_RCS_17/1  "<OBJ_RCS_17>"
  Bus Selector:RadarSensor:3_OBJ_RCS_BS/18 -> RadarSensor:3.OBJ_RCS_18/1  "<OBJ_RCS_18>"
  Bus Selector:RadarSensor:3_OBJ_RCS_BS/19 -> RadarSensor:3.OBJ_RCS_19/1  "<OBJ_RCS_19>"
  Bus Selector:RadarSensor:3_OBJ_RCS_BS/20 -> RadarSensor:3.OBJ_RCS_20/1  "<OBJ_RCS_20>"
  Bus Selector:RadarSensor:3_OBJ_RCS_BS/21 -> RadarSensor:3.OBJ_RCS_21/1  "<OBJ_RCS_21>"
  Bus Selector:RadarSensor:3_OBJ_RCS_BS/22 -> RadarSensor:3.OBJ_RCS_22/1  "<OBJ_RCS_22>"
  Bus Selector:RadarSensor:3_OBJ_RCS_BS/23 -> RadarSensor:3.OBJ_RCS_23/1  "<OBJ_RCS_23>"
  Bus Selector:RadarSensor:3_OBJ_RCS_BS/24 -> RadarSensor:3.OBJ_RCS_24/1  "<OBJ_RCS_24>"
  Bus Selector:RadarSensor:3_OBJ_RCS_BS/25 -> RadarSensor:3.OBJ_RCS_25/1  "<OBJ_RCS_25>"
  Bus Selector:RadarSensor:3_OBJ_RCS_BS/26 -> RadarSensor:3.OBJ_RCS_26/1  "<OBJ_RCS_26>"
  Bus Selector:RadarSensor:3_OBJ_RCS_BS/27 -> RadarSensor:3.OBJ_RCS_27/1  "<OBJ_RCS_27>"
  Bus Selector:RadarSensor:3_OBJ_RCS_BS/28 -> RadarSensor:3.OBJ_RCS_28/1  "<OBJ_RCS_28>"
  Bus Selector:RadarSensor:3_OBJ_RCS_BS/29 -> RadarSensor:3.OBJ_RCS_29/1  "<OBJ_RCS_29>"
  Bus Selector:RadarSensor:3_OBJ_RCS_BS/30 -> RadarSensor:3.OBJ_RCS_30/1  "<OBJ_RCS_30>"
  Bus Selector:RadarSensor:3_OBJ_RCS_BS/31 -> RadarSensor:3.OBJ_RCS_31/1  "<OBJ_RCS_31>"
  Bus Selector:RadarSensor:3_OBJ_RCS_BS/32 -> RadarSensor:3.OBJ_RCS_32/1  "<OBJ_RCS_32>"
  Bus Selector:RadarSensor:3_OBJ_RCS_BS/33 -> RadarSensor:3.OBJ_RCS_33/1  "<OBJ_RCS_33>"
  Bus Selector:RadarSensor:3_OBJ_RCS_BS/34 -> RadarSensor:3.OBJ_RCS_34/1  "<OBJ_RCS_34>"
  Bus Selector:RadarSensor:3_OBJ_RCS_BS/35 -> RadarSensor:3.OBJ_RCS_35/1  "<OBJ_RCS_35>"
  Bus Selector:RadarSensor:3_OBJ_RCS_BS/36 -> RadarSensor:3.OBJ_RCS_36/1  "<OBJ_RCS_36>"
  Bus Selector:RadarSensor:3_OBJ_RCS_BS/37 -> RadarSensor:3.OBJ_RCS_37/1  "<OBJ_RCS_37>"
  Bus Selector:RadarSensor:3_OBJ_RCS_BS/38 -> RadarSensor:3.OBJ_RCS_38/1  "<OBJ_RCS_38>"
  Bus Selector:RadarSensor:3_OBJ_RCS_BS/39 -> RadarSensor:3.OBJ_RCS_39/1  "<OBJ_RCS_39>"
  Bus Selector:RadarSensor:3_OBJ_RCS_BS/40 -> RadarSensor:3.OBJ_RCS_40/1  "<OBJ_RCS_40>"
  Bus Selector:RadarSensor:3_OBJ_RCS_BS/41 -> RadarSensor:3.OBJ_RCS_41/1  "<OBJ_RCS_41>"
  Bus Selector:RadarSensor:3_OBJ_RCS_BS/42 -> RadarSensor:3.OBJ_RCS_42/1  "<OBJ_RCS_42>"
  Bus Selector:RadarSensor:3_OBJ_RCS_BS/43 -> RadarSensor:3.OBJ_RCS_43/1  "<OBJ_RCS_43>"
  Bus Selector:RadarSensor:3_OBJ_RCS_BS/44 -> RadarSensor:3.OBJ_RCS_44/1  "<OBJ_RCS_44>"
  Bus Selector:RadarSensor:3_OBJ_RCS_BS/45 -> RadarSensor:3.OBJ_RCS_45/1  "<OBJ_RCS_45>"
  Bus Selector:RadarSensor:3_OBJ_RCS_BS/46 -> RadarSensor:3.OBJ_RCS_46/1  "<OBJ_RCS_46>"
  Bus Selector:RadarSensor:3_OBJ_RCS_BS/47 -> RadarSensor:3.OBJ_RCS_47/1  "<OBJ_RCS_47>"
  Bus Selector:RadarSensor:3_OBJ_RCS_BS/48 -> RadarSensor:3.OBJ_RCS_48/1  "<OBJ_RCS_48>"
  Bus Selector:RadarSensor:3_OBJ_RCS_BS/49 -> RadarSensor:3.OBJ_RCS_49/1  "<OBJ_RCS_49>"
  Bus Selector:RadarSensor:3_OBJ_RCS_BS/50 -> RadarSensor:3.OBJ_RCS_50/1  "<OBJ_RCS_50>"
  Bus Selector:RadarSensor:3_OBJ_RCS_BS/51 -> RadarSensor:3.OBJ_RCS_51/1  "<OBJ_RCS_51>"
  Bus Selector:RadarSensor:3_OBJ_RCS_BS/52 -> RadarSensor:3.OBJ_RCS_52/1  "<OBJ_RCS_52>"
  Bus Selector:RadarSensor:3_OBJ_RCS_BS/53 -> RadarSensor:3.OBJ_RCS_53/1  "<OBJ_RCS_53>"
  Bus Selector:RadarSensor:3_OBJ_RCS_BS/54 -> RadarSensor:3.OBJ_RCS_54/1  "<OBJ_RCS_54>"
  Bus Selector:RadarSensor:3_OBJ_RCS_BS/55 -> RadarSensor:3.OBJ_RCS_55/1  "<OBJ_RCS_55>"
  Bus Selector:RadarSensor:3_OBJ_RCS_BS/56 -> RadarSensor:3.OBJ_RCS_56/1  "<OBJ_RCS_56>"
  Bus Selector:RadarSensor:3_OBJ_RCS_BS/57 -> RadarSensor:3.OBJ_RCS_57/1  "<OBJ_RCS_57>"
  Bus Selector:RadarSensor:3_OBJ_RCS_BS/58 -> RadarSensor:3.OBJ_RCS_58/1  "<OBJ_RCS_58>"
  Bus Selector:RadarSensor:3_OBJ_RCS_BS/59 -> RadarSensor:3.OBJ_RCS_59/1  "<OBJ_RCS_59>"
  Bus Selector:RadarSensor:3_OBJ_RCS_BS/60 -> RadarSensor:3.OBJ_RCS_60/1  "<OBJ_RCS_60>"
  Bus Selector:RadarSensor:3_OBJ_RCS_BS/61 -> RadarSensor:3.OBJ_RCS_61/1  "<OBJ_RCS_61>"
  Bus Selector:RadarSensor:3_OBJ_RCS_BS/62 -> RadarSensor:3.OBJ_RCS_62/1  "<OBJ_RCS_62>"
  Bus Selector:RadarSensor:3_OBJ_RCS_BS/63 -> RadarSensor:3.OBJ_RCS_63/1  "<OBJ_RCS_63>"
  Bus Selector:RadarSensor:3_OBJ_RCS_BS/64 -> RadarSensor:3.OBJ_RCS_64/1  "<OBJ_RCS_64>"
  Bus Selector:RadarSensor:3/1 -> RadarSensor:3.time/1  "<time>"
  Bus Selector:RadarSensor:3/2 -> RadarSensor:3.width/1  "<width>"
  Bus Selector:RadarSensor:3/3 -> RadarSensor:3.OBJ_ID/1, Bus Selector:RadarSensor:3_OBJ_ID_BS/1  "<OBJ_ID>"
  Bus Selector:RadarSensor:3/4 -> RadarSensor:3.OBJ_Class/1, Bus Selector:RadarSensor:3_OBJ_Class_BS/1  "<OBJ_Class>"
  Bus Selector:RadarSensor:3/5 -> RadarSensor:3.OBJ_S_Azimuth/1, Bus Selector:RadarSensor:3_OBJ_S_Azimuth_BS/1  "<OBJ_S_Azimuth>"
  Bus Selector:RadarSensor:3/6 -> RadarSensor:3.OBJ_S_Elevation/1, Bus Selector:RadarSensor:3_OBJ_S_Elevation_BS/1  "<OBJ_S_Elevation>"
  Bus Selector:RadarSensor:3/7 -> RadarSensor:3.OBJ_S_Velocity/1, Bus Selector:RadarSensor:3_OBJ_S_Velocity_BS/1  "<OBJ_S_Velocity>"
  Bus Selector:RadarSensor:3/8 -> RadarSensor:3.OBJ_S_Range/1, Bus Selector:RadarSensor:3_OBJ_S_Range_BS/1  "<OBJ_S_Range>"
  Bus Selector:RadarSensor:3/9 -> RadarSensor:3.OBJ_RCS/1, Bus Selector:RadarSensor:3_OBJ_RCS_BS/1  "<OBJ_RCS>"
  Bus Selector:RadarSensor:4_OBJ_ID_BS/1 -> RadarSensor:4.OBJ_ID_1/1  "<OBJ_ID_1>"
  Bus Selector:RadarSensor:4_OBJ_ID_BS/2 -> RadarSensor:4.OBJ_ID_2/1  "<OBJ_ID_2>"
  Bus Selector:RadarSensor:4_OBJ_ID_BS/3 -> RadarSensor:4.OBJ_ID_3/1  "<OBJ_ID_3>"
  Bus Selector:RadarSensor:4_OBJ_ID_BS/4 -> RadarSensor:4.OBJ_ID_4/1  "<OBJ_ID_4>"
  Bus Selector:RadarSensor:4_OBJ_ID_BS/5 -> RadarSensor:4.OBJ_ID_5/1  "<OBJ_ID_5>"
  Bus Selector:RadarSensor:4_OBJ_ID_BS/6 -> RadarSensor:4.OBJ_ID_6/1  "<OBJ_ID_6>"
  Bus Selector:RadarSensor:4_OBJ_ID_BS/7 -> RadarSensor:4.OBJ_ID_7/1  "<OBJ_ID_7>"
  Bus Selector:RadarSensor:4_OBJ_ID_BS/8 -> RadarSensor:4.OBJ_ID_8/1  "<OBJ_ID_8>"
  Bus Selector:RadarSensor:4_OBJ_ID_BS/9 -> RadarSensor:4.OBJ_ID_9/1  "<OBJ_ID_9>"
  Bus Selector:RadarSensor:4_OBJ_ID_BS/10 -> RadarSensor:4.OBJ_ID_10/1  "<OBJ_ID_10>"
  Bus Selector:RadarSensor:4_OBJ_ID_BS/11 -> RadarSensor:4.OBJ_ID_11/1  "<OBJ_ID_11>"
  Bus Selector:RadarSensor:4_OBJ_ID_BS/12 -> RadarSensor:4.OBJ_ID_12/1  "<OBJ_ID_12>"
  Bus Selector:RadarSensor:4_OBJ_ID_BS/13 -> RadarSensor:4.OBJ_ID_13/1  "<OBJ_ID_13>"
  Bus Selector:RadarSensor:4_OBJ_ID_BS/14 -> RadarSensor:4.OBJ_ID_14/1  "<OBJ_ID_14>"
  Bus Selector:RadarSensor:4_OBJ_ID_BS/15 -> RadarSensor:4.OBJ_ID_15/1  "<OBJ_ID_15>"
  Bus Selector:RadarSensor:4_OBJ_ID_BS/16 -> RadarSensor:4.OBJ_ID_16/1  "<OBJ_ID_16>"
  Bus Selector:RadarSensor:4_OBJ_ID_BS/17 -> RadarSensor:4.OBJ_ID_17/1  "<OBJ_ID_17>"
  Bus Selector:RadarSensor:4_OBJ_ID_BS/18 -> RadarSensor:4.OBJ_ID_18/1  "<OBJ_ID_18>"
  Bus Selector:RadarSensor:4_OBJ_ID_BS/19 -> RadarSensor:4.OBJ_ID_19/1  "<OBJ_ID_19>"
  Bus Selector:RadarSensor:4_OBJ_ID_BS/20 -> RadarSensor:4.OBJ_ID_20/1  "<OBJ_ID_20>"
  Bus Selector:RadarSensor:4_OBJ_ID_BS/21 -> RadarSensor:4.OBJ_ID_21/1  "<OBJ_ID_21>"
  Bus Selector:RadarSensor:4_OBJ_ID_BS/22 -> RadarSensor:4.OBJ_ID_22/1  "<OBJ_ID_22>"
  Bus Selector:RadarSensor:4_OBJ_ID_BS/23 -> RadarSensor:4.OBJ_ID_23/1  "<OBJ_ID_23>"
  Bus Selector:RadarSensor:4_OBJ_ID_BS/24 -> RadarSensor:4.OBJ_ID_24/1  "<OBJ_ID_24>"
  Bus Selector:RadarSensor:4_OBJ_ID_BS/25 -> RadarSensor:4.OBJ_ID_25/1  "<OBJ_ID_25>"
  Bus Selector:RadarSensor:4_OBJ_ID_BS/26 -> RadarSensor:4.OBJ_ID_26/1  "<OBJ_ID_26>"
  Bus Selector:RadarSensor:4_OBJ_ID_BS/27 -> RadarSensor:4.OBJ_ID_27/1  "<OBJ_ID_27>"
  Bus Selector:RadarSensor:4_OBJ_ID_BS/28 -> RadarSensor:4.OBJ_ID_28/1  "<OBJ_ID_28>"
  Bus Selector:RadarSensor:4_OBJ_ID_BS/29 -> RadarSensor:4.OBJ_ID_29/1  "<OBJ_ID_29>"
  Bus Selector:RadarSensor:4_OBJ_ID_BS/30 -> RadarSensor:4.OBJ_ID_30/1  "<OBJ_ID_30>"
  Bus Selector:RadarSensor:4_OBJ_ID_BS/31 -> RadarSensor:4.OBJ_ID_31/1  "<OBJ_ID_31>"
  Bus Selector:RadarSensor:4_OBJ_ID_BS/32 -> RadarSensor:4.OBJ_ID_32/1  "<OBJ_ID_32>"
  Bus Selector:RadarSensor:4_OBJ_ID_BS/33 -> RadarSensor:4.OBJ_ID_33/1  "<OBJ_ID_33>"
  Bus Selector:RadarSensor:4_OBJ_ID_BS/34 -> RadarSensor:4.OBJ_ID_34/1  "<OBJ_ID_34>"
  Bus Selector:RadarSensor:4_OBJ_ID_BS/35 -> RadarSensor:4.OBJ_ID_35/1  "<OBJ_ID_35>"
  Bus Selector:RadarSensor:4_OBJ_ID_BS/36 -> RadarSensor:4.OBJ_ID_36/1  "<OBJ_ID_36>"
  Bus Selector:RadarSensor:4_OBJ_ID_BS/37 -> RadarSensor:4.OBJ_ID_37/1  "<OBJ_ID_37>"
  Bus Selector:RadarSensor:4_OBJ_ID_BS/38 -> RadarSensor:4.OBJ_ID_38/1  "<OBJ_ID_38>"
  Bus Selector:RadarSensor:4_OBJ_ID_BS/39 -> RadarSensor:4.OBJ_ID_39/1  "<OBJ_ID_39>"
  Bus Selector:RadarSensor:4_OBJ_ID_BS/40 -> RadarSensor:4.OBJ_ID_40/1  "<OBJ_ID_40>"
  Bus Selector:RadarSensor:4_OBJ_ID_BS/41 -> RadarSensor:4.OBJ_ID_41/1  "<OBJ_ID_41>"
  Bus Selector:RadarSensor:4_OBJ_ID_BS/42 -> RadarSensor:4.OBJ_ID_42/1  "<OBJ_ID_42>"
  Bus Selector:RadarSensor:4_OBJ_ID_BS/43 -> RadarSensor:4.OBJ_ID_43/1  "<OBJ_ID_43>"
  Bus Selector:RadarSensor:4_OBJ_ID_BS/44 -> RadarSensor:4.OBJ_ID_44/1  "<OBJ_ID_44>"
  Bus Selector:RadarSensor:4_OBJ_ID_BS/45 -> RadarSensor:4.OBJ_ID_45/1  "<OBJ_ID_45>"
  Bus Selector:RadarSensor:4_OBJ_ID_BS/46 -> RadarSensor:4.OBJ_ID_46/1  "<OBJ_ID_46>"
  Bus Selector:RadarSensor:4_OBJ_ID_BS/47 -> RadarSensor:4.OBJ_ID_47/1  "<OBJ_ID_47>"
  Bus Selector:RadarSensor:4_OBJ_ID_BS/48 -> RadarSensor:4.OBJ_ID_48/1  "<OBJ_ID_48>"
  Bus Selector:RadarSensor:4_OBJ_ID_BS/49 -> RadarSensor:4.OBJ_ID_49/1  "<OBJ_ID_49>"
  Bus Selector:RadarSensor:4_OBJ_ID_BS/50 -> RadarSensor:4.OBJ_ID_50/1  "<OBJ_ID_50>"
  Bus Selector:RadarSensor:4_OBJ_ID_BS/51 -> RadarSensor:4.OBJ_ID_51/1  "<OBJ_ID_51>"
  Bus Selector:RadarSensor:4_OBJ_ID_BS/52 -> RadarSensor:4.OBJ_ID_52/1  "<OBJ_ID_52>"
  Bus Selector:RadarSensor:4_OBJ_ID_BS/53 -> RadarSensor:4.OBJ_ID_53/1  "<OBJ_ID_53>"
  Bus Selector:RadarSensor:4_OBJ_ID_BS/54 -> RadarSensor:4.OBJ_ID_54/1  "<OBJ_ID_54>"
  Bus Selector:RadarSensor:4_OBJ_ID_BS/55 -> RadarSensor:4.OBJ_ID_55/1  "<OBJ_ID_55>"
  Bus Selector:RadarSensor:4_OBJ_ID_BS/56 -> RadarSensor:4.OBJ_ID_56/1  "<OBJ_ID_56>"
  Bus Selector:RadarSensor:4_OBJ_ID_BS/57 -> RadarSensor:4.OBJ_ID_57/1  "<OBJ_ID_57>"
  Bus Selector:RadarSensor:4_OBJ_ID_BS/58 -> RadarSensor:4.OBJ_ID_58/1  "<OBJ_ID_58>"
  Bus Selector:RadarSensor:4_OBJ_ID_BS/59 -> RadarSensor:4.OBJ_ID_59/1  "<OBJ_ID_59>"
  Bus Selector:RadarSensor:4_OBJ_ID_BS/60 -> RadarSensor:4.OBJ_ID_60/1  "<OBJ_ID_60>"
  Bus Selector:RadarSensor:4_OBJ_ID_BS/61 -> RadarSensor:4.OBJ_ID_61/1  "<OBJ_ID_61>"
  Bus Selector:RadarSensor:4_OBJ_ID_BS/62 -> RadarSensor:4.OBJ_ID_62/1  "<OBJ_ID_62>"
  Bus Selector:RadarSensor:4_OBJ_ID_BS/63 -> RadarSensor:4.OBJ_ID_63/1  "<OBJ_ID_63>"
  Bus Selector:RadarSensor:4_OBJ_ID_BS/64 -> RadarSensor:4.OBJ_ID_64/1  "<OBJ_ID_64>"
  Bus Selector:RadarSensor:4_OBJ_Class_BS/1 -> RadarSensor:4.OBJ_Class_1/1  "<OBJ_Class_1>"
  Bus Selector:RadarSensor:4_OBJ_Class_BS/2 -> RadarSensor:4.OBJ_Class_2/1  "<OBJ_Class_2>"
  Bus Selector:RadarSensor:4_OBJ_Class_BS/3 -> RadarSensor:4.OBJ_Class_3/1  "<OBJ_Class_3>"
  Bus Selector:RadarSensor:4_OBJ_Class_BS/4 -> RadarSensor:4.OBJ_Class_4/1  "<OBJ_Class_4>"
  Bus Selector:RadarSensor:4_OBJ_Class_BS/5 -> RadarSensor:4.OBJ_Class_5/1  "<OBJ_Class_5>"
  Bus Selector:RadarSensor:4_OBJ_Class_BS/6 -> RadarSensor:4.OBJ_Class_6/1  "<OBJ_Class_6>"
  Bus Selector:RadarSensor:4_OBJ_Class_BS/7 -> RadarSensor:4.OBJ_Class_7/1  "<OBJ_Class_7>"
  Bus Selector:RadarSensor:4_OBJ_Class_BS/8 -> RadarSensor:4.OBJ_Class_8/1  "<OBJ_Class_8>"
  Bus Selector:RadarSensor:4_OBJ_Class_BS/9 -> RadarSensor:4.OBJ_Class_9/1  "<OBJ_Class_9>"
  Bus Selector:RadarSensor:4_OBJ_Class_BS/10 -> RadarSensor:4.OBJ_Class_10/1  "<OBJ_Class_10>"
  Bus Selector:RadarSensor:4_OBJ_Class_BS/11 -> RadarSensor:4.OBJ_Class_11/1  "<OBJ_Class_11>"
  Bus Selector:RadarSensor:4_OBJ_Class_BS/12 -> RadarSensor:4.OBJ_Class_12/1  "<OBJ_Class_12>"
  Bus Selector:RadarSensor:4_OBJ_Class_BS/13 -> RadarSensor:4.OBJ_Class_13/1  "<OBJ_Class_13>"
  Bus Selector:RadarSensor:4_OBJ_Class_BS/14 -> RadarSensor:4.OBJ_Class_14/1  "<OBJ_Class_14>"
  Bus Selector:RadarSensor:4_OBJ_Class_BS/15 -> RadarSensor:4.OBJ_Class_15/1  "<OBJ_Class_15>"
  Bus Selector:RadarSensor:4_OBJ_Class_BS/16 -> RadarSensor:4.OBJ_Class_16/1  "<OBJ_Class_16>"
  Bus Selector:RadarSensor:4_OBJ_Class_BS/17 -> RadarSensor:4.OBJ_Class_17/1  "<OBJ_Class_17>"
  Bus Selector:RadarSensor:4_OBJ_Class_BS/18 -> RadarSensor:4.OBJ_Class_18/1  "<OBJ_Class_18>"
  Bus Selector:RadarSensor:4_OBJ_Class_BS/19 -> RadarSensor:4.OBJ_Class_19/1  "<OBJ_Class_19>"
  Bus Selector:RadarSensor:4_OBJ_Class_BS/20 -> RadarSensor:4.OBJ_Class_20/1  "<OBJ_Class_20>"
  Bus Selector:RadarSensor:4_OBJ_Class_BS/21 -> RadarSensor:4.OBJ_Class_21/1  "<OBJ_Class_21>"
  Bus Selector:RadarSensor:4_OBJ_Class_BS/22 -> RadarSensor:4.OBJ_Class_22/1  "<OBJ_Class_22>"
  Bus Selector:RadarSensor:4_OBJ_Class_BS/23 -> RadarSensor:4.OBJ_Class_23/1  "<OBJ_Class_23>"
  Bus Selector:RadarSensor:4_OBJ_Class_BS/24 -> RadarSensor:4.OBJ_Class_24/1  "<OBJ_Class_24>"
  Bus Selector:RadarSensor:4_OBJ_Class_BS/25 -> RadarSensor:4.OBJ_Class_25/1  "<OBJ_Class_25>"
  Bus Selector:RadarSensor:4_OBJ_Class_BS/26 -> RadarSensor:4.OBJ_Class_26/1  "<OBJ_Class_26>"
  Bus Selector:RadarSensor:4_OBJ_Class_BS/27 -> RadarSensor:4.OBJ_Class_27/1  "<OBJ_Class_27>"
  Bus Selector:RadarSensor:4_OBJ_Class_BS/28 -> RadarSensor:4.OBJ_Class_28/1  "<OBJ_Class_28>"
  Bus Selector:RadarSensor:4_OBJ_Class_BS/29 -> RadarSensor:4.OBJ_Class_29/1  "<OBJ_Class_29>"
  Bus Selector:RadarSensor:4_OBJ_Class_BS/30 -> RadarSensor:4.OBJ_Class_30/1  "<OBJ_Class_30>"
  Bus Selector:RadarSensor:4_OBJ_Class_BS/31 -> RadarSensor:4.OBJ_Class_31/1  "<OBJ_Class_31>"
  Bus Selector:RadarSensor:4_OBJ_Class_BS/32 -> RadarSensor:4.OBJ_Class_32/1  "<OBJ_Class_32>"
  Bus Selector:RadarSensor:4_OBJ_Class_BS/33 -> RadarSensor:4.OBJ_Class_33/1  "<OBJ_Class_33>"
  Bus Selector:RadarSensor:4_OBJ_Class_BS/34 -> RadarSensor:4.OBJ_Class_34/1  "<OBJ_Class_34>"
  Bus Selector:RadarSensor:4_OBJ_Class_BS/35 -> RadarSensor:4.OBJ_Class_35/1  "<OBJ_Class_35>"
  Bus Selector:RadarSensor:4_OBJ_Class_BS/36 -> RadarSensor:4.OBJ_Class_36/1  "<OBJ_Class_36>"
  Bus Selector:RadarSensor:4_OBJ_Class_BS/37 -> RadarSensor:4.OBJ_Class_37/1  "<OBJ_Class_37>"
  Bus Selector:RadarSensor:4_OBJ_Class_BS/38 -> RadarSensor:4.OBJ_Class_38/1  "<OBJ_Class_38>"
  Bus Selector:RadarSensor:4_OBJ_Class_BS/39 -> RadarSensor:4.OBJ_Class_39/1  "<OBJ_Class_39>"
  Bus Selector:RadarSensor:4_OBJ_Class_BS/40 -> RadarSensor:4.OBJ_Class_40/1  "<OBJ_Class_40>"
  Bus Selector:RadarSensor:4_OBJ_Class_BS/41 -> RadarSensor:4.OBJ_Class_41/1  "<OBJ_Class_41>"
  Bus Selector:RadarSensor:4_OBJ_Class_BS/42 -> RadarSensor:4.OBJ_Class_42/1  "<OBJ_Class_42>"
  Bus Selector:RadarSensor:4_OBJ_Class_BS/43 -> RadarSensor:4.OBJ_Class_43/1  "<OBJ_Class_43>"
  Bus Selector:RadarSensor:4_OBJ_Class_BS/44 -> RadarSensor:4.OBJ_Class_44/1  "<OBJ_Class_44>"
  Bus Selector:RadarSensor:4_OBJ_Class_BS/45 -> RadarSensor:4.OBJ_Class_45/1  "<OBJ_Class_45>"
  Bus Selector:RadarSensor:4_OBJ_Class_BS/46 -> RadarSensor:4.OBJ_Class_46/1  "<OBJ_Class_46>"
  Bus Selector:RadarSensor:4_OBJ_Class_BS/47 -> RadarSensor:4.OBJ_Class_47/1  "<OBJ_Class_47>"
  Bus Selector:RadarSensor:4_OBJ_Class_BS/48 -> RadarSensor:4.OBJ_Class_48/1  "<OBJ_Class_48>"
  Bus Selector:RadarSensor:4_OBJ_Class_BS/49 -> RadarSensor:4.OBJ_Class_49/1  "<OBJ_Class_49>"
  Bus Selector:RadarSensor:4_OBJ_Class_BS/50 -> RadarSensor:4.OBJ_Class_50/1  "<OBJ_Class_50>"
  Bus Selector:RadarSensor:4_OBJ_Class_BS/51 -> RadarSensor:4.OBJ_Class_51/1  "<OBJ_Class_51>"
  Bus Selector:RadarSensor:4_OBJ_Class_BS/52 -> RadarSensor:4.OBJ_Class_52/1  "<OBJ_Class_52>"
  Bus Selector:RadarSensor:4_OBJ_Class_BS/53 -> RadarSensor:4.OBJ_Class_53/1  "<OBJ_Class_53>"
  Bus Selector:RadarSensor:4_OBJ_Class_BS/54 -> RadarSensor:4.OBJ_Class_54/1  "<OBJ_Class_54>"
  Bus Selector:RadarSensor:4_OBJ_Class_BS/55 -> RadarSensor:4.OBJ_Class_55/1  "<OBJ_Class_55>"
  Bus Selector:RadarSensor:4_OBJ_Class_BS/56 -> RadarSensor:4.OBJ_Class_56/1  "<OBJ_Class_56>"
  Bus Selector:RadarSensor:4_OBJ_Class_BS/57 -> RadarSensor:4.OBJ_Class_57/1  "<OBJ_Class_57>"
  Bus Selector:RadarSensor:4_OBJ_Class_BS/58 -> RadarSensor:4.OBJ_Class_58/1  "<OBJ_Class_58>"
  Bus Selector:RadarSensor:4_OBJ_Class_BS/59 -> RadarSensor:4.OBJ_Class_59/1  "<OBJ_Class_59>"
  Bus Selector:RadarSensor:4_OBJ_Class_BS/60 -> RadarSensor:4.OBJ_Class_60/1  "<OBJ_Class_60>"
  Bus Selector:RadarSensor:4_OBJ_Class_BS/61 -> RadarSensor:4.OBJ_Class_61/1  "<OBJ_Class_61>"
  Bus Selector:RadarSensor:4_OBJ_Class_BS/62 -> RadarSensor:4.OBJ_Class_62/1  "<OBJ_Class_62>"
  Bus Selector:RadarSensor:4_OBJ_Class_BS/63 -> RadarSensor:4.OBJ_Class_63/1  "<OBJ_Class_63>"
  Bus Selector:RadarSensor:4_OBJ_Class_BS/64 -> RadarSensor:4.OBJ_Class_64/1  "<OBJ_Class_64>"
  Bus Selector:RadarSensor:4_OBJ_S_Azimuth_BS/1 -> RadarSensor:4.OBJ_S_Azimuth_1/1  "<OBJ_S_Azimuth_1>"
  Bus Selector:RadarSensor:4_OBJ_S_Azimuth_BS/2 -> RadarSensor:4.OBJ_S_Azimuth_2/1  "<OBJ_S_Azimuth_2>"
  Bus Selector:RadarSensor:4_OBJ_S_Azimuth_BS/3 -> RadarSensor:4.OBJ_S_Azimuth_3/1  "<OBJ_S_Azimuth_3>"
  Bus Selector:RadarSensor:4_OBJ_S_Azimuth_BS/4 -> RadarSensor:4.OBJ_S_Azimuth_4/1  "<OBJ_S_Azimuth_4>"
  Bus Selector:RadarSensor:4_OBJ_S_Azimuth_BS/5 -> RadarSensor:4.OBJ_S_Azimuth_5/1  "<OBJ_S_Azimuth_5>"
  Bus Selector:RadarSensor:4_OBJ_S_Azimuth_BS/6 -> RadarSensor:4.OBJ_S_Azimuth_6/1  "<OBJ_S_Azimuth_6>"
  Bus Selector:RadarSensor:4_OBJ_S_Azimuth_BS/7 -> RadarSensor:4.OBJ_S_Azimuth_7/1  "<OBJ_S_Azimuth_7>"
  Bus Selector:RadarSensor:4_OBJ_S_Azimuth_BS/8 -> RadarSensor:4.OBJ_S_Azimuth_8/1  "<OBJ_S_Azimuth_8>"
  Bus Selector:RadarSensor:4_OBJ_S_Azimuth_BS/9 -> RadarSensor:4.OBJ_S_Azimuth_9/1  "<OBJ_S_Azimuth_9>"
  Bus Selector:RadarSensor:4_OBJ_S_Azimuth_BS/10 -> RadarSensor:4.OBJ_S_Azimuth_10/1  "<OBJ_S_Azimuth_10>"
  Bus Selector:RadarSensor:4_OBJ_S_Azimuth_BS/11 -> RadarSensor:4.OBJ_S_Azimuth_11/1  "<OBJ_S_Azimuth_11>"
  Bus Selector:RadarSensor:4_OBJ_S_Azimuth_BS/12 -> RadarSensor:4.OBJ_S_Azimuth_12/1  "<OBJ_S_Azimuth_12>"
  Bus Selector:RadarSensor:4_OBJ_S_Azimuth_BS/13 -> RadarSensor:4.OBJ_S_Azimuth_13/1  "<OBJ_S_Azimuth_13>"
  Bus Selector:RadarSensor:4_OBJ_S_Azimuth_BS/14 -> RadarSensor:4.OBJ_S_Azimuth_14/1  "<OBJ_S_Azimuth_14>"
  Bus Selector:RadarSensor:4_OBJ_S_Azimuth_BS/15 -> RadarSensor:4.OBJ_S_Azimuth_15/1  "<OBJ_S_Azimuth_15>"
  Bus Selector:RadarSensor:4_OBJ_S_Azimuth_BS/16 -> RadarSensor:4.OBJ_S_Azimuth_16/1  "<OBJ_S_Azimuth_16>"
  Bus Selector:RadarSensor:4_OBJ_S_Azimuth_BS/17 -> RadarSensor:4.OBJ_S_Azimuth_17/1  "<OBJ_S_Azimuth_17>"
  Bus Selector:RadarSensor:4_OBJ_S_Azimuth_BS/18 -> RadarSensor:4.OBJ_S_Azimuth_18/1  "<OBJ_S_Azimuth_18>"
  Bus Selector:RadarSensor:4_OBJ_S_Azimuth_BS/19 -> RadarSensor:4.OBJ_S_Azimuth_19/1  "<OBJ_S_Azimuth_19>"
  Bus Selector:RadarSensor:4_OBJ_S_Azimuth_BS/20 -> RadarSensor:4.OBJ_S_Azimuth_20/1  "<OBJ_S_Azimuth_20>"
  Bus Selector:RadarSensor:4_OBJ_S_Azimuth_BS/21 -> RadarSensor:4.OBJ_S_Azimuth_21/1  "<OBJ_S_Azimuth_21>"
  Bus Selector:RadarSensor:4_OBJ_S_Azimuth_BS/22 -> RadarSensor:4.OBJ_S_Azimuth_22/1  "<OBJ_S_Azimuth_22>"
  Bus Selector:RadarSensor:4_OBJ_S_Azimuth_BS/23 -> RadarSensor:4.OBJ_S_Azimuth_23/1  "<OBJ_S_Azimuth_23>"
  Bus Selector:RadarSensor:4_OBJ_S_Azimuth_BS/24 -> RadarSensor:4.OBJ_S_Azimuth_24/1  "<OBJ_S_Azimuth_24>"
  Bus Selector:RadarSensor:4_OBJ_S_Azimuth_BS/25 -> RadarSensor:4.OBJ_S_Azimuth_25/1  "<OBJ_S_Azimuth_25>"
  Bus Selector:RadarSensor:4_OBJ_S_Azimuth_BS/26 -> RadarSensor:4.OBJ_S_Azimuth_26/1  "<OBJ_S_Azimuth_26>"
  Bus Selector:RadarSensor:4_OBJ_S_Azimuth_BS/27 -> RadarSensor:4.OBJ_S_Azimuth_27/1  "<OBJ_S_Azimuth_27>"
  Bus Selector:RadarSensor:4_OBJ_S_Azimuth_BS/28 -> RadarSensor:4.OBJ_S_Azimuth_28/1  "<OBJ_S_Azimuth_28>"
  Bus Selector:RadarSensor:4_OBJ_S_Azimuth_BS/29 -> RadarSensor:4.OBJ_S_Azimuth_29/1  "<OBJ_S_Azimuth_29>"
  Bus Selector:RadarSensor:4_OBJ_S_Azimuth_BS/30 -> RadarSensor:4.OBJ_S_Azimuth_30/1  "<OBJ_S_Azimuth_30>"
  Bus Selector:RadarSensor:4_OBJ_S_Azimuth_BS/31 -> RadarSensor:4.OBJ_S_Azimuth_31/1  "<OBJ_S_Azimuth_31>"
  Bus Selector:RadarSensor:4_OBJ_S_Azimuth_BS/32 -> RadarSensor:4.OBJ_S_Azimuth_32/1  "<OBJ_S_Azimuth_32>"
  Bus Selector:RadarSensor:4_OBJ_S_Azimuth_BS/33 -> RadarSensor:4.OBJ_S_Azimuth_33/1  "<OBJ_S_Azimuth_33>"
  Bus Selector:RadarSensor:4_OBJ_S_Azimuth_BS/34 -> RadarSensor:4.OBJ_S_Azimuth_34/1  "<OBJ_S_Azimuth_34>"
  Bus Selector:RadarSensor:4_OBJ_S_Azimuth_BS/35 -> RadarSensor:4.OBJ_S_Azimuth_35/1  "<OBJ_S_Azimuth_35>"
  Bus Selector:RadarSensor:4_OBJ_S_Azimuth_BS/36 -> RadarSensor:4.OBJ_S_Azimuth_36/1  "<OBJ_S_Azimuth_36>"
  Bus Selector:RadarSensor:4_OBJ_S_Azimuth_BS/37 -> RadarSensor:4.OBJ_S_Azimuth_37/1  "<OBJ_S_Azimuth_37>"
  Bus Selector:RadarSensor:4_OBJ_S_Azimuth_BS/38 -> RadarSensor:4.OBJ_S_Azimuth_38/1  "<OBJ_S_Azimuth_38>"
  Bus Selector:RadarSensor:4_OBJ_S_Azimuth_BS/39 -> RadarSensor:4.OBJ_S_Azimuth_39/1  "<OBJ_S_Azimuth_39>"
  Bus Selector:RadarSensor:4_OBJ_S_Azimuth_BS/40 -> RadarSensor:4.OBJ_S_Azimuth_40/1  "<OBJ_S_Azimuth_40>"
  Bus Selector:RadarSensor:4_OBJ_S_Azimuth_BS/41 -> RadarSensor:4.OBJ_S_Azimuth_41/1  "<OBJ_S_Azimuth_41>"
  Bus Selector:RadarSensor:4_OBJ_S_Azimuth_BS/42 -> RadarSensor:4.OBJ_S_Azimuth_42/1  "<OBJ_S_Azimuth_42>"
  Bus Selector:RadarSensor:4_OBJ_S_Azimuth_BS/43 -> RadarSensor:4.OBJ_S_Azimuth_43/1  "<OBJ_S_Azimuth_43>"
  Bus Selector:RadarSensor:4_OBJ_S_Azimuth_BS/44 -> RadarSensor:4.OBJ_S_Azimuth_44/1  "<OBJ_S_Azimuth_44>"
  Bus Selector:RadarSensor:4_OBJ_S_Azimuth_BS/45 -> RadarSensor:4.OBJ_S_Azimuth_45/1  "<OBJ_S_Azimuth_45>"
  Bus Selector:RadarSensor:4_OBJ_S_Azimuth_BS/46 -> RadarSensor:4.OBJ_S_Azimuth_46/1  "<OBJ_S_Azimuth_46>"
  Bus Selector:RadarSensor:4_OBJ_S_Azimuth_BS/47 -> RadarSensor:4.OBJ_S_Azimuth_47/1  "<OBJ_S_Azimuth_47>"
  Bus Selector:RadarSensor:4_OBJ_S_Azimuth_BS/48 -> RadarSensor:4.OBJ_S_Azimuth_48/1  "<OBJ_S_Azimuth_48>"
  Bus Selector:RadarSensor:4_OBJ_S_Azimuth_BS/49 -> RadarSensor:4.OBJ_S_Azimuth_49/1  "<OBJ_S_Azimuth_49>"
  Bus Selector:RadarSensor:4_OBJ_S_Azimuth_BS/50 -> RadarSensor:4.OBJ_S_Azimuth_50/1  "<OBJ_S_Azimuth_50>"
  Bus Selector:RadarSensor:4_OBJ_S_Azimuth_BS/51 -> RadarSensor:4.OBJ_S_Azimuth_51/1  "<OBJ_S_Azimuth_51>"
  Bus Selector:RadarSensor:4_OBJ_S_Azimuth_BS/52 -> RadarSensor:4.OBJ_S_Azimuth_52/1  "<OBJ_S_Azimuth_52>"
  Bus Selector:RadarSensor:4_OBJ_S_Azimuth_BS/53 -> RadarSensor:4.OBJ_S_Azimuth_53/1  "<OBJ_S_Azimuth_53>"
  Bus Selector:RadarSensor:4_OBJ_S_Azimuth_BS/54 -> RadarSensor:4.OBJ_S_Azimuth_54/1  "<OBJ_S_Azimuth_54>"
  Bus Selector:RadarSensor:4_OBJ_S_Azimuth_BS/55 -> RadarSensor:4.OBJ_S_Azimuth_55/1  "<OBJ_S_Azimuth_55>"
  Bus Selector:RadarSensor:4_OBJ_S_Azimuth_BS/56 -> RadarSensor:4.OBJ_S_Azimuth_56/1  "<OBJ_S_Azimuth_56>"
  Bus Selector:RadarSensor:4_OBJ_S_Azimuth_BS/57 -> RadarSensor:4.OBJ_S_Azimuth_57/1  "<OBJ_S_Azimuth_57>"
  Bus Selector:RadarSensor:4_OBJ_S_Azimuth_BS/58 -> RadarSensor:4.OBJ_S_Azimuth_58/1  "<OBJ_S_Azimuth_58>"
  Bus Selector:RadarSensor:4_OBJ_S_Azimuth_BS/59 -> RadarSensor:4.OBJ_S_Azimuth_59/1  "<OBJ_S_Azimuth_59>"
  Bus Selector:RadarSensor:4_OBJ_S_Azimuth_BS/60 -> RadarSensor:4.OBJ_S_Azimuth_60/1  "<OBJ_S_Azimuth_60>"
  Bus Selector:RadarSensor:4_OBJ_S_Azimuth_BS/61 -> RadarSensor:4.OBJ_S_Azimuth_61/1  "<OBJ_S_Azimuth_61>"
  Bus Selector:RadarSensor:4_OBJ_S_Azimuth_BS/62 -> RadarSensor:4.OBJ_S_Azimuth_62/1  "<OBJ_S_Azimuth_62>"
  Bus Selector:RadarSensor:4_OBJ_S_Azimuth_BS/63 -> RadarSensor:4.OBJ_S_Azimuth_63/1  "<OBJ_S_Azimuth_63>"
  Bus Selector:RadarSensor:4_OBJ_S_Azimuth_BS/64 -> RadarSensor:4.OBJ_S_Azimuth_64/1  "<OBJ_S_Azimuth_64>"
  Bus Selector:RadarSensor:4_OBJ_S_Elevation_BS/1 -> RadarSensor:4.OBJ_S_Elevation_1/1  "<OBJ_S_Elevation_1>"
  Bus Selector:RadarSensor:4_OBJ_S_Elevation_BS/2 -> RadarSensor:4.OBJ_S_Elevation_2/1  "<OBJ_S_Elevation_2>"
  Bus Selector:RadarSensor:4_OBJ_S_Elevation_BS/3 -> RadarSensor:4.OBJ_S_Elevation_3/1  "<OBJ_S_Elevation_3>"
  Bus Selector:RadarSensor:4_OBJ_S_Elevation_BS/4 -> RadarSensor:4.OBJ_S_Elevation_4/1  "<OBJ_S_Elevation_4>"
  Bus Selector:RadarSensor:4_OBJ_S_Elevation_BS/5 -> RadarSensor:4.OBJ_S_Elevation_5/1  "<OBJ_S_Elevation_5>"
  Bus Selector:RadarSensor:4_OBJ_S_Elevation_BS/6 -> RadarSensor:4.OBJ_S_Elevation_6/1  "<OBJ_S_Elevation_6>"
  Bus Selector:RadarSensor:4_OBJ_S_Elevation_BS/7 -> RadarSensor:4.OBJ_S_Elevation_7/1  "<OBJ_S_Elevation_7>"
  Bus Selector:RadarSensor:4_OBJ_S_Elevation_BS/8 -> RadarSensor:4.OBJ_S_Elevation_8/1  "<OBJ_S_Elevation_8>"
  Bus Selector:RadarSensor:4_OBJ_S_Elevation_BS/9 -> RadarSensor:4.OBJ_S_Elevation_9/1  "<OBJ_S_Elevation_9>"
  Bus Selector:RadarSensor:4_OBJ_S_Elevation_BS/10 -> RadarSensor:4.OBJ_S_Elevation_10/1  "<OBJ_S_Elevation_10>"
  Bus Selector:RadarSensor:4_OBJ_S_Elevation_BS/11 -> RadarSensor:4.OBJ_S_Elevation_11/1  "<OBJ_S_Elevation_11>"
  Bus Selector:RadarSensor:4_OBJ_S_Elevation_BS/12 -> RadarSensor:4.OBJ_S_Elevation_12/1  "<OBJ_S_Elevation_12>"
  Bus Selector:RadarSensor:4_OBJ_S_Elevation_BS/13 -> RadarSensor:4.OBJ_S_Elevation_13/1  "<OBJ_S_Elevation_13>"
  Bus Selector:RadarSensor:4_OBJ_S_Elevation_BS/14 -> RadarSensor:4.OBJ_S_Elevation_14/1  "<OBJ_S_Elevation_14>"
  Bus Selector:RadarSensor:4_OBJ_S_Elevation_BS/15 -> RadarSensor:4.OBJ_S_Elevation_15/1  "<OBJ_S_Elevation_15>"
  Bus Selector:RadarSensor:4_OBJ_S_Elevation_BS/16 -> RadarSensor:4.OBJ_S_Elevation_16/1  "<OBJ_S_Elevation_16>"
  Bus Selector:RadarSensor:4_OBJ_S_Elevation_BS/17 -> RadarSensor:4.OBJ_S_Elevation_17/1  "<OBJ_S_Elevation_17>"
  Bus Selector:RadarSensor:4_OBJ_S_Elevation_BS/18 -> RadarSensor:4.OBJ_S_Elevation_18/1  "<OBJ_S_Elevation_18>"
  Bus Selector:RadarSensor:4_OBJ_S_Elevation_BS/19 -> RadarSensor:4.OBJ_S_Elevation_19/1  "<OBJ_S_Elevation_19>"
  Bus Selector:RadarSensor:4_OBJ_S_Elevation_BS/20 -> RadarSensor:4.OBJ_S_Elevation_20/1  "<OBJ_S_Elevation_20>"
  Bus Selector:RadarSensor:4_OBJ_S_Elevation_BS/21 -> RadarSensor:4.OBJ_S_Elevation_21/1  "<OBJ_S_Elevation_21>"
  Bus Selector:RadarSensor:4_OBJ_S_Elevation_BS/22 -> RadarSensor:4.OBJ_S_Elevation_22/1  "<OBJ_S_Elevation_22>"
  Bus Selector:RadarSensor:4_OBJ_S_Elevation_BS/23 -> RadarSensor:4.OBJ_S_Elevation_23/1  "<OBJ_S_Elevation_23>"
  Bus Selector:RadarSensor:4_OBJ_S_Elevation_BS/24 -> RadarSensor:4.OBJ_S_Elevation_24/1  "<OBJ_S_Elevation_24>"
  Bus Selector:RadarSensor:4_OBJ_S_Elevation_BS/25 -> RadarSensor:4.OBJ_S_Elevation_25/1  "<OBJ_S_Elevation_25>"
  Bus Selector:RadarSensor:4_OBJ_S_Elevation_BS/26 -> RadarSensor:4.OBJ_S_Elevation_26/1  "<OBJ_S_Elevation_26>"
  Bus Selector:RadarSensor:4_OBJ_S_Elevation_BS/27 -> RadarSensor:4.OBJ_S_Elevation_27/1  "<OBJ_S_Elevation_27>"
  Bus Selector:RadarSensor:4_OBJ_S_Elevation_BS/28 -> RadarSensor:4.OBJ_S_Elevation_28/1  "<OBJ_S_Elevation_28>"
  Bus Selector:RadarSensor:4_OBJ_S_Elevation_BS/29 -> RadarSensor:4.OBJ_S_Elevation_29/1  "<OBJ_S_Elevation_29>"
  Bus Selector:RadarSensor:4_OBJ_S_Elevation_BS/30 -> RadarSensor:4.OBJ_S_Elevation_30/1  "<OBJ_S_Elevation_30>"
  Bus Selector:RadarSensor:4_OBJ_S_Elevation_BS/31 -> RadarSensor:4.OBJ_S_Elevation_31/1  "<OBJ_S_Elevation_31>"
  Bus Selector:RadarSensor:4_OBJ_S_Elevation_BS/32 -> RadarSensor:4.OBJ_S_Elevation_32/1  "<OBJ_S_Elevation_32>"
  Bus Selector:RadarSensor:4_OBJ_S_Elevation_BS/33 -> RadarSensor:4.OBJ_S_Elevation_33/1  "<OBJ_S_Elevation_33>"
  Bus Selector:RadarSensor:4_OBJ_S_Elevation_BS/34 -> RadarSensor:4.OBJ_S_Elevation_34/1  "<OBJ_S_Elevation_34>"
  Bus Selector:RadarSensor:4_OBJ_S_Elevation_BS/35 -> RadarSensor:4.OBJ_S_Elevation_35/1  "<OBJ_S_Elevation_35>"
  Bus Selector:RadarSensor:4_OBJ_S_Elevation_BS/36 -> RadarSensor:4.OBJ_S_Elevation_36/1  "<OBJ_S_Elevation_36>"
  Bus Selector:RadarSensor:4_OBJ_S_Elevation_BS/37 -> RadarSensor:4.OBJ_S_Elevation_37/1  "<OBJ_S_Elevation_37>"
  Bus Selector:RadarSensor:4_OBJ_S_Elevation_BS/38 -> RadarSensor:4.OBJ_S_Elevation_38/1  "<OBJ_S_Elevation_38>"
  Bus Selector:RadarSensor:4_OBJ_S_Elevation_BS/39 -> RadarSensor:4.OBJ_S_Elevation_39/1  "<OBJ_S_Elevation_39>"
  Bus Selector:RadarSensor:4_OBJ_S_Elevation_BS/40 -> RadarSensor:4.OBJ_S_Elevation_40/1  "<OBJ_S_Elevation_40>"
  Bus Selector:RadarSensor:4_OBJ_S_Elevation_BS/41 -> RadarSensor:4.OBJ_S_Elevation_41/1  "<OBJ_S_Elevation_41>"
  Bus Selector:RadarSensor:4_OBJ_S_Elevation_BS/42 -> RadarSensor:4.OBJ_S_Elevation_42/1  "<OBJ_S_Elevation_42>"
  Bus Selector:RadarSensor:4_OBJ_S_Elevation_BS/43 -> RadarSensor:4.OBJ_S_Elevation_43/1  "<OBJ_S_Elevation_43>"
  Bus Selector:RadarSensor:4_OBJ_S_Elevation_BS/44 -> RadarSensor:4.OBJ_S_Elevation_44/1  "<OBJ_S_Elevation_44>"
  Bus Selector:RadarSensor:4_OBJ_S_Elevation_BS/45 -> RadarSensor:4.OBJ_S_Elevation_45/1  "<OBJ_S_Elevation_45>"
  Bus Selector:RadarSensor:4_OBJ_S_Elevation_BS/46 -> RadarSensor:4.OBJ_S_Elevation_46/1  "<OBJ_S_Elevation_46>"
  Bus Selector:RadarSensor:4_OBJ_S_Elevation_BS/47 -> RadarSensor:4.OBJ_S_Elevation_47/1  "<OBJ_S_Elevation_47>"
  Bus Selector:RadarSensor:4_OBJ_S_Elevation_BS/48 -> RadarSensor:4.OBJ_S_Elevation_48/1  "<OBJ_S_Elevation_48>"
  Bus Selector:RadarSensor:4_OBJ_S_Elevation_BS/49 -> RadarSensor:4.OBJ_S_Elevation_49/1  "<OBJ_S_Elevation_49>"
  Bus Selector:RadarSensor:4_OBJ_S_Elevation_BS/50 -> RadarSensor:4.OBJ_S_Elevation_50/1  "<OBJ_S_Elevation_50>"
  Bus Selector:RadarSensor:4_OBJ_S_Elevation_BS/51 -> RadarSensor:4.OBJ_S_Elevation_51/1  "<OBJ_S_Elevation_51>"
  Bus Selector:RadarSensor:4_OBJ_S_Elevation_BS/52 -> RadarSensor:4.OBJ_S_Elevation_52/1  "<OBJ_S_Elevation_52>"
  Bus Selector:RadarSensor:4_OBJ_S_Elevation_BS/53 -> RadarSensor:4.OBJ_S_Elevation_53/1  "<OBJ_S_Elevation_53>"
  Bus Selector:RadarSensor:4_OBJ_S_Elevation_BS/54 -> RadarSensor:4.OBJ_S_Elevation_54/1  "<OBJ_S_Elevation_54>"
  Bus Selector:RadarSensor:4_OBJ_S_Elevation_BS/55 -> RadarSensor:4.OBJ_S_Elevation_55/1  "<OBJ_S_Elevation_55>"
  Bus Selector:RadarSensor:4_OBJ_S_Elevation_BS/56 -> RadarSensor:4.OBJ_S_Elevation_56/1  "<OBJ_S_Elevation_56>"
  Bus Selector:RadarSensor:4_OBJ_S_Elevation_BS/57 -> RadarSensor:4.OBJ_S_Elevation_57/1  "<OBJ_S_Elevation_57>"
  Bus Selector:RadarSensor:4_OBJ_S_Elevation_BS/58 -> RadarSensor:4.OBJ_S_Elevation_58/1  "<OBJ_S_Elevation_58>"
  Bus Selector:RadarSensor:4_OBJ_S_Elevation_BS/59 -> RadarSensor:4.OBJ_S_Elevation_59/1  "<OBJ_S_Elevation_59>"
  Bus Selector:RadarSensor:4_OBJ_S_Elevation_BS/60 -> RadarSensor:4.OBJ_S_Elevation_60/1  "<OBJ_S_Elevation_60>"
  Bus Selector:RadarSensor:4_OBJ_S_Elevation_BS/61 -> RadarSensor:4.OBJ_S_Elevation_61/1  "<OBJ_S_Elevation_61>"
  Bus Selector:RadarSensor:4_OBJ_S_Elevation_BS/62 -> RadarSensor:4.OBJ_S_Elevation_62/1  "<OBJ_S_Elevation_62>"
  Bus Selector:RadarSensor:4_OBJ_S_Elevation_BS/63 -> RadarSensor:4.OBJ_S_Elevation_63/1  "<OBJ_S_Elevation_63>"
  Bus Selector:RadarSensor:4_OBJ_S_Elevation_BS/64 -> RadarSensor:4.OBJ_S_Elevation_64/1  "<OBJ_S_Elevation_64>"
  Bus Selector:RadarSensor:4_OBJ_S_Velocity_BS/1 -> RadarSensor:4.OBJ_S_Velocity_1/1  "<OBJ_S_Velocity_1>"
  Bus Selector:RadarSensor:4_OBJ_S_Velocity_BS/2 -> RadarSensor:4.OBJ_S_Velocity_2/1  "<OBJ_S_Velocity_2>"
  Bus Selector:RadarSensor:4_OBJ_S_Velocity_BS/3 -> RadarSensor:4.OBJ_S_Velocity_3/1  "<OBJ_S_Velocity_3>"
  Bus Selector:RadarSensor:4_OBJ_S_Velocity_BS/4 -> RadarSensor:4.OBJ_S_Velocity_4/1  "<OBJ_S_Velocity_4>"
  Bus Selector:RadarSensor:4_OBJ_S_Velocity_BS/5 -> RadarSensor:4.OBJ_S_Velocity_5/1  "<OBJ_S_Velocity_5>"
  Bus Selector:RadarSensor:4_OBJ_S_Velocity_BS/6 -> RadarSensor:4.OBJ_S_Velocity_6/1  "<OBJ_S_Velocity_6>"
  Bus Selector:RadarSensor:4_OBJ_S_Velocity_BS/7 -> RadarSensor:4.OBJ_S_Velocity_7/1  "<OBJ_S_Velocity_7>"
  Bus Selector:RadarSensor:4_OBJ_S_Velocity_BS/8 -> RadarSensor:4.OBJ_S_Velocity_8/1  "<OBJ_S_Velocity_8>"
  Bus Selector:RadarSensor:4_OBJ_S_Velocity_BS/9 -> RadarSensor:4.OBJ_S_Velocity_9/1  "<OBJ_S_Velocity_9>"
  Bus Selector:RadarSensor:4_OBJ_S_Velocity_BS/10 -> RadarSensor:4.OBJ_S_Velocity_10/1  "<OBJ_S_Velocity_10>"
  Bus Selector:RadarSensor:4_OBJ_S_Velocity_BS/11 -> RadarSensor:4.OBJ_S_Velocity_11/1  "<OBJ_S_Velocity_11>"
  Bus Selector:RadarSensor:4_OBJ_S_Velocity_BS/12 -> RadarSensor:4.OBJ_S_Velocity_12/1  "<OBJ_S_Velocity_12>"
  Bus Selector:RadarSensor:4_OBJ_S_Velocity_BS/13 -> RadarSensor:4.OBJ_S_Velocity_13/1  "<OBJ_S_Velocity_13>"
  Bus Selector:RadarSensor:4_OBJ_S_Velocity_BS/14 -> RadarSensor:4.OBJ_S_Velocity_14/1  "<OBJ_S_Velocity_14>"
  Bus Selector:RadarSensor:4_OBJ_S_Velocity_BS/15 -> RadarSensor:4.OBJ_S_Velocity_15/1  "<OBJ_S_Velocity_15>"
  Bus Selector:RadarSensor:4_OBJ_S_Velocity_BS/16 -> RadarSensor:4.OBJ_S_Velocity_16/1  "<OBJ_S_Velocity_16>"
  Bus Selector:RadarSensor:4_OBJ_S_Velocity_BS/17 -> RadarSensor:4.OBJ_S_Velocity_17/1  "<OBJ_S_Velocity_17>"
  Bus Selector:RadarSensor:4_OBJ_S_Velocity_BS/18 -> RadarSensor:4.OBJ_S_Velocity_18/1  "<OBJ_S_Velocity_18>"
  Bus Selector:RadarSensor:4_OBJ_S_Velocity_BS/19 -> RadarSensor:4.OBJ_S_Velocity_19/1  "<OBJ_S_Velocity_19>"
  Bus Selector:RadarSensor:4_OBJ_S_Velocity_BS/20 -> RadarSensor:4.OBJ_S_Velocity_20/1  "<OBJ_S_Velocity_20>"
  Bus Selector:RadarSensor:4_OBJ_S_Velocity_BS/21 -> RadarSensor:4.OBJ_S_Velocity_21/1  "<OBJ_S_Velocity_21>"
  Bus Selector:RadarSensor:4_OBJ_S_Velocity_BS/22 -> RadarSensor:4.OBJ_S_Velocity_22/1  "<OBJ_S_Velocity_22>"
  Bus Selector:RadarSensor:4_OBJ_S_Velocity_BS/23 -> RadarSensor:4.OBJ_S_Velocity_23/1  "<OBJ_S_Velocity_23>"
  Bus Selector:RadarSensor:4_OBJ_S_Velocity_BS/24 -> RadarSensor:4.OBJ_S_Velocity_24/1  "<OBJ_S_Velocity_24>"
  Bus Selector:RadarSensor:4_OBJ_S_Velocity_BS/25 -> RadarSensor:4.OBJ_S_Velocity_25/1  "<OBJ_S_Velocity_25>"
  Bus Selector:RadarSensor:4_OBJ_S_Velocity_BS/26 -> RadarSensor:4.OBJ_S_Velocity_26/1  "<OBJ_S_Velocity_26>"
  Bus Selector:RadarSensor:4_OBJ_S_Velocity_BS/27 -> RadarSensor:4.OBJ_S_Velocity_27/1  "<OBJ_S_Velocity_27>"
  Bus Selector:RadarSensor:4_OBJ_S_Velocity_BS/28 -> RadarSensor:4.OBJ_S_Velocity_28/1  "<OBJ_S_Velocity_28>"
  Bus Selector:RadarSensor:4_OBJ_S_Velocity_BS/29 -> RadarSensor:4.OBJ_S_Velocity_29/1  "<OBJ_S_Velocity_29>"
  Bus Selector:RadarSensor:4_OBJ_S_Velocity_BS/30 -> RadarSensor:4.OBJ_S_Velocity_30/1  "<OBJ_S_Velocity_30>"
  Bus Selector:RadarSensor:4_OBJ_S_Velocity_BS/31 -> RadarSensor:4.OBJ_S_Velocity_31/1  "<OBJ_S_Velocity_31>"
  Bus Selector:RadarSensor:4_OBJ_S_Velocity_BS/32 -> RadarSensor:4.OBJ_S_Velocity_32/1  "<OBJ_S_Velocity_32>"
  Bus Selector:RadarSensor:4_OBJ_S_Velocity_BS/33 -> RadarSensor:4.OBJ_S_Velocity_33/1  "<OBJ_S_Velocity_33>"
  Bus Selector:RadarSensor:4_OBJ_S_Velocity_BS/34 -> RadarSensor:4.OBJ_S_Velocity_34/1  "<OBJ_S_Velocity_34>"
  Bus Selector:RadarSensor:4_OBJ_S_Velocity_BS/35 -> RadarSensor:4.OBJ_S_Velocity_35/1  "<OBJ_S_Velocity_35>"
  Bus Selector:RadarSensor:4_OBJ_S_Velocity_BS/36 -> RadarSensor:4.OBJ_S_Velocity_36/1  "<OBJ_S_Velocity_36>"
  Bus Selector:RadarSensor:4_OBJ_S_Velocity_BS/37 -> RadarSensor:4.OBJ_S_Velocity_37/1  "<OBJ_S_Velocity_37>"
  Bus Selector:RadarSensor:4_OBJ_S_Velocity_BS/38 -> RadarSensor:4.OBJ_S_Velocity_38/1  "<OBJ_S_Velocity_38>"
  Bus Selector:RadarSensor:4_OBJ_S_Velocity_BS/39 -> RadarSensor:4.OBJ_S_Velocity_39/1  "<OBJ_S_Velocity_39>"
  Bus Selector:RadarSensor:4_OBJ_S_Velocity_BS/40 -> RadarSensor:4.OBJ_S_Velocity_40/1  "<OBJ_S_Velocity_40>"
  Bus Selector:RadarSensor:4_OBJ_S_Velocity_BS/41 -> RadarSensor:4.OBJ_S_Velocity_41/1  "<OBJ_S_Velocity_41>"
  Bus Selector:RadarSensor:4_OBJ_S_Velocity_BS/42 -> RadarSensor:4.OBJ_S_Velocity_42/1  "<OBJ_S_Velocity_42>"
  Bus Selector:RadarSensor:4_OBJ_S_Velocity_BS/43 -> RadarSensor:4.OBJ_S_Velocity_43/1  "<OBJ_S_Velocity_43>"
  Bus Selector:RadarSensor:4_OBJ_S_Velocity_BS/44 -> RadarSensor:4.OBJ_S_Velocity_44/1  "<OBJ_S_Velocity_44>"
  Bus Selector:RadarSensor:4_OBJ_S_Velocity_BS/45 -> RadarSensor:4.OBJ_S_Velocity_45/1  "<OBJ_S_Velocity_45>"
  Bus Selector:RadarSensor:4_OBJ_S_Velocity_BS/46 -> RadarSensor:4.OBJ_S_Velocity_46/1  "<OBJ_S_Velocity_46>"
  Bus Selector:RadarSensor:4_OBJ_S_Velocity_BS/47 -> RadarSensor:4.OBJ_S_Velocity_47/1  "<OBJ_S_Velocity_47>"
  Bus Selector:RadarSensor:4_OBJ_S_Velocity_BS/48 -> RadarSensor:4.OBJ_S_Velocity_48/1  "<OBJ_S_Velocity_48>"
  Bus Selector:RadarSensor:4_OBJ_S_Velocity_BS/49 -> RadarSensor:4.OBJ_S_Velocity_49/1  "<OBJ_S_Velocity_49>"
  Bus Selector:RadarSensor:4_OBJ_S_Velocity_BS/50 -> RadarSensor:4.OBJ_S_Velocity_50/1  "<OBJ_S_Velocity_50>"
  Bus Selector:RadarSensor:4_OBJ_S_Velocity_BS/51 -> RadarSensor:4.OBJ_S_Velocity_51/1  "<OBJ_S_Velocity_51>"
  Bus Selector:RadarSensor:4_OBJ_S_Velocity_BS/52 -> RadarSensor:4.OBJ_S_Velocity_52/1  "<OBJ_S_Velocity_52>"
  Bus Selector:RadarSensor:4_OBJ_S_Velocity_BS/53 -> RadarSensor:4.OBJ_S_Velocity_53/1  "<OBJ_S_Velocity_53>"
  Bus Selector:RadarSensor:4_OBJ_S_Velocity_BS/54 -> RadarSensor:4.OBJ_S_Velocity_54/1  "<OBJ_S_Velocity_54>"
  Bus Selector:RadarSensor:4_OBJ_S_Velocity_BS/55 -> RadarSensor:4.OBJ_S_Velocity_55/1  "<OBJ_S_Velocity_55>"
  Bus Selector:RadarSensor:4_OBJ_S_Velocity_BS/56 -> RadarSensor:4.OBJ_S_Velocity_56/1  "<OBJ_S_Velocity_56>"
  Bus Selector:RadarSensor:4_OBJ_S_Velocity_BS/57 -> RadarSensor:4.OBJ_S_Velocity_57/1  "<OBJ_S_Velocity_57>"
  Bus Selector:RadarSensor:4_OBJ_S_Velocity_BS/58 -> RadarSensor:4.OBJ_S_Velocity_58/1  "<OBJ_S_Velocity_58>"
  Bus Selector:RadarSensor:4_OBJ_S_Velocity_BS/59 -> RadarSensor:4.OBJ_S_Velocity_59/1  "<OBJ_S_Velocity_59>"
  Bus Selector:RadarSensor:4_OBJ_S_Velocity_BS/60 -> RadarSensor:4.OBJ_S_Velocity_60/1  "<OBJ_S_Velocity_60>"
  Bus Selector:RadarSensor:4_OBJ_S_Velocity_BS/61 -> RadarSensor:4.OBJ_S_Velocity_61/1  "<OBJ_S_Velocity_61>"
  Bus Selector:RadarSensor:4_OBJ_S_Velocity_BS/62 -> RadarSensor:4.OBJ_S_Velocity_62/1  "<OBJ_S_Velocity_62>"
  Bus Selector:RadarSensor:4_OBJ_S_Velocity_BS/63 -> RadarSensor:4.OBJ_S_Velocity_63/1  "<OBJ_S_Velocity_63>"
  Bus Selector:RadarSensor:4_OBJ_S_Velocity_BS/64 -> RadarSensor:4.OBJ_S_Velocity_64/1  "<OBJ_S_Velocity_64>"
  Bus Selector:RadarSensor:4_OBJ_S_Range_BS/1 -> RadarSensor:4.OBJ_S_Range_1/1  "<OBJ_S_Range_1>"
  Bus Selector:RadarSensor:4_OBJ_S_Range_BS/2 -> RadarSensor:4.OBJ_S_Range_2/1  "<OBJ_S_Range_2>"
  Bus Selector:RadarSensor:4_OBJ_S_Range_BS/3 -> RadarSensor:4.OBJ_S_Range_3/1  "<OBJ_S_Range_3>"
  Bus Selector:RadarSensor:4_OBJ_S_Range_BS/4 -> RadarSensor:4.OBJ_S_Range_4/1  "<OBJ_S_Range_4>"
  Bus Selector:RadarSensor:4_OBJ_S_Range_BS/5 -> RadarSensor:4.OBJ_S_Range_5/1  "<OBJ_S_Range_5>"
  Bus Selector:RadarSensor:4_OBJ_S_Range_BS/6 -> RadarSensor:4.OBJ_S_Range_6/1  "<OBJ_S_Range_6>"
  Bus Selector:RadarSensor:4_OBJ_S_Range_BS/7 -> RadarSensor:4.OBJ_S_Range_7/1  "<OBJ_S_Range_7>"
  Bus Selector:RadarSensor:4_OBJ_S_Range_BS/8 -> RadarSensor:4.OBJ_S_Range_8/1  "<OBJ_S_Range_8>"
  Bus Selector:RadarSensor:4_OBJ_S_Range_BS/9 -> RadarSensor:4.OBJ_S_Range_9/1  "<OBJ_S_Range_9>"
  Bus Selector:RadarSensor:4_OBJ_S_Range_BS/10 -> RadarSensor:4.OBJ_S_Range_10/1  "<OBJ_S_Range_10>"
  Bus Selector:RadarSensor:4_OBJ_S_Range_BS/11 -> RadarSensor:4.OBJ_S_Range_11/1  "<OBJ_S_Range_11>"
  Bus Selector:RadarSensor:4_OBJ_S_Range_BS/12 -> RadarSensor:4.OBJ_S_Range_12/1  "<OBJ_S_Range_12>"
  Bus Selector:RadarSensor:4_OBJ_S_Range_BS/13 -> RadarSensor:4.OBJ_S_Range_13/1  "<OBJ_S_Range_13>"
  Bus Selector:RadarSensor:4_OBJ_S_Range_BS/14 -> RadarSensor:4.OBJ_S_Range_14/1  "<OBJ_S_Range_14>"
  Bus Selector:RadarSensor:4_OBJ_S_Range_BS/15 -> RadarSensor:4.OBJ_S_Range_15/1  "<OBJ_S_Range_15>"
  Bus Selector:RadarSensor:4_OBJ_S_Range_BS/16 -> RadarSensor:4.OBJ_S_Range_16/1  "<OBJ_S_Range_16>"
  Bus Selector:RadarSensor:4_OBJ_S_Range_BS/17 -> RadarSensor:4.OBJ_S_Range_17/1  "<OBJ_S_Range_17>"
  Bus Selector:RadarSensor:4_OBJ_S_Range_BS/18 -> RadarSensor:4.OBJ_S_Range_18/1  "<OBJ_S_Range_18>"
  Bus Selector:RadarSensor:4_OBJ_S_Range_BS/19 -> RadarSensor:4.OBJ_S_Range_19/1  "<OBJ_S_Range_19>"
  Bus Selector:RadarSensor:4_OBJ_S_Range_BS/20 -> RadarSensor:4.OBJ_S_Range_20/1  "<OBJ_S_Range_20>"
  Bus Selector:RadarSensor:4_OBJ_S_Range_BS/21 -> RadarSensor:4.OBJ_S_Range_21/1  "<OBJ_S_Range_21>"
  Bus Selector:RadarSensor:4_OBJ_S_Range_BS/22 -> RadarSensor:4.OBJ_S_Range_22/1  "<OBJ_S_Range_22>"
  Bus Selector:RadarSensor:4_OBJ_S_Range_BS/23 -> RadarSensor:4.OBJ_S_Range_23/1  "<OBJ_S_Range_23>"
  Bus Selector:RadarSensor:4_OBJ_S_Range_BS/24 -> RadarSensor:4.OBJ_S_Range_24/1  "<OBJ_S_Range_24>"
  Bus Selector:RadarSensor:4_OBJ_S_Range_BS/25 -> RadarSensor:4.OBJ_S_Range_25/1  "<OBJ_S_Range_25>"
  Bus Selector:RadarSensor:4_OBJ_S_Range_BS/26 -> RadarSensor:4.OBJ_S_Range_26/1  "<OBJ_S_Range_26>"
  Bus Selector:RadarSensor:4_OBJ_S_Range_BS/27 -> RadarSensor:4.OBJ_S_Range_27/1  "<OBJ_S_Range_27>"
  Bus Selector:RadarSensor:4_OBJ_S_Range_BS/28 -> RadarSensor:4.OBJ_S_Range_28/1  "<OBJ_S_Range_28>"
  Bus Selector:RadarSensor:4_OBJ_S_Range_BS/29 -> RadarSensor:4.OBJ_S_Range_29/1  "<OBJ_S_Range_29>"
  Bus Selector:RadarSensor:4_OBJ_S_Range_BS/30 -> RadarSensor:4.OBJ_S_Range_30/1  "<OBJ_S_Range_30>"
  Bus Selector:RadarSensor:4_OBJ_S_Range_BS/31 -> RadarSensor:4.OBJ_S_Range_31/1  "<OBJ_S_Range_31>"
  Bus Selector:RadarSensor:4_OBJ_S_Range_BS/32 -> RadarSensor:4.OBJ_S_Range_32/1  "<OBJ_S_Range_32>"
  Bus Selector:RadarSensor:4_OBJ_S_Range_BS/33 -> RadarSensor:4.OBJ_S_Range_33/1  "<OBJ_S_Range_33>"
  Bus Selector:RadarSensor:4_OBJ_S_Range_BS/34 -> RadarSensor:4.OBJ_S_Range_34/1  "<OBJ_S_Range_34>"
  Bus Selector:RadarSensor:4_OBJ_S_Range_BS/35 -> RadarSensor:4.OBJ_S_Range_35/1  "<OBJ_S_Range_35>"
  Bus Selector:RadarSensor:4_OBJ_S_Range_BS/36 -> RadarSensor:4.OBJ_S_Range_36/1  "<OBJ_S_Range_36>"
  Bus Selector:RadarSensor:4_OBJ_S_Range_BS/37 -> RadarSensor:4.OBJ_S_Range_37/1  "<OBJ_S_Range_37>"
  Bus Selector:RadarSensor:4_OBJ_S_Range_BS/38 -> RadarSensor:4.OBJ_S_Range_38/1  "<OBJ_S_Range_38>"
  Bus Selector:RadarSensor:4_OBJ_S_Range_BS/39 -> RadarSensor:4.OBJ_S_Range_39/1  "<OBJ_S_Range_39>"
  Bus Selector:RadarSensor:4_OBJ_S_Range_BS/40 -> RadarSensor:4.OBJ_S_Range_40/1  "<OBJ_S_Range_40>"
  Bus Selector:RadarSensor:4_OBJ_S_Range_BS/41 -> RadarSensor:4.OBJ_S_Range_41/1  "<OBJ_S_Range_41>"
  Bus Selector:RadarSensor:4_OBJ_S_Range_BS/42 -> RadarSensor:4.OBJ_S_Range_42/1  "<OBJ_S_Range_42>"
  Bus Selector:RadarSensor:4_OBJ_S_Range_BS/43 -> RadarSensor:4.OBJ_S_Range_43/1  "<OBJ_S_Range_43>"
  Bus Selector:RadarSensor:4_OBJ_S_Range_BS/44 -> RadarSensor:4.OBJ_S_Range_44/1  "<OBJ_S_Range_44>"
  Bus Selector:RadarSensor:4_OBJ_S_Range_BS/45 -> RadarSensor:4.OBJ_S_Range_45/1  "<OBJ_S_Range_45>"
  Bus Selector:RadarSensor:4_OBJ_S_Range_BS/46 -> RadarSensor:4.OBJ_S_Range_46/1  "<OBJ_S_Range_46>"
  Bus Selector:RadarSensor:4_OBJ_S_Range_BS/47 -> RadarSensor:4.OBJ_S_Range_47/1  "<OBJ_S_Range_47>"
  Bus Selector:RadarSensor:4_OBJ_S_Range_BS/48 -> RadarSensor:4.OBJ_S_Range_48/1  "<OBJ_S_Range_48>"
  Bus Selector:RadarSensor:4_OBJ_S_Range_BS/49 -> RadarSensor:4.OBJ_S_Range_49/1  "<OBJ_S_Range_49>"
  Bus Selector:RadarSensor:4_OBJ_S_Range_BS/50 -> RadarSensor:4.OBJ_S_Range_50/1  "<OBJ_S_Range_50>"
  Bus Selector:RadarSensor:4_OBJ_S_Range_BS/51 -> RadarSensor:4.OBJ_S_Range_51/1  "<OBJ_S_Range_51>"
  Bus Selector:RadarSensor:4_OBJ_S_Range_BS/52 -> RadarSensor:4.OBJ_S_Range_52/1  "<OBJ_S_Range_52>"
  Bus Selector:RadarSensor:4_OBJ_S_Range_BS/53 -> RadarSensor:4.OBJ_S_Range_53/1  "<OBJ_S_Range_53>"
  Bus Selector:RadarSensor:4_OBJ_S_Range_BS/54 -> RadarSensor:4.OBJ_S_Range_54/1  "<OBJ_S_Range_54>"
  Bus Selector:RadarSensor:4_OBJ_S_Range_BS/55 -> RadarSensor:4.OBJ_S_Range_55/1  "<OBJ_S_Range_55>"
  Bus Selector:RadarSensor:4_OBJ_S_Range_BS/56 -> RadarSensor:4.OBJ_S_Range_56/1  "<OBJ_S_Range_56>"
  Bus Selector:RadarSensor:4_OBJ_S_Range_BS/57 -> RadarSensor:4.OBJ_S_Range_57/1  "<OBJ_S_Range_57>"
  Bus Selector:RadarSensor:4_OBJ_S_Range_BS/58 -> RadarSensor:4.OBJ_S_Range_58/1  "<OBJ_S_Range_58>"
  Bus Selector:RadarSensor:4_OBJ_S_Range_BS/59 -> RadarSensor:4.OBJ_S_Range_59/1  "<OBJ_S_Range_59>"
  Bus Selector:RadarSensor:4_OBJ_S_Range_BS/60 -> RadarSensor:4.OBJ_S_Range_60/1  "<OBJ_S_Range_60>"
  Bus Selector:RadarSensor:4_OBJ_S_Range_BS/61 -> RadarSensor:4.OBJ_S_Range_61/1  "<OBJ_S_Range_61>"
  Bus Selector:RadarSensor:4_OBJ_S_Range_BS/62 -> RadarSensor:4.OBJ_S_Range_62/1  "<OBJ_S_Range_62>"
  Bus Selector:RadarSensor:4_OBJ_S_Range_BS/63 -> RadarSensor:4.OBJ_S_Range_63/1  "<OBJ_S_Range_63>"
  Bus Selector:RadarSensor:4_OBJ_S_Range_BS/64 -> RadarSensor:4.OBJ_S_Range_64/1  "<OBJ_S_Range_64>"
  Bus Selector:RadarSensor:4_OBJ_RCS_BS/1 -> RadarSensor:4.OBJ_RCS_1/1  "<OBJ_RCS_1>"
  Bus Selector:RadarSensor:4_OBJ_RCS_BS/2 -> RadarSensor:4.OBJ_RCS_2/1  "<OBJ_RCS_2>"
  Bus Selector:RadarSensor:4_OBJ_RCS_BS/3 -> RadarSensor:4.OBJ_RCS_3/1  "<OBJ_RCS_3>"
  Bus Selector:RadarSensor:4_OBJ_RCS_BS/4 -> RadarSensor:4.OBJ_RCS_4/1  "<OBJ_RCS_4>"
